simulink model "aurora_cpu_ch0_ver2_rtxsg"  (R2019b)
(part 2 of 4)

      link override Hardware Config: Controller=Xilinx VC707 Development Platform  Chassis=FlatIO  Slot1_Carrier=<empty>  Slot1_MezzA=<Empty>  Slot1_MezzB=<Empty>  Slot1_MezzC=<Empty>  Slot1_MezzD=<Empty>  Slot1_MezzE=<Empty>  Slot1_MezzF=<Empty>  Slot1_MezzG=<Empty>  Slot1_MezzH=<Empty>  Slot2_Carrier=<empty>  Slot2_MezzA=<unavailable>  Slot2_MezzB=<unavailable>  Slot3_Carrier=<empty>  Slot3_MezzA=<unavailable>  Slot3_MezzB=<unavailable>  Slot4_Carrier=<empty>  Slot4_MezzA=<unavailable>  Slot4_MezzB=<unavailable>  Slot5_Carrier=<empty>  Slot5_MezzA=<unavailable>  Slot5_MezzB=<unavailable>  Slot6_Carrier=<empty>  Slot6_MezzA=<unavailable>  Slot6_MezzB=<unavailable>  Slot7_Carrier=<empty>  Slot7_MezzA=<unavailable>  Slot7_MezzB=<unavailable>  Slot8_Carrier=<empty>  Slot8_MezzA=<unavailable>  Slot8_MezzB=<unavailable>  Slot9_Carrier=<empty>  Slot9_MezzA=<unavailable>  Slot9_MezzB=<unavailable>  Slot10_Carrier=<empty>  Slot10_MezzA=<unavailable>  Slot10_MezzB=<unavailable>  Slot11_Carrier=<empty>  Slot11_MezzA=<unavailable>  Slot11_MezzB=<unavailable>  Slot12_Carrier=<empty>  Slot12_MezzA=<unavailable>  Slot12_MezzB=<unavailable>  Slot13_Carrier=<empty>  Slot13_MezzA=<unavailable>  Slot13_MezzB=<unavailable>  Slot14_Carrier=<empty>  Slot14_MezzA=<unavailable>  Slot14_MezzB=<unavailable>  Slot15_Carrier=<empty>  Slot15_MezzA=<unavailable>  Slot15_MezzB=<unavailable>  Slot16_Carrier=<empty>  Slot16_MezzA=<unavailable>  Slot16_MezzB=<unavailable>  ExpansionSlot1A=<unavailable>  ExpansionSlot1B=<unavailable>  ExpansionSlot1C=<unavailable>  ExpansionSlot1D=<unavailable>  ExpansionSlot1E=<unavailable>  ExpansionSlot1F=<unavailable>  ExpansionSlot1G=<unavailable>  ExpansionSlot1H=<unavailable>  ExpansionSlot2A=<unavailable>  ExpansionSlot2B=<unavailable>  ExpansionSlot3A=<unavailable>  ExpansionSlot3B=<unavailable>  ExpansionSlot4A=<unavailable>  ExpansionSlot4B=<unavailable>  ExpansionSlot5A=<unavailable>  ExpansionSlot5B=<unavailable>  ExpansionSlot6A=<unavailable>  ExpansionSlot6B=<unavailable>  ExpansionSlot7A=<unavailable>  ExpansionSlot7B=<unavailable>  ExpansionSlot8A=<unavailable>  ExpansionSlot8B=<unavailable>  ExpansionSlot9A=<unavailable>  ExpansionSlot9B=<unavailable>  ExpansionSlot10A=<unavailable>  ExpansionSlot10B=<unavailable>  ExpansionSlot11A=<unavailable>  ExpansionSlot11B=<unavailable>  ExpansionSlot12A=<unavailable>  ExpansionSlot12B=<unavailable>  ExpansionSlot13A=<unavailable>  ExpansionSlot13B=<unavailable>  ExpansionSlot14A=<unavailable>  ExpansionSlot14B=<unavailable>  ExpansionSlot15A=<unavailable>  ExpansionSlot15B=<unavailable>  ExpansionSlot16A=<unavailable>  ExpansionSlot16B=<unavailable>  Slot_DV_16A="{\"dv_16A\":{\"ch0\":{\"PauseBehavior\":\"0\",\"IdleBehavior\":\"0\",\"DefaultValueReg\":\"0\"},\"ch1\":{\"PauseBehavior\":\"0\",\"IdleBehavior\":\"0\",\"DefaultValueReg\":\"0\"},\"ch2\":{\"PauseBehavior\":\"0\",\"IdleBehavior\":\"0\",\"DefaultValueReg\":\"0\"},\"ch3\":{\"PauseBehavior\":\"0\",\"IdleBehavior\":\"0\",\"DefaultValueReg\":\"0\"},\"ch4\":{\"PauseBehavior\":\"0\",\"IdleBehavior\":\"0\",\"DefaultValueReg\":\"0\"},\"ch5\":{\"PauseBehavior\":\"0\",\"IdleBehavior\":\"0\",\"DefaultValueReg\":\"0\"},\"ch6\":{\"PauseBehavior\":\"0\",\"IdleBehavior\":\"0\",\"DefaultValueReg\":\"0\"},\"ch7\":{\"PauseBehavior\":\"0\",\"IdleBehavior\":\"0\",\"DefaultValueReg\":\"0\"},\"ch8\":{\"PauseBehavior\":\"0\",\"IdleBehavior\":\"0\",\"DefaultValueReg\":\"0\"},\"ch9\":{\"PauseBehavior\":\"0\",\"IdleBehavior\":\"0\",\"DefaultValueReg\":\"0\"},\"ch10\":{\"PauseBehavior\":\"0\",\"IdleBehavior\":\"0\",\"DefaultValueReg\":\"0\"},\"ch11\":{\"PauseBehavior\":\"0\",\"IdleBehavior\":\"0\",\"DefaultValueReg\":\"0\"},\"ch12\":{\"PauseBehavior\":\"0\",\"IdleBehavior\":\"0\",\"DefaultValueReg\":\"0\"},\"ch13\":{\"PauseBehavior\":\"0\",\"IdleBehavior\":\"0\",\"DefaultValueReg\":\"0\"},\"ch14\":{\"PauseBehavior\":\"0\",\"IdleBehavior\":\"0\",\"DefaultValueReg\":\"0\"},\"ch15\":{\"PauseBehavior\":\"0\",\"IdleBehavior\":\"0\",\"DefaultValueReg\":\"0\"},\"ch16\":{\"PauseBehavior\":\"0\",\"IdleBehavior\":\"0\",\"DefaultValueReg\":\"0\"},\"ch17\":{\"PauseBehavior\":\"0\",\"IdleBehavior\":\"0\",\"DefaultValueReg\":\"0\"},\"ch18\":{\"PauseBehavior\":\"0\",\"IdleBehavior\":\"0\",\"DefaultValueReg\":\"0\"},\"ch19\":{\"PauseBehavior\":\"0\",\"IdleBehavior\":\"0\",\"DefaultValueReg\":\"0\"},\"ch20\":{\"PauseBehavior\":\"0\",\"IdleBehavior\":\"0\",\"DefaultValueReg\":\"0\"},\"ch21\":{\"PauseBehavior\":\"0\",\"IdleBehavior\":\"0\",\"DefaultValueReg\":\"0\"},\"ch22\":{\"PauseBehavior\":\"0\",\"IdleBehavior\":\"0\",\"DefaultValueReg\":\"0\"},\"ch23\":{\"PauseBehavior\":\"0\",\"IdleBehavior\":\"0\",\"DefaultValueReg\":\"0\"},\"ch24\":{\"PauseBehavior\":\"0\",\"IdleBehavior\":\"0\",\"DefaultValueReg\":\"0\"},\"ch25\":{\"PauseBehavior\":\"0\",\"IdleBehavior\":\"0\",\"DefaultValueReg\":\"0\"},\"ch26\":{\"PauseBehavior\":\"0\",\"IdleBehavior\":\"0\",\"DefaultValueReg\":\"0\"},\"ch27\":{\"PauseBehavior\":\"0\",\"IdleBehavior\":\"0\",\"DefaultValueReg\":\"0\"},\"ch28\":{\"PauseBehavior\":\"0\",\"IdleBehavior\":\"0\",\"DefaultValueReg\":\"0\"},\"ch29\":{\"PauseBehavior\":\"0\",\"IdleBehavior\":\"0\",\"DefaultValueReg\":\"0\"},\"ch30\":{\"PauseBehavior\":\"0\",\"IdleBehavior\":\"0\",\"DefaultValueReg\":\"0\"},\"ch31\":{\"PauseBehavior\":\"0\",\"IdleBehavior\":\"0\",\"DefaultValueReg\":\"0\"}}}"  Slot_DV_16B="{\"dv_16B\":{\"ch0\":{\"PauseBehavior\":\"0\",\"IdleBehavior\":\"0\",\"DefaultValueReg\":\"0\"},\"ch1\":{\"PauseBehavior\":\"0\",\"IdleBehavior\":\"0\",\"DefaultValueReg\":\"0\"},\"ch2\":{\"PauseBehavior\":\"0\",\"IdleBehavior\":\"0\",\"DefaultValueReg\":\"0\"},\"ch3\":{\"PauseBehavior\":\"0\",\"IdleBehavior\":\"0\",\"DefaultValueReg\":\"0\"},\"ch4\":{\"PauseBehavior\":\"0\",\"IdleBehavior\":\"0\",\"DefaultValueReg\":\"0\"},\"ch5\":{\"PauseBehavior\":\"0\",\"IdleBehavior\":\"0\",\"DefaultValueReg\":\"0\"},\"ch6\":{\"PauseBehavior\":\"0\",\"IdleBehavior\":\"0\",\"DefaultValueReg\":\"0\"},\"ch7\":{\"PauseBehavior\":\"0\",\"IdleBehavior\":\"0\",\"DefaultValueReg\":\"0\"},\"ch8\":{\"PauseBehavior\":\"0\",\"IdleBehavior\":\"0\",\"DefaultValueReg\":\"0\"},\"ch9\":{\"PauseBehavior\":\"0\",\"IdleBehavior\":\"0\",\"DefaultValueReg\":\"0\"},\"ch10\":{\"PauseBehavior\":\"0\",\"IdleBehavior\":\"0\",\"DefaultValueReg\":\"0\"},\"ch11\":{\"PauseBehavior\":\"0\",\"IdleBehavior\":\"0\",\"DefaultValueReg\":\"0\"},\"ch12\":{\"PauseBehavior\":\"0\",\"IdleBehavior\":\"0\",\"DefaultValueReg\":\"0\"},\"ch13\":{\"PauseBehavior\":\"0\",\"IdleBehavior\":\"0\",\"DefaultValueReg\":\"0\"},\"ch14\":{\"PauseBehavior\":\"0\",\"IdleBehavior\":\"0\",\"DefaultValueReg\":\"0\"},\"ch15\":{\"PauseBehavior\":\"0\",\"IdleBehavior\":\"0\",\"DefaultValueReg\":\"0\"},\"ch16\":{\"PauseBehavior\":\"0\",\"IdleBehavior\":\"0\",\"DefaultValueReg\":\"0\"},\"ch17\":{\"PauseBehavior\":\"0\",\"IdleBehavior\":\"0\",\"DefaultValueReg\":\"0\"},\"ch18\":{\"PauseBehavior\":\"0\",\"IdleBehavior\":\"0\",\"DefaultValueReg\":\"0\"},\"ch19\":{\"PauseBehavior\":\"0\",\"IdleBehavior\":\"0\",\"DefaultValueReg\":\"0\"},\"ch20\":{\"PauseBehavior\":\"0\",\"IdleBehavior\":\"0\",\"DefaultValueReg\":\"0\"},\"ch21\":{\"PauseBehavior\":\"0\",\"IdleBehavior\":\"0\",\"DefaultValueReg\":\"0\"},\"ch22\":{\"PauseBehavior\":\"0\",\"IdleBehavior\":\"0\",\"DefaultValueReg\":\"0\"},\"ch23\":{\"PauseBehavior\":\"0\",\"IdleBehavior\":\"0\",\"DefaultValueReg\":\"0\"},\"ch24\":{\"PauseBehavior\":\"0\",\"IdleBehavior\":\"0\",\"DefaultValueReg\":\"0\"},\"ch25\":{\"PauseBehavior\":\"0\",\"IdleBehavior\":\"0\",\"DefaultValueReg\":\"0\"},\"ch26\":{\"PauseBehavior\":\"0\",\"IdleBehavior\":\"0\",\"DefaultValueReg\":\"0\"},\"ch27\":{\"PauseBehavior\":\"0\",\"IdleBehavior\":\"0\",\"DefaultValueReg\":\"0\"},\"ch28\":{\"PauseBehavior\":\"0\",\"IdleBehavior\":\"0\",\"DefaultValueReg\":\"0\"},\"ch29\":{\"PauseBehavior\":\"0\",\"IdleBehavior\":\"0\",\"DefaultValueReg\":\"0\"},\"ch30\":{\"PauseBehavior\":\"0\",\"IdleBehavior\":\"0\",\"DefaultValueReg\":\"0\"},\"ch31\":{\"PauseBehavior\":\"0\",\"IdleBehavior\":\"0\",\"DefaultValueReg\":\"0\"}}}"  Expansion_DV_16A="{\"dv_Expansion_16A\":{\"ch0\":{\"PauseBehavior\":\"0\",\"IdleBehavior\":\"0\",\"DefaultValueReg\":\"0\"},\"ch1\":{\"PauseBehavior\":\"0\",\"IdleBehavior\":\"0\",\"DefaultValueReg\":\"0\"},\"ch2\":{\"PauseBehavior\":\"0\",\"IdleBehavior\":\"0\",\"DefaultValueReg\":\"0\"},\"ch3\":{\"PauseBehavior\":\"0\",\"IdleBehavior\":\"0\",\"DefaultValueReg\":\"0\"},\"ch4\":{\"PauseBehavior\":\"0\",\"IdleBehavior\":\"0\",\"DefaultValueReg\":\"0\"},\"ch5\":{\"PauseBehavior\":\"0\",\"IdleBehavior\":\"0\",\"DefaultValueReg\":\"0\"},\"ch6\":{\"PauseBehavior\":\"0\",\"IdleBehavior\":\"0\",\"DefaultValueReg\":\"0\"},\"ch7\":{\"PauseBehavior\":\"0\",\"IdleBehavior\":\"0\",\"DefaultValueReg\":\"0\"},\"ch8\":{\"PauseBehavior\":\"0\",\"IdleBehavior\":\"0\",\"DefaultValueReg\":\"0\"},\"ch9\":{\"PauseBehavior\":\"0\",\"IdleBehavior\":\"0\",\"DefaultValueReg\":\"0\"},\"ch10\":{\"PauseBehavior\":\"0\",\"IdleBehavior\":\"0\",\"DefaultValueReg\":\"0\"},\"ch11\":{\"PauseBehavior\":\"0\",\"IdleBehavior\":\"0\",\"DefaultValueReg\":\"0\"},\"ch12\":{\"PauseBehavior\":\"0\",\"IdleBehavior\":\"0\",\"DefaultValueReg\":\"0\"},\"ch13\":{\"PauseBehavior\":\"0\",\"IdleBehavior\":\"0\",\"DefaultValueReg\":\"0\"},\"ch14\":{\"PauseBehavior\":\"0\",\"IdleBehavior\":\"0\",\"DefaultValueReg\":\"0\"},\"ch15\":{\"PauseBehavior\":\"0\",\"IdleBehavior\":\"0\",\"DefaultValueReg\":\"0\"},\"ch16\":{\"PauseBehavior\":\"0\",\"IdleBehavior\":\"0\",\"DefaultValueReg\":\"0\"},\"ch17\":{\"PauseBehavior\":\"0\",\"IdleBehavior\":\"0\",\"DefaultValueReg\":\"0\"},\"ch18\":{\"PauseBehavior\":\"0\",\"IdleBehavior\":\"0\",\"DefaultValueReg\":\"0\"},\"ch19\":{\"PauseBehavior\":\"0\",\"IdleBehavior\":\"0\",\"DefaultValueReg\":\"0\"},\"ch20\":{\"PauseBehavior\":\"0\",\"IdleBehavior\":\"0\",\"DefaultValueReg\":\"0\"},\"ch21\":{\"PauseBehavior\":\"0\",\"IdleBehavior\":\"0\",\"DefaultValueReg\":\"0\"},\"ch22\":{\"PauseBehavior\":\"0\",\"IdleBehavior\":\"0\",\"DefaultValueReg\":\"0\"},\"ch23\":{\"PauseBehavior\":\"0\",\"IdleBehavior\":\"0\",\"DefaultValueReg\":\"0\"},\"ch24\":{\"PauseBehavior\":\"0\",\"IdleBehavior\":\"0\",\"DefaultValueReg\":\"0\"},\"ch25\":{\"PauseBehavior\":\"0\",\"IdleBehavior\":\"0\",\"DefaultValueReg\":\"0\"},\"ch26\":{\"PauseBehavior\":\"0\",\"IdleBehavior\":\"0\",\"DefaultValueReg\":\"0\"},\"ch27\":{\"PauseBehavior\":\"0\",\"IdleBehavior\":\"0\",\"DefaultValueReg\":\"0\"},\"ch28\":{\"PauseBehavior\":\"0\",\"IdleBehavior\":\"0\",\"DefaultValueReg\":\"0\"},\"ch29\":{\"PauseBehavior\":\"0\",\"IdleBehavior\":\"0\",\"DefaultValueReg\":\"0\"},\"ch30\":{\"PauseBehavior\":\"0\",\"IdleBehavior\":\"0\",\"DefaultValueReg\":\"0\"},\"ch31\":{\"PauseBehavior\":\"0\",\"IdleBehavior\":\"0\",\"DefaultValueReg\":\"0\"}}}"  Expansion_DV_16B="{\"dv_Expansion_16B\":{\"ch0\":{\"PauseBehavior\":\"0\",\"IdleBehavior\":\"0\",\"DefaultValueReg\":\"0\"},\"ch1\":{\"PauseBehavior\":\"0\",\"IdleBehavior\":\"0\",\"DefaultValueReg\":\"0\"},\"ch2\":{\"PauseBehavior\":\"0\",\"IdleBehavior\":\"0\",\"DefaultValueReg\":\"0\"},\"ch3\":{\"PauseBehavior\":\"0\",\"IdleBehavior\":\"0\",\"DefaultValueReg\":\"0\"},\"ch4\":{\"PauseBehavior\":\"0\",\"IdleBehavior\":\"0\",\"DefaultValueReg\":\"0\"},\"ch5\":{\"PauseBehavior\":\"0\",\"IdleBehavior\":\"0\",\"DefaultValueReg\":\"0\"},\"ch6\":{\"PauseBehavior\":\"0\",\"IdleBehavior\":\"0\",\"DefaultValueReg\":\"0\"},\"ch7\":{\"PauseBehavior\":\"0\",\"IdleBehavior\":\"0\",\"DefaultValueReg\":\"0\"},\"ch8\":{\"PauseBehavior\":\"0\",\"IdleBehavior\":\"0\",\"DefaultValueReg\":\"0\"},\"ch9\":{\"PauseBehavior\":\"0\",\"IdleBehavior\":\"0\",\"DefaultValueReg\":\"0\"},\"ch10\":{\"PauseBehavior\":\"0\",\"IdleBehavior\":\"0\",\"DefaultValueReg\":\"0\"},\"ch11\":{\"PauseBehavior\":\"0\",\"IdleBehavior\":\"0\",\"DefaultValueReg\":\"0\"},\"ch12\":{\"PauseBehavior\":\"0\",\"IdleBehavior\":\"0\",\"DefaultValueReg\":\"0\"},\"ch13\":{\"PauseBehavior\":\"0\",\"IdleBehavior\":\"0\",\"DefaultValueReg\":\"0\"},\"ch14\":{\"PauseBehavior\":\"0\",\"IdleBehavior\":\"0\",\"DefaultValueReg\":\"0\"},\"ch15\":{\"PauseBehavior\":\"0\",\"IdleBehavior\":\"0\",\"DefaultValueReg\":\"0\"},\"ch16\":{\"PauseBehavior\":\"0\",\"IdleBehavior\":\"0\",\"DefaultValueReg\":\"0\"},\"ch17\":{\"PauseBehavior\":\"0\",\"IdleBehavior\":\"0\",\"DefaultValueReg\":\"0\"},\"ch18\":{\"PauseBehavior\":\"0\",\"IdleBehavior\":\"0\",\"DefaultValueReg\":\"0\"},\"ch19\":{\"PauseBehavior\":\"0\",\"IdleBehavior\":\"0\",\"DefaultValueReg\":\"0\"},\"ch20\":{\"PauseBehavior\":\"0\",\"IdleBehavior\":\"0\",\"DefaultValueReg\":\"0\"},\"ch21\":{\"PauseBehavior\":\"0\",\"IdleBehavior\":\"0\",\"DefaultValueReg\":\"0\"},\"ch22\":{\"PauseBehavior\":\"0\",\"IdleBehavior\":\"0\",\"DefaultValueReg\":\"0\"},\"ch23\":{\"PauseBehavior\":\"0\",\"IdleBehavior\":\"0\",\"DefaultValueReg\":\"0\"},\"ch24\":{\"PauseBehavior\":\"0\",\"IdleBehavior\":\"0\",\"DefaultValueReg\":\"0\"},\"ch25\":{\"PauseBehavior\":\"0\",\"IdleBehavior\":\"0\",\"DefaultValueReg\":\"0\"},\"ch26\":{\"PauseBehavior\":\"0\",\"IdleBehavior\":\"0\",\"DefaultValueReg\":\"0\"},\"ch27\":{\"PauseBehavior\":\"0\",\"IdleBehavior\":\"0\",\"DefaultValueReg\":\"0\"},\"ch28\":{\"PauseBehavior\":\"0\",\"IdleBehavior\":\"0\",\"DefaultValueReg\":\"0\"},\"ch29\":{\"PauseBehavior\":\"0\",\"IdleBehavior\":\"0\",\"DefaultValueReg\":\"0\"},\"ch30\":{\"PauseBehavior\":\"0\",\"IdleBehavior\":\"0\",\"DefaultValueReg\":\"0\"},\"ch31\":{\"PauseBehavior\":\"0\",\"IdleBehavior\":\"0\",\"DefaultValueReg\":\"0\"}}}"  Slot_DV_15A="{\"dv_15A\":{\"ch0\":{\"PauseBehavior\":\"0\",\"IdleBehavior\":\"0\",\"DefaultValueReg\":\"0\"},\"ch1\":{\"PauseBehavior\":\"0\",\"IdleBehavior\":\"0\",\"DefaultValueReg\":\"0\"},\"ch2\":{\"PauseBehavior\":\"0\",\"IdleBehavior\":\"0\",\"DefaultValueReg\":\"0\"},\"ch3\":{\"PauseBehavior\":\"0\",\"IdleBehavior\":\"0\",\"DefaultValueReg\":\"0\"},\"ch4\":{\"PauseBehavior\":\"0\",\"IdleBehavior\":\"0\",\"DefaultValueReg\":\"0\"},\"ch5\":{\"PauseBehavior\":\"0\",\"IdleBehavior\":\"0\",\"DefaultValueReg\":\"0\"},\"ch6\":{\"PauseBehavior\":\"0\",\"IdleBehavior\":\"0\",\"DefaultValueReg\":\"0\"},\"ch7\":{\"PauseBehavior\":\"0\",\"IdleBehavior\":\"0\",\"DefaultValueReg\":\"0\"},\"ch8\":{\"PauseBehavior\":\"0\",\"IdleBehavior\":\"0\",\"DefaultValueReg\":\"0\"},\"ch9\":{\"PauseBehavior\":\"0\",\"IdleBehavior\":\"0\",\"DefaultValueReg\":\"0\"},\"ch10\":{\"PauseBehavior\":\"0\",\"IdleBehavior\":\"0\",\"DefaultValueReg\":\"0\"},\"ch11\":{\"PauseBehavior\":\"0\",\"IdleBehavior\":\"0\",\"DefaultValueReg\":\"0\"},\"ch12\":{\"PauseBehavior\":\"0\",\"IdleBehavior\":\"0\",\"DefaultValueReg\":\"0\"},\"ch13\":{\"PauseBehavior\":\"0\",\"IdleBehavior\":\"0\",\"DefaultValueReg\":\"0\"},\"ch14\":{\"PauseBehavior\":\"0\",\"IdleBehavior\":\"0\",\"DefaultValueReg\":\"0\"},\"ch15\":{\"PauseBehavior\":\"0\",\"IdleBehavior\":\"0\",\"DefaultValueReg\":\"0\"},\"ch16\":{\"PauseBehavior\":\"0\",\"IdleBehavior\":\"0\",\"DefaultValueReg\":\"0\"},\"ch17\":{\"PauseBehavior\":\"0\",\"IdleBehavior\":\"0\",\"DefaultValueReg\":\"0\"},\"ch18\":{\"PauseBehavior\":\"0\",\"IdleBehavior\":\"0\",\"DefaultValueReg\":\"0\"},\"ch19\":{\"PauseBehavior\":\"0\",\"IdleBehavior\":\"0\",\"DefaultValueReg\":\"0\"},\"ch20\":{\"PauseBehavior\":\"0\",\"IdleBehavior\":\"0\",\"DefaultValueReg\":\"0\"},\"ch21\":{\"PauseBehavior\":\"0\",\"IdleBehavior\":\"0\",\"DefaultValueReg\":\"0\"},\"ch22\":{\"PauseBehavior\":\"0\",\"IdleBehavior\":\"0\",\"DefaultValueReg\":\"0\"},\"ch23\":{\"PauseBehavior\":\"0\",\"IdleBehavior\":\"0\",\"DefaultValueReg\":\"0\"},\"ch24\":{\"PauseBehavior\":\"0\",\"IdleBehavior\":\"0\",\"DefaultValueReg\":\"0\"},\"ch25\":{\"PauseBehavior\":\"0\",\"IdleBehavior\":\"0\",\"DefaultValueReg\":\"0\"},\"ch26\":{\"PauseBehavior\":\"0\",\"IdleBehavior\":\"0\",\"DefaultValueReg\":\"0\"},\"ch27\":{\"PauseBehavior\":\"0\",\"IdleBehavior\":\"0\",\"DefaultValueReg\":\"0\"},\"ch28\":{\"PauseBehavior\":\"0\",\"IdleBehavior\":\"0\",\"DefaultValueReg\":\"0\"},\"ch29\":{\"PauseBehavior\":\"0\",\"IdleBehavior\":\"0\",\"DefaultValueReg\":\"0\"},\"ch30\":{\"PauseBehavior\":\"0\",\"IdleBehavior\":\"0\",\"DefaultValueReg\":\"0\"},\"ch31\":{\"PauseBehavior\":\"0\",\"IdleBehavior\":\"0\",\"DefaultValueReg\":\"0\"}}}"  Slot_DV_15B="{\"dv_15B\":{\"ch0\":{\"PauseBehavior\":\"0\",\"IdleBehavior\":\"0\",\"DefaultValueReg\":\"0\"},\"ch1\":{\"PauseBehavior\":\"0\",\"IdleBehavior\":\"0\",\"DefaultValueReg\":\"0\"},\"ch2\":{\"PauseBehavior\":\"0\",\"IdleBehavior\":\"0\",\"DefaultValueReg\":\"0\"},\"ch3\":{\"PauseBehavior\":\"0\",\"IdleBehavior\":\"0\",\"DefaultValueReg\":\"0\"},\"ch4\":{\"PauseBehavior\":\"0\",\"IdleBehavior\":\"0\",\"DefaultValueReg\":\"0\"},\"ch5\":{\"PauseBehavior\":\"0\",\"IdleBehavior\":\"0\",\"DefaultValueReg\":\"0\"},\"ch6\":{\"PauseBehavior\":\"0\",\"IdleBehavior\":\"0\",\"DefaultValueReg\":\"0\"},\"ch7\":{\"PauseBehavior\":\"0\",\"IdleBehavior\":\"0\",\"DefaultValueReg\":\"0\"},\"ch8\":{\"PauseBehavior\":\"0\",\"IdleBehavior\":\"0\",\"DefaultValueReg\":\"0\"},\"ch9\":{\"PauseBehavior\":\"0\",\"IdleBehavior\":\"0\",\"DefaultValueReg\":\"0\"},\"ch10\":{\"PauseBehavior\":\"0\",\"IdleBehavior\":\"0\",\"DefaultValueReg\":\"0\"},\"ch11\":{\"PauseBehavior\":\"0\",\"IdleBehavior\":\"0\",\"DefaultValueReg\":\"0\"},\"ch12\":{\"PauseBehavior\":\"0\",\"IdleBehavior\":\"0\",\"DefaultValueReg\":\"0\"},\"ch13\":{\"PauseBehavior\":\"0\",\"IdleBehavior\":\"0\",\"DefaultValueReg\":\"0\"},\"ch14\":{\"PauseBehavior\":\"0\",\"IdleBehavior\":\"0\",\"DefaultValueReg\":\"0\"},\"ch15\":{\"PauseBehavior\":\"0\",\"IdleBehavior\":\"0\",\"DefaultValueReg\":\"0\"},\"ch16\":{\"PauseBehavior\":\"0\",\"IdleBehavior\":\"0\",\"DefaultValueReg\":\"0\"},\"ch17\":{\"PauseBehavior\":\"0\",\"IdleBehavior\":\"0\",\"DefaultValueReg\":\"0\"},\"ch18\":{\"PauseBehavior\":\"0\",\"IdleBehavior\":\"0\",\"DefaultValueReg\":\"0\"},\"ch19\":{\"PauseBehavior\":\"0\",\"IdleBehavior\":\"0\",\"DefaultValueReg\":\"0\"},\"ch20\":{\"PauseBehavior\":\"0\",\"IdleBehavior\":\"0\",\"DefaultValueReg\":\"0\"},\"ch21\":{\"PauseBehavior\":\"0\",\"IdleBehavior\":\"0\",\"DefaultValueReg\":\"0\"},\"ch22\":{\"PauseBehavior\":\"0\",\"IdleBehavior\":\"0\",\"DefaultValueReg\":\"0\"},\"ch23\":{\"PauseBehavior\":\"0\",\"IdleBehavior\":\"0\",\"DefaultValueReg\":\"0\"},\"ch24\":{\"PauseBehavior\":\"0\",\"IdleBehavior\":\"0\",\"DefaultValueReg\":\"0\"},\"ch25\":{\"PauseBehavior\":\"0\",\"IdleBehavior\":\"0\",\"DefaultValueReg\":\"0\"},\"ch26\":{\"PauseBehavior\":\"0\",\"IdleBehavior\":\"0\",\"DefaultValueReg\":\"0\"},\"ch27\":{\"PauseBehavior\":\"0\",\"IdleBehavior\":\"0\",\"DefaultValueReg\":\"0\"},\"ch28\":{\"PauseBehavior\":\"0\",\"IdleBehavior\":\"0\",\"DefaultValueReg\":\"0\"},\"ch29\":{\"PauseBehavior\":\"0\",\"IdleBehavior\":\"0\",\"DefaultValueReg\":\"0\"},\"ch30\":{\"PauseBehavior\":\"0\",\"IdleBehavior\":\"0\",\"DefaultValueReg\":\"0\"},\"ch31\":{\"PauseBehavior\":\"0\",\"IdleBehavior\":\"0\",\"DefaultValueReg\":\"0\"}}}"  Expansion_DV_15A="{\"dv_Expansion_15A\":{\"ch0\":{\"PauseBehavior\":\"0\",\"IdleBehavior\":\"0\",\"DefaultValueReg\":\"0\"},\"ch1\":{\"PauseBehavior\":\"0\",\"IdleBehavior\":\"0\",\"DefaultValueReg\":\"0\"},\"ch2\":{\"PauseBehavior\":\"0\",\"IdleBehavior\":\"0\",\"DefaultValueReg\":\"0\"},\"ch3\":{\"PauseBehavior\":\"0\",\"IdleBehavior\":\"0\",\"DefaultValueReg\":\"0\"},\"ch4\":{\"PauseBehavior\":\"0\",\"IdleBehavior\":\"0\",\"DefaultValueReg\":\"0\"},\"ch5\":{\"PauseBehavior\":\"0\",\"IdleBehavior\":\"0\",\"DefaultValueReg\":\"0\"},\"ch6\":{\"PauseBehavior\":\"0\",\"IdleBehavior\":\"0\",\"DefaultValueReg\":\"0\"},\"ch7\":{\"PauseBehavior\":\"0\",\"IdleBehavior\":\"0\",\"DefaultValueReg\":\"0\"},\"ch8\":{\"PauseBehavior\":\"0\",\"IdleBehavior\":\"0\",\"DefaultValueReg\":\"0\"},\"ch9\":{\"PauseBehavior\":\"0\",\"IdleBehavior\":\"0\",\"DefaultValueReg\":\"0\"},\"ch10\":{\"PauseBehavior\":\"0\",\"IdleBehavior\":\"0\",\"DefaultValueReg\":\"0\"},\"ch11\":{\"PauseBehavior\":\"0\",\"IdleBehavior\":\"0\",\"DefaultValueReg\":\"0\"},\"ch12\":{\"PauseBehavior\":\"0\",\"IdleBehavior\":\"0\",\"DefaultValueReg\":\"0\"},\"ch13\":{\"PauseBehavior\":\"0\",\"IdleBehavior\":\"0\",\"DefaultValueReg\":\"0\"},\"ch14\":{\"PauseBehavior\":\"0\",\"IdleBehavior\":\"0\",\"DefaultValueReg\":\"0\"},\"ch15\":{\"PauseBehavior\":\"0\",\"IdleBehavior\":\"0\",\"DefaultValueReg\":\"0\"},\"ch16\":{\"PauseBehavior\":\"0\",\"IdleBehavior\":\"0\",\"DefaultValueReg\":\"0\"},\"ch17\":{\"PauseBehavior\":\"0\",\"IdleBehavior\":\"0\",\"DefaultValueReg\":\"0\"},\"ch18\":{\"PauseBehavior\":\"0\",\"IdleBehavior\":\"0\",\"DefaultValueReg\":\"0\"},\"ch19\":{\"PauseBehavior\":\"0\",\"IdleBehavior\":\"0\",\"DefaultValueReg\":\"0\"},\"ch20\":{\"PauseBehavior\":\"0\",\"IdleBehavior\":\"0\",\"DefaultValueReg\":\"0\"},\"ch21\":{\"PauseBehavior\":\"0\",\"IdleBehavior\":\"0\",\"DefaultValueReg\":\"0\"},\"ch22\":{\"PauseBehavior\":\"0\",\"IdleBehavior\":\"0\",\"DefaultValueReg\":\"0\"},\"ch23\":{\"PauseBehavior\":\"0\",\"IdleBehavior\":\"0\",\"DefaultValueReg\":\"0\"},\"ch24\":{\"PauseBehavior\":\"0\",\"IdleBehavior\":\"0\",\"DefaultValueReg\":\"0\"},\"ch25\":{\"PauseBehavior\":\"0\",\"IdleBehavior\":\"0\",\"DefaultValueReg\":\"0\"},\"ch26\":{\"PauseBehavior\":\"0\",\"IdleBehavior\":\"0\",\"DefaultValueReg\":\"0\"},\"ch27\":{\"PauseBehavior\":\"0\",\"IdleBehavior\":\"0\",\"DefaultValueReg\":\"0\"},\"ch28\":{\"PauseBehavior\":\"0\",\"IdleBehavior\":\"0\",\"DefaultValueReg\":\"0\"},\"ch29\":{\"PauseBehavior\":\"0\",\"IdleBehavior\":\"0\",\"DefaultValueReg\":\"0\"},\"ch30\":{\"PauseBehavior\":\"0\",\"IdleBehavior\":\"0\",\"DefaultValueReg\":\"0\"},\"ch31\":{\"PauseBehavior\":\"0\",\"IdleBehavior\":\"0\",\"DefaultValueReg\":\"0\"}}}"  Expansion_DV_15B="{\"dv_Expansion_15B\":{\"ch0\":{\"PauseBehavior\":\"0\",\"IdleBehavior\":\"0\",\"DefaultValueReg\":\"0\"},\"ch1\":{\"PauseBehavior\":\"0\",\"IdleBehavior\":\"0\",\"DefaultValueReg\":\"0\"},\"ch2\":{\"PauseBehavior\":\"0\",\"IdleBehavior\":\"0\",\"DefaultValueReg\":\"0\"},\"ch3\":{\"PauseBehavior\":\"0\",\"IdleBehavior\":\"0\",\"DefaultValueReg\":\"0\"},\"ch4\":{\"PauseBehavior\":\"0\",\"IdleBehavior\":\"0\",\"DefaultValueReg\":\"0\"},\"ch5\":{\"PauseBehavior\":\"0\",\"IdleBehavior\":\"0\",\"DefaultValueReg\":\"0\"},\"ch6\":{\"PauseBehavior\":\"0\",\"IdleBehavior\":\"0\",\"DefaultValueReg\":\"0\"},\"ch7\":{\"PauseBehavior\":\"0\",\"IdleBehavior\":\"0\",\"DefaultValueReg\":\"0\"},\"ch8\":{\"PauseBehavior\":\"0\",\"IdleBehavior\":\"0\",\"DefaultValueReg\":\"0\"},\"ch9\":{\"PauseBehavior\":\"0\",\"IdleBehavior\":\"0\",\"DefaultValueReg\":\"0\"},\"ch10\":{\"PauseBehavior\":\"0\",\"IdleBehavior\":\"0\",\"DefaultValueReg\":\"0\"},\"ch11\":{\"PauseBehavior\":\"0\",\"IdleBehavior\":\"0\",\"DefaultValueReg\":\"0\"},\"ch12\":{\"PauseBehavior\":\"0\",\"IdleBehavior\":\"0\",\"DefaultValueReg\":\"0\"},\"ch13\":{\"PauseBehavior\":\"0\",\"IdleBehavior\":\"0\",\"DefaultValueReg\":\"0\"},\"ch14\":{\"PauseBehavior\":\"0\",\"IdleBehavior\":\"0\",\"DefaultValueReg\":\"0\"},\"ch15\":{\"PauseBehavior\":\"0\",\"IdleBehavior\":\"0\",\"DefaultValueReg\":\"0\"},\"ch16\":{\"PauseBehavior\":\"0\",\"IdleBehavior\":\"0\",\"DefaultValueReg\":\"0\"},\"ch17\":{\"PauseBehavior\":\"0\",\"IdleBehavior\":\"0\",\"DefaultValueReg\":\"0\"},\"ch18\":{\"PauseBehavior\":\"0\",\"IdleBehavior\":\"0\",\"DefaultValueReg\":\"0\"},\"ch19\":{\"PauseBehavior\":\"0\",\"IdleBehavior\":\"0\",\"DefaultValueReg\":\"0\"},\"ch20\":{\"PauseBehavior\":\"0\",\"IdleBehavior\":\"0\",\"DefaultValueReg\":\"0\"},\"ch21\":{\"PauseBehavior\":\"0\",\"IdleBehavior\":\"0\",\"DefaultValueReg\":\"0\"},\"ch22\":{\"PauseBehavior\":\"0\",\"IdleBehavior\":\"0\",\"DefaultValueReg\":\"0\"},\"ch23\":{\"PauseBehavior\":\"0\",\"IdleBehavior\":\"0\",\"DefaultValueReg\":\"0\"},\"ch24\":{\"PauseBehavior\":\"0\",\"IdleBehavior\":\"0\",\"DefaultValueReg\":\"0\"},\"ch25\":{\"PauseBehavior\":\"0\",\"IdleBehavior\":\"0\",\"DefaultValueReg\":\"0\"},\"ch26\":{\"PauseBehavior\":\"0\",\"IdleBehavior\":\"0\",\"DefaultValueReg\":\"0\"},\"ch27\":{\"PauseBehavior\":\"0\",\"IdleBehavior\":\"0\",\"DefaultValueReg\":\"0\"},\"ch28\":{\"PauseBehavior\":\"0\",\"IdleBehavior\":\"0\",\"DefaultValueReg\":\"0\"},\"ch29\":{\"PauseBehavior\":\"0\",\"IdleBehavior\":\"0\",\"DefaultValueReg\":\"0\"},\"ch30\":{\"PauseBehavior\":\"0\",\"IdleBehavior\":\"0\",\"DefaultValueReg\":\"0\"},\"ch31\":{\"PauseBehavior\":\"0\",\"IdleBehavior\":\"0\",\"DefaultValueReg\":\"0\"}}}"  Slot_DV_14A="{\"dv_14A\":{\"ch0\":{\"PauseBehavior\":\"0\",\"IdleBehavior\":\"0\",\"DefaultValueReg\":\"0\"},\"ch1\":{\"PauseBehavior\":\"0\",\"IdleBehavior\":\"0\",\"DefaultValueReg\":\"0\"},\"ch2\":{\"PauseBehavior\":\"0\",\"IdleBehavior\":\"0\",\"DefaultValueReg\":\"0\"},\"ch3\":{\"PauseBehavior\":\"0\",\"IdleBehavior\":\"0\",\"DefaultValueReg\":\"0\"},\"ch4\":{\"PauseBehavior\":\"0\",\"IdleBehavior\":\"0\",\"DefaultValueReg\":\"0\"},\"ch5\":{\"PauseBehavior\":\"0\",\"IdleBehavior\":\"0\",\"DefaultValueReg\":\"0\"},\"ch6\":{\"PauseBehavior\":\"0\",\"IdleBehavior\":\"0\",\"DefaultValueReg\":\"0\"},\"ch7\":{\"PauseBehavior\":\"0\",\"IdleBehavior\":\"0\",\"DefaultValueReg\":\"0\"},\"ch8\":{\"PauseBehavior\":\"0\",\"IdleBehavior\":\"0\",\"DefaultValueReg\":\"0\"},\"ch9\":{\"PauseBehavior\":\"0\",\"IdleBehavior\":\"0\",\"DefaultValueReg\":\"0\"},\"ch10\":{\"PauseBehavior\":\"0\",\"IdleBehavior\":\"0\",\"DefaultValueReg\":\"0\"},\"ch11\":{\"PauseBehavior\":\"0\",\"IdleBehavior\":\"0\",\"DefaultValueReg\":\"0\"},\"ch12\":{\"PauseBehavior\":\"0\",\"IdleBehavior\":\"0\",\"DefaultValueReg\":\"0\"},\"ch13\":{\"PauseBehavior\":\"0\",\"IdleBehavior\":\"0\",\"DefaultValueReg\":\"0\"},\"ch14\":{\"PauseBehavior\":\"0\",\"IdleBehavior\":\"0\",\"DefaultValueReg\":\"0\"},\"ch15\":{\"PauseBehavior\":\"0\",\"IdleBehavior\":\"0\",\"DefaultValueReg\":\"0\"},\"ch16\":{\"PauseBehavior\":\"0\",\"IdleBehavior\":\"0\",\"DefaultValueReg\":\"0\"},\"ch17\":{\"PauseBehavior\":\"0\",\"IdleBehavior\":\"0\",\"DefaultValueReg\":\"0\"},\"ch18\":{\"PauseBehavior\":\"0\",\"IdleBehavior\":\"0\",\"DefaultValueReg\":\"0\"},\"ch19\":{\"PauseBehavior\":\"0\",\"IdleBehavior\":\"0\",\"DefaultValueReg\":\"0\"},\"ch20\":{\"PauseBehavior\":\"0\",\"IdleBehavior\":\"0\",\"DefaultValueReg\":\"0\"},\"ch21\":{\"PauseBehavior\":\"0\",\"IdleBehavior\":\"0\",\"DefaultValueReg\":\"0\"},\"ch22\":{\"PauseBehavior\":\"0\",\"IdleBehavior\":\"0\",\"DefaultValueReg\":\"0\"},\"ch23\":{\"PauseBehavior\":\"0\",\"IdleBehavior\":\"0\",\"DefaultValueReg\":\"0\"},\"ch24\":{\"PauseBehavior\":\"0\",\"IdleBehavior\":\"0\",\"DefaultValueReg\":\"0\"},\"ch25\":{\"PauseBehavior\":\"0\",\"IdleBehavior\":\"0\",\"DefaultValueReg\":\"0\"},\"ch26\":{\"PauseBehavior\":\"0\",\"IdleBehavior\":\"0\",\"DefaultValueReg\":\"0\"},\"ch27\":{\"PauseBehavior\":\"0\",\"IdleBehavior\":\"0\",\"DefaultValueReg\":\"0\"},\"ch28\":{\"PauseBehavior\":\"0\",\"IdleBehavior\":\"0\",\"DefaultValueReg\":\"0\"},\"ch29\":{\"PauseBehavior\":\"0\",\"IdleBehavior\":\"0\",\"DefaultValueReg\":\"0\"},\"ch30\":{\"PauseBehavior\":\"0\",\"IdleBehavior\":\"0\",\"DefaultValueReg\":\"0\"},\"ch31\":{\"PauseBehavior\":\"0\",\"IdleBehavior\":\"0\",\"DefaultValueReg\":\"0\"}}}"  Slot_DV_14B="{\"dv_14B\":{\"ch0\":{\"PauseBehavior\":\"0\",\"IdleBehavior\":\"0\",\"DefaultValueReg\":\"0\"},\"ch1\":{\"PauseBehavior\":\"0\",\"IdleBehavior\":\"0\",\"DefaultValueReg\":\"0\"},\"ch2\":{\"PauseBehavior\":\"0\",\"IdleBehavior\":\"0\",\"DefaultValueReg\":\"0\"},\"ch3\":{\"PauseBehavior\":\"0\",\"IdleBehavior\":\"0\",\"DefaultValueReg\":\"0\"},\"ch4\":{\"PauseBehavior\":\"0\",\"IdleBehavior\":\"0\",\"DefaultValueReg\":\"0\"},\"ch5\":{\"PauseBehavior\":\"0\",\"IdleBehavior\":\"0\",\"DefaultValueReg\":\"0\"},\"ch6\":{\"PauseBehavior\":\"0\",\"IdleBehavior\":\"0\",\"DefaultValueReg\":\"0\"},\"ch7\":{\"PauseBehavior\":\"0\",\"IdleBehavior\":\"0\",\"DefaultValueReg\":\"0\"},\"ch8\":{\"PauseBehavior\":\"0\",\"IdleBehavior\":\"0\",\"DefaultValueReg\":\"0\"},\"ch9\":{\"PauseBehavior\":\"0\",\"IdleBehavior\":\"0\",\"DefaultValueReg\":\"0\"},\"ch10\":{\"PauseBehavior\":\"0\",\"IdleBehavior\":\"0\",\"DefaultValueReg\":\"0\"},\"ch11\":{\"PauseBehavior\":\"0\",\"IdleBehavior\":\"0\",\"DefaultValueReg\":\"0\"},\"ch12\":{\"PauseBehavior\":\"0\",\"IdleBehavior\":\"0\",\"DefaultValueReg\":\"0\"},\"ch13\":{\"PauseBehavior\":\"0\",\"IdleBehavior\":\"0\",\"DefaultValueReg\":\"0\"},\"ch14\":{\"PauseBehavior\":\"0\",\"IdleBehavior\":\"0\",\"DefaultValueReg\":\"0\"},\"ch15\":{\"PauseBehavior\":\"0\",\"IdleBehavior\":\"0\",\"DefaultValueReg\":\"0\"},\"ch16\":{\"PauseBehavior\":\"0\",\"IdleBehavior\":\"0\",\"DefaultValueReg\":\"0\"},\"ch17\":{\"PauseBehavior\":\"0\",\"IdleBehavior\":\"0\",\"DefaultValueReg\":\"0\"},\"ch18\":{\"PauseBehavior\":\"0\",\"IdleBehavior\":\"0\",\"DefaultValueReg\":\"0\"},\"ch19\":{\"PauseBehavior\":\"0\",\"IdleBehavior\":\"0\",\"DefaultValueReg\":\"0\"},\"ch20\":{\"PauseBehavior\":\"0\",\"IdleBehavior\":\"0\",\"DefaultValueReg\":\"0\"},\"ch21\":{\"PauseBehavior\":\"0\",\"IdleBehavior\":\"0\",\"DefaultValueReg\":\"0\"},\"ch22\":{\"PauseBehavior\":\"0\",\"IdleBehavior\":\"0\",\"DefaultValueReg\":\"0\"},\"ch23\":{\"PauseBehavior\":\"0\",\"IdleBehavior\":\"0\",\"DefaultValueReg\":\"0\"},\"ch24\":{\"PauseBehavior\":\"0\",\"IdleBehavior\":\"0\",\"DefaultValueReg\":\"0\"},\"ch25\":{\"PauseBehavior\":\"0\",\"IdleBehavior\":\"0\",\"DefaultValueReg\":\"0\"},\"ch26\":{\"PauseBehavior\":\"0\",\"IdleBehavior\":\"0\",\"DefaultValueReg\":\"0\"},\"ch27\":{\"PauseBehavior\":\"0\",\"IdleBehavior\":\"0\",\"DefaultValueReg\":\"0\"},\"ch28\":{\"PauseBehavior\":\"0\",\"IdleBehavior\":\"0\",\"DefaultValueReg\":\"0\"},\"ch29\":{\"PauseBehavior\":\"0\",\"IdleBehavior\":\"0\",\"DefaultValueReg\":\"0\"},\"ch30\":{\"PauseBehavior\":\"0\",\"IdleBehavior\":\"0\",\"DefaultValueReg\":\"0\"},\"ch31\":{\"PauseBehavior\":\"0\",\"IdleBehavior\":\"0\",\"DefaultValueReg\":\"0\"}}}"  Expansion_DV_14A="{\"dv_Expansion_14A\":{\"ch0\":{\"PauseBehavior\":\"0\",\"IdleBehavior\":\"0\",\"DefaultValueReg\":\"0\"},\"ch1\":{\"PauseBehavior\":\"0\",\"IdleBehavior\":\"0\",\"DefaultValueReg\":\"0\"},\"ch2\":{\"PauseBehavior\":\"0\",\"IdleBehavior\":\"0\",\"DefaultValueReg\":\"0\"},\"ch3\":{\"PauseBehavior\":\"0\",\"IdleBehavior\":\"0\",\"DefaultValueReg\":\"0\"},\"ch4\":{\"PauseBehavior\":\"0\",\"IdleBehavior\":\"0\",\"DefaultValueReg\":\"0\"},\"ch5\":{\"PauseBehavior\":\"0\",\"IdleBehavior\":\"0\",\"DefaultValueReg\":\"0\"},\"ch6\":{\"PauseBehavior\":\"0\",\"IdleBehavior\":\"0\",\"DefaultValueReg\":\"0\"},\"ch7\":{\"PauseBehavior\":\"0\",\"IdleBehavior\":\"0\",\"DefaultValueReg\":\"0\"},\"ch8\":{\"PauseBehavior\":\"0\",\"IdleBehavior\":\"0\",\"DefaultValueReg\":\"0\"},\"ch9\":{\"PauseBehavior\":\"0\",\"IdleBehavior\":\"0\",\"DefaultValueReg\":\"0\"},\"ch10\":{\"PauseBehavior\":\"0\",\"IdleBehavior\":\"0\",\"DefaultValueReg\":\"0\"},\"ch11\":{\"PauseBehavior\":\"0\",\"IdleBehavior\":\"0\",\"DefaultValueReg\":\"0\"},\"ch12\":{\"PauseBehavior\":\"0\",\"IdleBehavior\":\"0\",\"DefaultValueReg\":\"0\"},\"ch13\":{\"PauseBehavior\":\"0\",\"IdleBehavior\":\"0\",\"DefaultValueReg\":\"0\"},\"ch14\":{\"PauseBehavior\":\"0\",\"IdleBehavior\":\"0\",\"DefaultValueReg\":\"0\"},\"ch15\":{\"PauseBehavior\":\"0\",\"IdleBehavior\":\"0\",\"DefaultValueReg\":\"0\"},\"ch16\":{\"PauseBehavior\":\"0\",\"IdleBehavior\":\"0\",\"DefaultValueReg\":\"0\"},\"ch17\":{\"PauseBehavior\":\"0\",\"IdleBehavior\":\"0\",\"DefaultValueReg\":\"0\"},\"ch18\":{\"PauseBehavior\":\"0\",\"IdleBehavior\":\"0\",\"DefaultValueReg\":\"0\"},\"ch19\":{\"PauseBehavior\":\"0\",\"IdleBehavior\":\"0\",\"DefaultValueReg\":\"0\"},\"ch20\":{\"PauseBehavior\":\"0\",\"IdleBehavior\":\"0\",\"DefaultValueReg\":\"0\"},\"ch21\":{\"PauseBehavior\":\"0\",\"IdleBehavior\":\"0\",\"DefaultValueReg\":\"0\"},\"ch22\":{\"PauseBehavior\":\"0\",\"IdleBehavior\":\"0\",\"DefaultValueReg\":\"0\"},\"ch23\":{\"PauseBehavior\":\"0\",\"IdleBehavior\":\"0\",\"DefaultValueReg\":\"0\"},\"ch24\":{\"PauseBehavior\":\"0\",\"IdleBehavior\":\"0\",\"DefaultValueReg\":\"0\"},\"ch25\":{\"PauseBehavior\":\"0\",\"IdleBehavior\":\"0\",\"DefaultValueReg\":\"0\"},\"ch26\":{\"PauseBehavior\":\"0\",\"IdleBehavior\":\"0\",\"DefaultValueReg\":\"0\"},\"ch27\":{\"PauseBehavior\":\"0\",\"IdleBehavior\":\"0\",\"DefaultValueReg\":\"0\"},\"ch28\":{\"PauseBehavior\":\"0\",\"IdleBehavior\":\"0\",\"DefaultValueReg\":\"0\"},\"ch29\":{\"PauseBehavior\":\"0\",\"IdleBehavior\":\"0\",\"DefaultValueReg\":\"0\"},\"ch30\":{\"PauseBehavior\":\"0\",\"IdleBehavior\":\"0\",\"DefaultValueReg\":\"0\"},\"ch31\":{\"PauseBehavior\":\"0\",\"IdleBehavior\":\"0\",\"DefaultValueReg\":\"0\"}}}"  Expansion_DV_14B="{\"dv_Expansion_14B\":{\"ch0\":{\"PauseBehavior\":\"0\",\"IdleBehavior\":\"0\",\"DefaultValueReg\":\"0\"},\"ch1\":{\"PauseBehavior\":\"0\",\"IdleBehavior\":\"0\",\"DefaultValueReg\":\"0\"},\"ch2\":{\"PauseBehavior\":\"0\",\"IdleBehavior\":\"0\",\"DefaultValueReg\":\"0\"},\"ch3\":{\"PauseBehavior\":\"0\",\"IdleBehavior\":\"0\",\"DefaultValueReg\":\"0\"},\"ch4\":{\"PauseBehavior\":\"0\",\"IdleBehavior\":\"0\",\"DefaultValueReg\":\"0\"},\"ch5\":{\"PauseBehavior\":\"0\",\"IdleBehavior\":\"0\",\"DefaultValueReg\":\"0\"},\"ch6\":{\"PauseBehavior\":\"0\",\"IdleBehavior\":\"0\",\"DefaultValueReg\":\"0\"},\"ch7\":{\"PauseBehavior\":\"0\",\"IdleBehavior\":\"0\",\"DefaultValueReg\":\"0\"},\"ch8\":{\"PauseBehavior\":\"0\",\"IdleBehavior\":\"0\",\"DefaultValueReg\":\"0\"},\"ch9\":{\"PauseBehavior\":\"0\",\"IdleBehavior\":\"0\",\"DefaultValueReg\":\"0\"},\"ch10\":{\"PauseBehavior\":\"0\",\"IdleBehavior\":\"0\",\"DefaultValueReg\":\"0\"},\"ch11\":{\"PauseBehavior\":\"0\",\"IdleBehavior\":\"0\",\"DefaultValueReg\":\"0\"},\"ch12\":{\"PauseBehavior\":\"0\",\"IdleBehavior\":\"0\",\"DefaultValueReg\":\"0\"},\"ch13\":{\"PauseBehavior\":\"0\",\"IdleBehavior\":\"0\",\"DefaultValueReg\":\"0\"},\"ch14\":{\"PauseBehavior\":\"0\",\"IdleBehavior\":\"0\",\"DefaultValueReg\":\"0\"},\"ch15\":{\"PauseBehavior\":\"0\",\"IdleBehavior\":\"0\",\"DefaultValueReg\":\"0\"},\"ch16\":{\"PauseBehavior\":\"0\",\"IdleBehavior\":\"0\",\"DefaultValueReg\":\"0\"},\"ch17\":{\"PauseBehavior\":\"0\",\"IdleBehavior\":\"0\",\"DefaultValueReg\":\"0\"},\"ch18\":{\"PauseBehavior\":\"0\",\"IdleBehavior\":\"0\",\"DefaultValueReg\":\"0\"},\"ch19\":{\"PauseBehavior\":\"0\",\"IdleBehavior\":\"0\",\"DefaultValueReg\":\"0\"},\"ch20\":{\"PauseBehavior\":\"0\",\"IdleBehavior\":\"0\",\"DefaultValueReg\":\"0\"},\"ch21\":{\"PauseBehavior\":\"0\",\"IdleBehavior\":\"0\",\"DefaultValueReg\":\"0\"},\"ch22\":{\"PauseBehavior\":\"0\",\"IdleBehavior\":\"0\",\"DefaultValueReg\":\"0\"},\"ch23\":{\"PauseBehavior\":\"0\",\"IdleBehavior\":\"0\",\"DefaultValueReg\":\"0\"},\"ch24\":{\"PauseBehavior\":\"0\",\"IdleBehavior\":\"0\",\"DefaultValueReg\":\"0\"},\"ch25\":{\"PauseBehavior\":\"0\",\"IdleBehavior\":\"0\",\"DefaultValueReg\":\"0\"},\"ch26\":{\"PauseBehavior\":\"0\",\"IdleBehavior\":\"0\",\"DefaultValueReg\":\"0\"},\"ch27\":{\"PauseBehavior\":\"0\",\"IdleBehavior\":\"0\",\"DefaultValueReg\":\"0\"},\"ch28\":{\"PauseBehavior\":\"0\",\"IdleBehavior\":\"0\",\"DefaultValueReg\":\"0\"},\"ch29\":{\"PauseBehavior\":\"0\",\"IdleBehavior\":\"0\",\"DefaultValueReg\":\"0\"},\"ch30\":{\"PauseBehavior\":\"0\",\"IdleBehavior\":\"0\",\"DefaultValueReg\":\"0\"},\"ch31\":{\"PauseBehavior\":\"0\",\"IdleBehavior\":\"0\",\"DefaultValueReg\":\"0\"}}}"  Slot_DV_13A="{\"dv_13A\":{\"ch0\":{\"PauseBehavior\":\"0\",\"IdleBehavior\":\"0\",\"DefaultValueReg\":\"0\"},\"ch1\":{\"PauseBehavior\":\"0\",\"IdleBehavior\":\"0\",\"DefaultValueReg\":\"0\"},\"ch2\":{\"PauseBehavior\":\"0\",\"IdleBehavior\":\"0\",\"DefaultValueReg\":\"0\"},\"ch3\":{\"PauseBehavior\":\"0\",\"IdleBehavior\":\"0\",\"DefaultValueReg\":\"0\"},\"ch4\":{\"PauseBehavior\":\"0\",\"IdleBehavior\":\"0\",\"DefaultValueReg\":\"0\"},\"ch5\":{\"PauseBehavior\":\"0\",\"IdleBehavior\":\"0\",\"DefaultValueReg\":\"0\"},\"ch6\":{\"PauseBehavior\":\"0\",\"IdleBehavior\":\"0\",\"DefaultValueReg\":\"0\"},\"ch7\":{\"PauseBehavior\":\"0\",\"IdleBehavior\":\"0\",\"DefaultValueReg\":\"0\"},\"ch8\":{\"PauseBehavior\":\"0\",\"IdleBehavior\":\"0\",\"DefaultValueReg\":\"0\"},\"ch9\":{\"PauseBehavior\":\"0\",\"IdleBehavior\":\"0\",\"DefaultValueReg\":\"0\"},\"ch10\":{\"PauseBehavior\":\"0\",\"IdleBehavior\":\"0\",\"DefaultValueReg\":\"0\"},\"ch11\":{\"PauseBehavior\":\"0\",\"IdleBehavior\":\"0\",\"DefaultValueReg\":\"0\"},\"ch12\":{\"PauseBehavior\":\"0\",\"IdleBehavior\":\"0\",\"DefaultValueReg\":\"0\"},\"ch13\":{\"PauseBehavior\":\"0\",\"IdleBehavior\":\"0\",\"DefaultValueReg\":\"0\"},\"ch14\":{\"PauseBehavior\":\"0\",\"IdleBehavior\":\"0\",\"DefaultValueReg\":\"0\"},\"ch15\":{\"PauseBehavior\":\"0\",\"IdleBehavior\":\"0\",\"DefaultValueReg\":\"0\"},\"ch16\":{\"PauseBehavior\":\"0\",\"IdleBehavior\":\"0\",\"DefaultValueReg\":\"0\"},\"ch17\":{\"PauseBehavior\":\"0\",\"IdleBehavior\":\"0\",\"DefaultValueReg\":\"0\"},\"ch18\":{\"PauseBehavior\":\"0\",\"IdleBehavior\":\"0\",\"DefaultValueReg\":\"0\"},\"ch19\":{\"PauseBehavior\":\"0\",\"IdleBehavior\":\"0\",\"DefaultValueReg\":\"0\"},\"ch20\":{\"PauseBehavior\":\"0\",\"IdleBehavior\":\"0\",\"DefaultValueReg\":\"0\"},\"ch21\":{\"PauseBehavior\":\"0\",\"IdleBehavior\":\"0\",\"DefaultValueReg\":\"0\"},\"ch22\":{\"PauseBehavior\":\"0\",\"IdleBehavior\":\"0\",\"DefaultValueReg\":\"0\"},\"ch23\":{\"PauseBehavior\":\"0\",\"IdleBehavior\":\"0\",\"DefaultValueReg\":\"0\"},\"ch24\":{\"PauseBehavior\":\"0\",\"IdleBehavior\":\"0\",\"DefaultValueReg\":\"0\"},\"ch25\":{\"PauseBehavior\":\"0\",\"IdleBehavior\":\"0\",\"DefaultValueReg\":\"0\"},\"ch26\":{\"PauseBehavior\":\"0\",\"IdleBehavior\":\"0\",\"DefaultValueReg\":\"0\"},\"ch27\":{\"PauseBehavior\":\"0\",\"IdleBehavior\":\"0\",\"DefaultValueReg\":\"0\"},\"ch28\":{\"PauseBehavior\":\"0\",\"IdleBehavior\":\"0\",\"DefaultValueReg\":\"0\"},\"ch29\":{\"PauseBehavior\":\"0\",\"IdleBehavior\":\"0\",\"DefaultValueReg\":\"0\"},\"ch30\":{\"PauseBehavior\":\"0\",\"IdleBehavior\":\"0\",\"DefaultValueReg\":\"0\"},\"ch31\":{\"PauseBehavior\":\"0\",\"IdleBehavior\":\"0\",\"DefaultValueReg\":\"0\"}}}"  Slot_DV_13B="{\"dv_13B\":{\"ch0\":{\"PauseBehavior\":\"0\",\"IdleBehavior\":\"0\",\"DefaultValueReg\":\"0\"},\"ch1\":{\"PauseBehavior\":\"0\",\"IdleBehavior\":\"0\",\"DefaultValueReg\":\"0\"},\"ch2\":{\"PauseBehavior\":\"0\",\"IdleBehavior\":\"0\",\"DefaultValueReg\":\"0\"},\"ch3\":{\"PauseBehavior\":\"0\",\"IdleBehavior\":\"0\",\"DefaultValueReg\":\"0\"},\"ch4\":{\"PauseBehavior\":\"0\",\"IdleBehavior\":\"0\",\"DefaultValueReg\":\"0\"},\"ch5\":{\"PauseBehavior\":\"0\",\"IdleBehavior\":\"0\",\"DefaultValueReg\":\"0\"},\"ch6\":{\"PauseBehavior\":\"0\",\"IdleBehavior\":\"0\",\"DefaultValueReg\":\"0\"},\"ch7\":{\"PauseBehavior\":\"0\",\"IdleBehavior\":\"0\",\"DefaultValueReg\":\"0\"},\"ch8\":{\"PauseBehavior\":\"0\",\"IdleBehavior\":\"0\",\"DefaultValueReg\":\"0\"},\"ch9\":{\"PauseBehavior\":\"0\",\"IdleBehavior\":\"0\",\"DefaultValueReg\":\"0\"},\"ch10\":{\"PauseBehavior\":\"0\",\"IdleBehavior\":\"0\",\"DefaultValueReg\":\"0\"},\"ch11\":{\"PauseBehavior\":\"0\",\"IdleBehavior\":\"0\",\"DefaultValueReg\":\"0\"},\"ch12\":{\"PauseBehavior\":\"0\",\"IdleBehavior\":\"0\",\"DefaultValueReg\":\"0\"},\"ch13\":{\"PauseBehavior\":\"0\",\"IdleBehavior\":\"0\",\"DefaultValueReg\":\"0\"},\"ch14\":{\"PauseBehavior\":\"0\",\"IdleBehavior\":\"0\",\"DefaultValueReg\":\"0\"},\"ch15\":{\"PauseBehavior\":\"0\",\"IdleBehavior\":\"0\",\"DefaultValueReg\":\"0\"},\"ch16\":{\"PauseBehavior\":\"0\",\"IdleBehavior\":\"0\",\"DefaultValueReg\":\"0\"},\"ch17\":{\"PauseBehavior\":\"0\",\"IdleBehavior\":\"0\",\"DefaultValueReg\":\"0\"},\"ch18\":{\"PauseBehavior\":\"0\",\"IdleBehavior\":\"0\",\"DefaultValueReg\":\"0\"},\"ch19\":{\"PauseBehavior\":\"0\",\"IdleBehavior\":\"0\",\"DefaultValueReg\":\"0\"},\"ch20\":{\"PauseBehavior\":\"0\",\"IdleBehavior\":\"0\",\"DefaultValueReg\":\"0\"},\"ch21\":{\"PauseBehavior\":\"0\",\"IdleBehavior\":\"0\",\"DefaultValueReg\":\"0\"},\"ch22\":{\"PauseBehavior\":\"0\",\"IdleBehavior\":\"0\",\"DefaultValueReg\":\"0\"},\"ch23\":{\"PauseBehavior\":\"0\",\"IdleBehavior\":\"0\",\"DefaultValueReg\":\"0\"},\"ch24\":{\"PauseBehavior\":\"0\",\"IdleBehavior\":\"0\",\"DefaultValueReg\":\"0\"},\"ch25\":{\"PauseBehavior\":\"0\",\"IdleBehavior\":\"0\",\"DefaultValueReg\":\"0\"},\"ch26\":{\"PauseBehavior\":\"0\",\"IdleBehavior\":\"0\",\"DefaultValueReg\":\"0\"},\"ch27\":{\"PauseBehavior\":\"0\",\"IdleBehavior\":\"0\",\"DefaultValueReg\":\"0\"},\"ch28\":{\"PauseBehavior\":\"0\",\"IdleBehavior\":\"0\",\"DefaultValueReg\":\"0\"},\"ch29\":{\"PauseBehavior\":\"0\",\"IdleBehavior\":\"0\",\"DefaultValueReg\":\"0\"},\"ch30\":{\"PauseBehavior\":\"0\",\"IdleBehavior\":\"0\",\"DefaultValueReg\":\"0\"},\"ch31\":{\"PauseBehavior\":\"0\",\"IdleBehavior\":\"0\",\"DefaultValueReg\":\"0\"}}}"  Expansion_DV_13A="{\"dv_Expansion_13A\":{\"ch0\":{\"PauseBehavior\":\"0\",\"IdleBehavior\":\"0\",\"DefaultValueReg\":\"0\"},\"ch1\":{\"PauseBehavior\":\"0\",\"IdleBehavior\":\"0\",\"DefaultValueReg\":\"0\"},\"ch2\":{\"PauseBehavior\":\"0\",\"IdleBehavior\":\"0\",\"DefaultValueReg\":\"0\"},\"ch3\":{\"PauseBehavior\":\"0\",\"IdleBehavior\":\"0\",\"DefaultValueReg\":\"0\"},\"ch4\":{\"PauseBehavior\":\"0\",\"IdleBehavior\":\"0\",\"DefaultValueReg\":\"0\"},\"ch5\":{\"PauseBehavior\":\"0\",\"IdleBehavior\":\"0\",\"DefaultValueReg\":\"0\"},\"ch6\":{\"PauseBehavior\":\"0\",\"IdleBehavior\":\"0\",\"DefaultValueReg\":\"0\"},\"ch7\":{\"PauseBehavior\":\"0\",\"IdleBehavior\":\"0\",\"DefaultValueReg\":\"0\"},\"ch8\":{\"PauseBehavior\":\"0\",\"IdleBehavior\":\"0\",\"DefaultValueReg\":\"0\"},\"ch9\":{\"PauseBehavior\":\"0\",\"IdleBehavior\":\"0\",\"DefaultValueReg\":\"0\"},\"ch10\":{\"PauseBehavior\":\"0\",\"IdleBehavior\":\"0\",\"DefaultValueReg\":\"0\"},\"ch11\":{\"PauseBehavior\":\"0\",\"IdleBehavior\":\"0\",\"DefaultValueReg\":\"0\"},\"ch12\":{\"PauseBehavior\":\"0\",\"IdleBehavior\":\"0\",\"DefaultValueReg\":\"0\"},\"ch13\":{\"PauseBehavior\":\"0\",\"IdleBehavior\":\"0\",\"DefaultValueReg\":\"0\"},\"ch14\":{\"PauseBehavior\":\"0\",\"IdleBehavior\":\"0\",\"DefaultValueReg\":\"0\"},\"ch15\":{\"PauseBehavior\":\"0\",\"IdleBehavior\":\"0\",\"DefaultValueReg\":\"0\"},\"ch16\":{\"PauseBehavior\":\"0\",\"IdleBehavior\":\"0\",\"DefaultValueReg\":\"0\"},\"ch17\":{\"PauseBehavior\":\"0\",\"IdleBehavior\":\"0\",\"DefaultValueReg\":\"0\"},\"ch18\":{\"PauseBehavior\":\"0\",\"IdleBehavior\":\"0\",\"DefaultValueReg\":\"0\"},\"ch19\":{\"PauseBehavior\":\"0\",\"IdleBehavior\":\"0\",\"DefaultValueReg\":\"0\"},\"ch20\":{\"PauseBehavior\":\"0\",\"IdleBehavior\":\"0\",\"DefaultValueReg\":\"0\"},\"ch21\":{\"PauseBehavior\":\"0\",\"IdleBehavior\":\"0\",\"DefaultValueReg\":\"0\"},\"ch22\":{\"PauseBehavior\":\"0\",\"IdleBehavior\":\"0\",\"DefaultValueReg\":\"0\"},\"ch23\":{\"PauseBehavior\":\"0\",\"IdleBehavior\":\"0\",\"DefaultValueReg\":\"0\"},\"ch24\":{\"PauseBehavior\":\"0\",\"IdleBehavior\":\"0\",\"DefaultValueReg\":\"0\"},\"ch25\":{\"PauseBehavior\":\"0\",\"IdleBehavior\":\"0\",\"DefaultValueReg\":\"0\"},\"ch26\":{\"PauseBehavior\":\"0\",\"IdleBehavior\":\"0\",\"DefaultValueReg\":\"0\"},\"ch27\":{\"PauseBehavior\":\"0\",\"IdleBehavior\":\"0\",\"DefaultValueReg\":\"0\"},\"ch28\":{\"PauseBehavior\":\"0\",\"IdleBehavior\":\"0\",\"DefaultValueReg\":\"0\"},\"ch29\":{\"PauseBehavior\":\"0\",\"IdleBehavior\":\"0\",\"DefaultValueReg\":\"0\"},\"ch30\":{\"PauseBehavior\":\"0\",\"IdleBehavior\":\"0\",\"DefaultValueReg\":\"0\"},\"ch31\":{\"PauseBehavior\":\"0\",\"IdleBehavior\":\"0\",\"DefaultValueReg\":\"0\"}}}"  Expansion_DV_13B="{\"dv_Expansion_13B\":{\"ch0\":{\"PauseBehavior\":\"0\",\"IdleBehavior\":\"0\",\"DefaultValueReg\":\"0\"},\"ch1\":{\"PauseBehavior\":\"0\",\"IdleBehavior\":\"0\",\"DefaultValueReg\":\"0\"},\"ch2\":{\"PauseBehavior\":\"0\",\"IdleBehavior\":\"0\",\"DefaultValueReg\":\"0\"},\"ch3\":{\"PauseBehavior\":\"0\",\"IdleBehavior\":\"0\",\"DefaultValueReg\":\"0\"},\"ch4\":{\"PauseBehavior\":\"0\",\"IdleBehavior\":\"0\",\"DefaultValueReg\":\"0\"},\"ch5\":{\"PauseBehavior\":\"0\",\"IdleBehavior\":\"0\",\"DefaultValueReg\":\"0\"},\"ch6\":{\"PauseBehavior\":\"0\",\"IdleBehavior\":\"0\",\"DefaultValueReg\":\"0\"},\"ch7\":{\"PauseBehavior\":\"0\",\"IdleBehavior\":\"0\",\"DefaultValueReg\":\"0\"},\"ch8\":{\"PauseBehavior\":\"0\",\"IdleBehavior\":\"0\",\"DefaultValueReg\":\"0\"},\"ch9\":{\"PauseBehavior\":\"0\",\"IdleBehavior\":\"0\",\"DefaultValueReg\":\"0\"},\"ch10\":{\"PauseBehavior\":\"0\",\"IdleBehavior\":\"0\",\"DefaultValueReg\":\"0\"},\"ch11\":{\"PauseBehavior\":\"0\",\"IdleBehavior\":\"0\",\"DefaultValueReg\":\"0\"},\"ch12\":{\"PauseBehavior\":\"0\",\"IdleBehavior\":\"0\",\"DefaultValueReg\":\"0\"},\"ch13\":{\"PauseBehavior\":\"0\",\"IdleBehavior\":\"0\",\"DefaultValueReg\":\"0\"},\"ch14\":{\"PauseBehavior\":\"0\",\"IdleBehavior\":\"0\",\"DefaultValueReg\":\"0\"},\"ch15\":{\"PauseBehavior\":\"0\",\"IdleBehavior\":\"0\",\"DefaultValueReg\":\"0\"},\"ch16\":{\"PauseBehavior\":\"0\",\"IdleBehavior\":\"0\",\"DefaultValueReg\":\"0\"},\"ch17\":{\"PauseBehavior\":\"0\",\"IdleBehavior\":\"0\",\"DefaultValueReg\":\"0\"},\"ch18\":{\"PauseBehavior\":\"0\",\"IdleBehavior\":\"0\",\"DefaultValueReg\":\"0\"},\"ch19\":{\"PauseBehavior\":\"0\",\"IdleBehavior\":\"0\",\"DefaultValueReg\":\"0\"},\"ch20\":{\"PauseBehavior\":\"0\",\"IdleBehavior\":\"0\",\"DefaultValueReg\":\"0\"},\"ch21\":{\"PauseBehavior\":\"0\",\"IdleBehavior\":\"0\",\"DefaultValueReg\":\"0\"},\"ch22\":{\"PauseBehavior\":\"0\",\"IdleBehavior\":\"0\",\"DefaultValueReg\":\"0\"},\"ch23\":{\"PauseBehavior\":\"0\",\"IdleBehavior\":\"0\",\"DefaultValueReg\":\"0\"},\"ch24\":{\"PauseBehavior\":\"0\",\"IdleBehavior\":\"0\",\"DefaultValueReg\":\"0\"},\"ch25\":{\"PauseBehavior\":\"0\",\"IdleBehavior\":\"0\",\"DefaultValueReg\":\"0\"},\"ch26\":{\"PauseBehavior\":\"0\",\"IdleBehavior\":\"0\",\"DefaultValueReg\":\"0\"},\"ch27\":{\"PauseBehavior\":\"0\",\"IdleBehavior\":\"0\",\"DefaultValueReg\":\"0\"},\"ch28\":{\"PauseBehavior\":\"0\",\"IdleBehavior\":\"0\",\"DefaultValueReg\":\"0\"},\"ch29\":{\"PauseBehavior\":\"0\",\"IdleBehavior\":\"0\",\"DefaultValueReg\":\"0\"},\"ch30\":{\"PauseBehavior\":\"0\",\"IdleBehavior\":\"0\",\"DefaultValueReg\":\"0\"},\"ch31\":{\"PauseBehavior\":\"0\",\"IdleBehavior\":\"0\",\"DefaultValueReg\":\"0\"}}}"  Slot_DV_12A="{\"dv_12A\":{\"ch0\":{\"PauseBehavior\":\"0\",\"IdleBehavior\":\"0\",\"DefaultValueReg\":\"0\"},\"ch1\":{\"PauseBehavior\":\"0\",\"IdleBehavior\":\"0\",\"DefaultValueReg\":\"0\"},\"ch2\":{\"PauseBehavior\":\"0\",\"IdleBehavior\":\"0\",\"DefaultValueReg\":\"0\"},\"ch3\":{\"PauseBehavior\":\"0\",\"IdleBehavior\":\"0\",\"DefaultValueReg\":\"0\"},\"ch4\":{\"PauseBehavior\":\"0\",\"IdleBehavior\":\"0\",\"DefaultValueReg\":\"0\"},\"ch5\":{\"PauseBehavior\":\"0\",\"IdleBehavior\":\"0\",\"DefaultValueReg\":\"0\"},\"ch6\":{\"PauseBehavior\":\"0\",\"IdleBehavior\":\"0\",\"DefaultValueReg\":\"0\"},\"ch7\":{\"PauseBehavior\":\"0\",\"IdleBehavior\":\"0\",\"DefaultValueReg\":\"0\"},\"ch8\":{\"PauseBehavior\":\"0\",\"IdleBehavior\":\"0\",\"DefaultValueReg\":\"0\"},\"ch9\":{\"PauseBehavior\":\"0\",\"IdleBehavior\":\"0\",\"DefaultValueReg\":\"0\"},\"ch10\":{\"PauseBehavior\":\"0\",\"IdleBehavior\":\"0\",\"DefaultValueReg\":\"0\"},\"ch11\":{\"PauseBehavior\":\"0\",\"IdleBehavior\":\"0\",\"DefaultValueReg\":\"0\"},\"ch12\":{\"PauseBehavior\":\"0\",\"IdleBehavior\":\"0\",\"DefaultValueReg\":\"0\"},\"ch13\":{\"PauseBehavior\":\"0\",\"IdleBehavior\":\"0\",\"DefaultValueReg\":\"0\"},\"ch14\":{\"PauseBehavior\":\"0\",\"IdleBehavior\":\"0\",\"DefaultValueReg\":\"0\"},\"ch15\":{\"PauseBehavior\":\"0\",\"IdleBehavior\":\"0\",\"DefaultValueReg\":\"0\"},\"ch16\":{\"PauseBehavior\":\"0\",\"IdleBehavior\":\"0\",\"DefaultValueReg\":\"0\"},\"ch17\":{\"PauseBehavior\":\"0\",\"IdleBehavior\":\"0\",\"DefaultValueReg\":\"0\"},\"ch18\":{\"PauseBehavior\":\"0\",\"IdleBehavior\":\"0\",\"DefaultValueReg\":\"0\"},\"ch19\":{\"PauseBehavior\":\"0\",\"IdleBehavior\":\"0\",\"DefaultValueReg\":\"0\"},\"ch20\":{\"PauseBehavior\":\"0\",\"IdleBehavior\":\"0\",\"DefaultValueReg\":\"0\"},\"ch21\":{\"PauseBehavior\":\"0\",\"IdleBehavior\":\"0\",\"DefaultValueReg\":\"0\"},\"ch22\":{\"PauseBehavior\":\"0\",\"IdleBehavior\":\"0\",\"DefaultValueReg\":\"0\"},\"ch23\":{\"PauseBehavior\":\"0\",\"IdleBehavior\":\"0\",\"DefaultValueReg\":\"0\"},\"ch24\":{\"PauseBehavior\":\"0\",\"IdleBehavior\":\"0\",\"DefaultValueReg\":\"0\"},\"ch25\":{\"PauseBehavior\":\"0\",\"IdleBehavior\":\"0\",\"DefaultValueReg\":\"0\"},\"ch26\":{\"PauseBehavior\":\"0\",\"IdleBehavior\":\"0\",\"DefaultValueReg\":\"0\"},\"ch27\":{\"PauseBehavior\":\"0\",\"IdleBehavior\":\"0\",\"DefaultValueReg\":\"0\"},\"ch28\":{\"PauseBehavior\":\"0\",\"IdleBehavior\":\"0\",\"DefaultValueReg\":\"0\"},\"ch29\":{\"PauseBehavior\":\"0\",\"IdleBehavior\":\"0\",\"DefaultValueReg\":\"0\"},\"ch30\":{\"PauseBehavior\":\"0\",\"IdleBehavior\":\"0\",\"DefaultValueReg\":\"0\"},\"ch31\":{\"PauseBehavior\":\"0\",\"IdleBehavior\":\"0\",\"DefaultValueReg\":\"0\"}}}"  Slot_DV_12B="{\"dv_12B\":{\"ch0\":{\"PauseBehavior\":\"0\",\"IdleBehavior\":\"0\",\"DefaultValueReg\":\"0\"},\"ch1\":{\"PauseBehavior\":\"0\",\"IdleBehavior\":\"0\",\"DefaultValueReg\":\"0\"},\"ch2\":{\"PauseBehavior\":\"0\",\"IdleBehavior\":\"0\",\"DefaultValueReg\":\"0\"},\"ch3\":{\"PauseBehavior\":\"0\",\"IdleBehavior\":\"0\",\"DefaultValueReg\":\"0\"},\"ch4\":{\"PauseBehavior\":\"0\",\"IdleBehavior\":\"0\",\"DefaultValueReg\":\"0\"},\"ch5\":{\"PauseBehavior\":\"0\",\"IdleBehavior\":\"0\",\"DefaultValueReg\":\"0\"},\"ch6\":{\"PauseBehavior\":\"0\",\"IdleBehavior\":\"0\",\"DefaultValueReg\":\"0\"},\"ch7\":{\"PauseBehavior\":\"0\",\"IdleBehavior\":\"0\",\"DefaultValueReg\":\"0\"},\"ch8\":{\"PauseBehavior\":\"0\",\"IdleBehavior\":\"0\",\"DefaultValueReg\":\"0\"},\"ch9\":{\"PauseBehavior\":\"0\",\"IdleBehavior\":\"0\",\"DefaultValueReg\":\"0\"},\"ch10\":{\"PauseBehavior\":\"0\",\"IdleBehavior\":\"0\",\"DefaultValueReg\":\"0\"},\"ch11\":{\"PauseBehavior\":\"0\",\"IdleBehavior\":\"0\",\"DefaultValueReg\":\"0\"},\"ch12\":{\"PauseBehavior\":\"0\",\"IdleBehavior\":\"0\",\"DefaultValueReg\":\"0\"},\"ch13\":{\"PauseBehavior\":\"0\",\"IdleBehavior\":\"0\",\"DefaultValueReg\":\"0\"},\"ch14\":{\"PauseBehavior\":\"0\",\"IdleBehavior\":\"0\",\"DefaultValueReg\":\"0\"},\"ch15\":{\"PauseBehavior\":\"0\",\"IdleBehavior\":\"0\",\"DefaultValueReg\":\"0\"},\"ch16\":{\"PauseBehavior\":\"0\",\"IdleBehavior\":\"0\",\"DefaultValueReg\":\"0\"},\"ch17\":{\"PauseBehavior\":\"0\",\"IdleBehavior\":\"0\",\"DefaultValueReg\":\"0\"},\"ch18\":{\"PauseBehavior\":\"0\",\"IdleBehavior\":\"0\",\"DefaultValueReg\":\"0\"},\"ch19\":{\"PauseBehavior\":\"0\",\"IdleBehavior\":\"0\",\"DefaultValueReg\":\"0\"},\"ch20\":{\"PauseBehavior\":\"0\",\"IdleBehavior\":\"0\",\"DefaultValueReg\":\"0\"},\"ch21\":{\"PauseBehavior\":\"0\",\"IdleBehavior\":\"0\",\"DefaultValueReg\":\"0\"},\"ch22\":{\"PauseBehavior\":\"0\",\"IdleBehavior\":\"0\",\"DefaultValueReg\":\"0\"},\"ch23\":{\"PauseBehavior\":\"0\",\"IdleBehavior\":\"0\",\"DefaultValueReg\":\"0\"},\"ch24\":{\"PauseBehavior\":\"0\",\"IdleBehavior\":\"0\",\"DefaultValueReg\":\"0\"},\"ch25\":{\"PauseBehavior\":\"0\",\"IdleBehavior\":\"0\",\"DefaultValueReg\":\"0\"},\"ch26\":{\"PauseBehavior\":\"0\",\"IdleBehavior\":\"0\",\"DefaultValueReg\":\"0\"},\"ch27\":{\"PauseBehavior\":\"0\",\"IdleBehavior\":\"0\",\"DefaultValueReg\":\"0\"},\"ch28\":{\"PauseBehavior\":\"0\",\"IdleBehavior\":\"0\",\"DefaultValueReg\":\"0\"},\"ch29\":{\"PauseBehavior\":\"0\",\"IdleBehavior\":\"0\",\"DefaultValueReg\":\"0\"},\"ch30\":{\"PauseBehavior\":\"0\",\"IdleBehavior\":\"0\",\"DefaultValueReg\":\"0\"},\"ch31\":{\"PauseBehavior\":\"0\",\"IdleBehavior\":\"0\",\"DefaultValueReg\":\"0\"}}}"  Expansion_DV_12A="{\"dv_Expansion_12A\":{\"ch0\":{\"PauseBehavior\":\"0\",\"IdleBehavior\":\"0\",\"DefaultValueReg\":\"0\"},\"ch1\":{\"PauseBehavior\":\"0\",\"IdleBehavior\":\"0\",\"DefaultValueReg\":\"0\"},\"ch2\":{\"PauseBehavior\":\"0\",\"IdleBehavior\":\"0\",\"DefaultValueReg\":\"0\"},\"ch3\":{\"PauseBehavior\":\"0\",\"IdleBehavior\":\"0\",\"DefaultValueReg\":\"0\"},\"ch4\":{\"PauseBehavior\":\"0\",\"IdleBehavior\":\"0\",\"DefaultValueReg\":\"0\"},\"ch5\":{\"PauseBehavior\":\"0\",\"IdleBehavior\":\"0\",\"DefaultValueReg\":\"0\"},\"ch6\":{\"PauseBehavior\":\"0\",\"IdleBehavior\":\"0\",\"DefaultValueReg\":\"0\"},\"ch7\":{\"PauseBehavior\":\"0\",\"IdleBehavior\":\"0\",\"DefaultValueReg\":\"0\"},\"ch8\":{\"PauseBehavior\":\"0\",\"IdleBehavior\":\"0\",\"DefaultValueReg\":\"0\"},\"ch9\":{\"PauseBehavior\":\"0\",\"IdleBehavior\":\"0\",\"DefaultValueReg\":\"0\"},\"ch10\":{\"PauseBehavior\":\"0\",\"IdleBehavior\":\"0\",\"DefaultValueReg\":\"0\"},\"ch11\":{\"PauseBehavior\":\"0\",\"IdleBehavior\":\"0\",\"DefaultValueReg\":\"0\"},\"ch12\":{\"PauseBehavior\":\"0\",\"IdleBehavior\":\"0\",\"DefaultValueReg\":\"0\"},\"ch13\":{\"PauseBehavior\":\"0\",\"IdleBehavior\":\"0\",\"DefaultValueReg\":\"0\"},\"ch14\":{\"PauseBehavior\":\"0\",\"IdleBehavior\":\"0\",\"DefaultValueReg\":\"0\"},\"ch15\":{\"PauseBehavior\":\"0\",\"IdleBehavior\":\"0\",\"DefaultValueReg\":\"0\"},\"ch16\":{\"PauseBehavior\":\"0\",\"IdleBehavior\":\"0\",\"DefaultValueReg\":\"0\"},\"ch17\":{\"PauseBehavior\":\"0\",\"IdleBehavior\":\"0\",\"DefaultValueReg\":\"0\"},\"ch18\":{\"PauseBehavior\":\"0\",\"IdleBehavior\":\"0\",\"DefaultValueReg\":\"0\"},\"ch19\":{\"PauseBehavior\":\"0\",\"IdleBehavior\":\"0\",\"DefaultValueReg\":\"0\"},\"ch20\":{\"PauseBehavior\":\"0\",\"IdleBehavior\":\"0\",\"DefaultValueReg\":\"0\"},\"ch21\":{\"PauseBehavior\":\"0\",\"IdleBehavior\":\"0\",\"DefaultValueReg\":\"0\"},\"ch22\":{\"PauseBehavior\":\"0\",\"IdleBehavior\":\"0\",\"DefaultValueReg\":\"0\"},\"ch23\":{\"PauseBehavior\":\"0\",\"IdleBehavior\":\"0\",\"DefaultValueReg\":\"0\"},\"ch24\":{\"PauseBehavior\":\"0\",\"IdleBehavior\":\"0\",\"DefaultValueReg\":\"0\"},\"ch25\":{\"PauseBehavior\":\"0\",\"IdleBehavior\":\"0\",\"DefaultValueReg\":\"0\"},\"ch26\":{\"PauseBehavior\":\"0\",\"IdleBehavior\":\"0\",\"DefaultValueReg\":\"0\"},\"ch27\":{\"PauseBehavior\":\"0\",\"IdleBehavior\":\"0\",\"DefaultValueReg\":\"0\"},\"ch28\":{\"PauseBehavior\":\"0\",\"IdleBehavior\":\"0\",\"DefaultValueReg\":\"0\"},\"ch29\":{\"PauseBehavior\":\"0\",\"IdleBehavior\":\"0\",\"DefaultValueReg\":\"0\"},\"ch30\":{\"PauseBehavior\":\"0\",\"IdleBehavior\":\"0\",\"DefaultValueReg\":\"0\"},\"ch31\":{\"PauseBehavior\":\"0\",\"IdleBehavior\":\"0\",\"DefaultValueReg\":\"0\"}}}"  Expansion_DV_12B="{\"dv_Expansion_12B\":{\"ch0\":{\"PauseBehavior\":\"0\",\"IdleBehavior\":\"0\",\"DefaultValueReg\":\"0\"},\"ch1\":{\"PauseBehavior\":\"0\",\"IdleBehavior\":\"0\",\"DefaultValueReg\":\"0\"},\"ch2\":{\"PauseBehavior\":\"0\",\"IdleBehavior\":\"0\",\"DefaultValueReg\":\"0\"},\"ch3\":{\"PauseBehavior\":\"0\",\"IdleBehavior\":\"0\",\"DefaultValueReg\":\"0\"},\"ch4\":{\"PauseBehavior\":\"0\",\"IdleBehavior\":\"0\",\"DefaultValueReg\":\"0\"},\"ch5\":{\"PauseBehavior\":\"0\",\"IdleBehavior\":\"0\",\"DefaultValueReg\":\"0\"},\"ch6\":{\"PauseBehavior\":\"0\",\"IdleBehavior\":\"0\",\"DefaultValueReg\":\"0\"},\"ch7\":{\"PauseBehavior\":\"0\",\"IdleBehavior\":\"0\",\"DefaultValueReg\":\"0\"},\"ch8\":{\"PauseBehavior\":\"0\",\"IdleBehavior\":\"0\",\"DefaultValueReg\":\"0\"},\"ch9\":{\"PauseBehavior\":\"0\",\"IdleBehavior\":\"0\",\"DefaultValueReg\":\"0\"},\"ch10\":{\"PauseBehavior\":\"0\",\"IdleBehavior\":\"0\",\"DefaultValueReg\":\"0\"},\"ch11\":{\"PauseBehavior\":\"0\",\"IdleBehavior\":\"0\",\"DefaultValueReg\":\"0\"},\"ch12\":{\"PauseBehavior\":\"0\",\"IdleBehavior\":\"0\",\"DefaultValueReg\":\"0\"},\"ch13\":{\"PauseBehavior\":\"0\",\"IdleBehavior\":\"0\",\"DefaultValueReg\":\"0\"},\"ch14\":{\"PauseBehavior\":\"0\",\"IdleBehavior\":\"0\",\"DefaultValueReg\":\"0\"},\"ch15\":{\"PauseBehavior\":\"0\",\"IdleBehavior\":\"0\",\"DefaultValueReg\":\"0\"},\"ch16\":{\"PauseBehavior\":\"0\",\"IdleBehavior\":\"0\",\"DefaultValueReg\":\"0\"},\"ch17\":{\"PauseBehavior\":\"0\",\"IdleBehavior\":\"0\",\"DefaultValueReg\":\"0\"},\"ch18\":{\"PauseBehavior\":\"0\",\"IdleBehavior\":\"0\",\"DefaultValueReg\":\"0\"},\"ch19\":{\"PauseBehavior\":\"0\",\"IdleBehavior\":\"0\",\"DefaultValueReg\":\"0\"},\"ch20\":{\"PauseBehavior\":\"0\",\"IdleBehavior\":\"0\",\"DefaultValueReg\":\"0\"},\"ch21\":{\"PauseBehavior\":\"0\",\"IdleBehavior\":\"0\",\"DefaultValueReg\":\"0\"},\"ch22\":{\"PauseBehavior\":\"0\",\"IdleBehavior\":\"0\",\"DefaultValueReg\":\"0\"},\"ch23\":{\"PauseBehavior\":\"0\",\"IdleBehavior\":\"0\",\"DefaultValueReg\":\"0\"},\"ch24\":{\"PauseBehavior\":\"0\",\"IdleBehavior\":\"0\",\"DefaultValueReg\":\"0\"},\"ch25\":{\"PauseBehavior\":\"0\",\"IdleBehavior\":\"0\",\"DefaultValueReg\":\"0\"},\"ch26\":{\"PauseBehavior\":\"0\",\"IdleBehavior\":\"0\",\"DefaultValueReg\":\"0\"},\"ch27\":{\"PauseBehavior\":\"0\",\"IdleBehavior\":\"0\",\"DefaultValueReg\":\"0\"},\"ch28\":{\"PauseBehavior\":\"0\",\"IdleBehavior\":\"0\",\"DefaultValueReg\":\"0\"},\"ch29\":{\"PauseBehavior\":\"0\",\"IdleBehavior\":\"0\",\"DefaultValueReg\":\"0\"},\"ch30\":{\"PauseBehavior\":\"0\",\"IdleBehavior\":\"0\",\"DefaultValueReg\":\"0\"},\"ch31\":{\"PauseBehavior\":\"0\",\"IdleBehavior\":\"0\",\"DefaultValueReg\":\"0\"}}}"  Slot_DV_11A="{\"dv_11A\":{\"ch0\":{\"PauseBehavior\":\"0\",\"IdleBehavior\":\"0\",\"DefaultValueReg\":\"0\"},\"ch1\":{\"PauseBehavior\":\"0\",\"IdleBehavior\":\"0\",\"DefaultValueReg\":\"0\"},\"ch2\":{\"PauseBehavior\":\"0\",\"IdleBehavior\":\"0\",\"DefaultValueReg\":\"0\"},\"ch3\":{\"PauseBehavior\":\"0\",\"IdleBehavior\":\"0\",\"DefaultValueReg\":\"0\"},\"ch4\":{\"PauseBehavior\":\"0\",\"IdleBehavior\":\"0\",\"DefaultValueReg\":\"0\"},\"ch5\":{\"PauseBehavior\":\"0\",\"IdleBehavior\":\"0\",\"DefaultValueReg\":\"0\"},\"ch6\":{\"PauseBehavior\":\"0\",\"IdleBehavior\":\"0\",\"DefaultValueReg\":\"0\"},\"ch7\":{\"PauseBehavior\":\"0\",\"IdleBehavior\":\"0\",\"DefaultValueReg\":\"0\"},\"ch8\":{\"PauseBehavior\":\"0\",\"IdleBehavior\":\"0\",\"DefaultValueReg\":\"0\"},\"ch9\":{\"PauseBehavior\":\"0\",\"IdleBehavior\":\"0\",\"DefaultValueReg\":\"0\"},\"ch10\":{\"PauseBehavior\":\"0\",\"IdleBehavior\":\"0\",\"DefaultValueReg\":\"0\"},\"ch11\":{\"PauseBehavior\":\"0\",\"IdleBehavior\":\"0\",\"DefaultValueReg\":\"0\"},\"ch12\":{\"PauseBehavior\":\"0\",\"IdleBehavior\":\"0\",\"DefaultValueReg\":\"0\"},\"ch13\":{\"PauseBehavior\":\"0\",\"IdleBehavior\":\"0\",\"DefaultValueReg\":\"0\"},\"ch14\":{\"PauseBehavior\":\"0\",\"IdleBehavior\":\"0\",\"DefaultValueReg\":\"0\"},\"ch15\":{\"PauseBehavior\":\"0\",\"IdleBehavior\":\"0\",\"DefaultValueReg\":\"0\"},\"ch16\":{\"PauseBehavior\":\"0\",\"IdleBehavior\":\"0\",\"DefaultValueReg\":\"0\"},\"ch17\":{\"PauseBehavior\":\"0\",\"IdleBehavior\":\"0\",\"DefaultValueReg\":\"0\"},\"ch18\":{\"PauseBehavior\":\"0\",\"IdleBehavior\":\"0\",\"DefaultValueReg\":\"0\"},\"ch19\":{\"PauseBehavior\":\"0\",\"IdleBehavior\":\"0\",\"DefaultValueReg\":\"0\"},\"ch20\":{\"PauseBehavior\":\"0\",\"IdleBehavior\":\"0\",\"DefaultValueReg\":\"0\"},\"ch21\":{\"PauseBehavior\":\"0\",\"IdleBehavior\":\"0\",\"DefaultValueReg\":\"0\"},\"ch22\":{\"PauseBehavior\":\"0\",\"IdleBehavior\":\"0\",\"DefaultValueReg\":\"0\"},\"ch23\":{\"PauseBehavior\":\"0\",\"IdleBehavior\":\"0\",\"DefaultValueReg\":\"0\"},\"ch24\":{\"PauseBehavior\":\"0\",\"IdleBehavior\":\"0\",\"DefaultValueReg\":\"0\"},\"ch25\":{\"PauseBehavior\":\"0\",\"IdleBehavior\":\"0\",\"DefaultValueReg\":\"0\"},\"ch26\":{\"PauseBehavior\":\"0\",\"IdleBehavior\":\"0\",\"DefaultValueReg\":\"0\"},\"ch27\":{\"PauseBehavior\":\"0\",\"IdleBehavior\":\"0\",\"DefaultValueReg\":\"0\"},\"ch28\":{\"PauseBehavior\":\"0\",\"IdleBehavior\":\"0\",\"DefaultValueReg\":\"0\"},\"ch29\":{\"PauseBehavior\":\"0\",\"IdleBehavior\":\"0\",\"DefaultValueReg\":\"0\"},\"ch30\":{\"PauseBehavior\":\"0\",\"IdleBehavior\":\"0\",\"DefaultValueReg\":\"0\"},\"ch31\":{\"PauseBehavior\":\"0\",\"IdleBehavior\":\"0\",\"DefaultValueReg\":\"0\"}}}"  Slot_DV_11B="{\"dv_11B\":{\"ch0\":{\"PauseBehavior\":\"0\",\"IdleBehavior\":\"0\",\"DefaultValueReg\":\"0\"},\"ch1\":{\"PauseBehavior\":\"0\",\"IdleBehavior\":\"0\",\"DefaultValueReg\":\"0\"},\"ch2\":{\"PauseBehavior\":\"0\",\"IdleBehavior\":\"0\",\"DefaultValueReg\":\"0\"},\"ch3\":{\"PauseBehavior\":\"0\",\"IdleBehavior\":\"0\",\"DefaultValueReg\":\"0\"},\"ch4\":{\"PauseBehavior\":\"0\",\"IdleBehavior\":\"0\",\"DefaultValueReg\":\"0\"},\"ch5\":{\"PauseBehavior\":\"0\",\"IdleBehavior\":\"0\",\"DefaultValueReg\":\"0\"},\"ch6\":{\"PauseBehavior\":\"0\",\"IdleBehavior\":\"0\",\"DefaultValueReg\":\"0\"},\"ch7\":{\"PauseBehavior\":\"0\",\"IdleBehavior\":\"0\",\"DefaultValueReg\":\"0\"},\"ch8\":{\"PauseBehavior\":\"0\",\"IdleBehavior\":\"0\",\"DefaultValueReg\":\"0\"},\"ch9\":{\"PauseBehavior\":\"0\",\"IdleBehavior\":\"0\",\"DefaultValueReg\":\"0\"},\"ch10\":{\"PauseBehavior\":\"0\",\"IdleBehavior\":\"0\",\"DefaultValueReg\":\"0\"},\"ch11\":{\"PauseBehavior\":\"0\",\"IdleBehavior\":\"0\",\"DefaultValueReg\":\"0\"},\"ch12\":{\"PauseBehavior\":\"0\",\"IdleBehavior\":\"0\",\"DefaultValueReg\":\"0\"},\"ch13\":{\"PauseBehavior\":\"0\",\"IdleBehavior\":\"0\",\"DefaultValueReg\":\"0\"},\"ch14\":{\"PauseBehavior\":\"0\",\"IdleBehavior\":\"0\",\"DefaultValueReg\":\"0\"},\"ch15\":{\"PauseBehavior\":\"0\",\"IdleBehavior\":\"0\",\"DefaultValueReg\":\"0\"},\"ch16\":{\"PauseBehavior\":\"0\",\"IdleBehavior\":\"0\",\"DefaultValueReg\":\"0\"},\"ch17\":{\"PauseBehavior\":\"0\",\"IdleBehavior\":\"0\",\"DefaultValueReg\":\"0\"},\"ch18\":{\"PauseBehavior\":\"0\",\"IdleBehavior\":\"0\",\"DefaultValueReg\":\"0\"},\"ch19\":{\"PauseBehavior\":\"0\",\"IdleBehavior\":\"0\",\"DefaultValueReg\":\"0\"},\"ch20\":{\"PauseBehavior\":\"0\",\"IdleBehavior\":\"0\",\"DefaultValueReg\":\"0\"},\"ch21\":{\"PauseBehavior\":\"0\",\"IdleBehavior\":\"0\",\"DefaultValueReg\":\"0\"},\"ch22\":{\"PauseBehavior\":\"0\",\"IdleBehavior\":\"0\",\"DefaultValueReg\":\"0\"},\"ch23\":{\"PauseBehavior\":\"0\",\"IdleBehavior\":\"0\",\"DefaultValueReg\":\"0\"},\"ch24\":{\"PauseBehavior\":\"0\",\"IdleBehavior\":\"0\",\"DefaultValueReg\":\"0\"},\"ch25\":{\"PauseBehavior\":\"0\",\"IdleBehavior\":\"0\",\"DefaultValueReg\":\"0\"},\"ch26\":{\"PauseBehavior\":\"0\",\"IdleBehavior\":\"0\",\"DefaultValueReg\":\"0\"},\"ch27\":{\"PauseBehavior\":\"0\",\"IdleBehavior\":\"0\",\"DefaultValueReg\":\"0\"},\"ch28\":{\"PauseBehavior\":\"0\",\"IdleBehavior\":\"0\",\"DefaultValueReg\":\"0\"},\"ch29\":{\"PauseBehavior\":\"0\",\"IdleBehavior\":\"0\",\"DefaultValueReg\":\"0\"},\"ch30\":{\"PauseBehavior\":\"0\",\"IdleBehavior\":\"0\",\"DefaultValueReg\":\"0\"},\"ch31\":{\"PauseBehavior\":\"0\",\"IdleBehavior\":\"0\",\"DefaultValueReg\":\"0\"}}}"  Expansion_DV_11A="{\"dv_Expansion_11A\":{\"ch0\":{\"PauseBehavior\":\"0\",\"IdleBehavior\":\"0\",\"DefaultValueReg\":\"0\"},\"ch1\":{\"PauseBehavior\":\"0\",\"IdleBehavior\":\"0\",\"DefaultValueReg\":\"0\"},\"ch2\":{\"PauseBehavior\":\"0\",\"IdleBehavior\":\"0\",\"DefaultValueReg\":\"0\"},\"ch3\":{\"PauseBehavior\":\"0\",\"IdleBehavior\":\"0\",\"DefaultValueReg\":\"0\"},\"ch4\":{\"PauseBehavior\":\"0\",\"IdleBehavior\":\"0\",\"DefaultValueReg\":\"0\"},\"ch5\":{\"PauseBehavior\":\"0\",\"IdleBehavior\":\"0\",\"DefaultValueReg\":\"0\"},\"ch6\":{\"PauseBehavior\":\"0\",\"IdleBehavior\":\"0\",\"DefaultValueReg\":\"0\"},\"ch7\":{\"PauseBehavior\":\"0\",\"IdleBehavior\":\"0\",\"DefaultValueReg\":\"0\"},\"ch8\":{\"PauseBehavior\":\"0\",\"IdleBehavior\":\"0\",\"DefaultValueReg\":\"0\"},\"ch9\":{\"PauseBehavior\":\"0\",\"IdleBehavior\":\"0\",\"DefaultValueReg\":\"0\"},\"ch10\":{\"PauseBehavior\":\"0\",\"IdleBehavior\":\"0\",\"DefaultValueReg\":\"0\"},\"ch11\":{\"PauseBehavior\":\"0\",\"IdleBehavior\":\"0\",\"DefaultValueReg\":\"0\"},\"ch12\":{\"PauseBehavior\":\"0\",\"IdleBehavior\":\"0\",\"DefaultValueReg\":\"0\"},\"ch13\":{\"PauseBehavior\":\"0\",\"IdleBehavior\":\"0\",\"DefaultValueReg\":\"0\"},\"ch14\":{\"PauseBehavior\":\"0\",\"IdleBehavior\":\"0\",\"DefaultValueReg\":\"0\"},\"ch15\":{\"PauseBehavior\":\"0\",\"IdleBehavior\":\"0\",\"DefaultValueReg\":\"0\"},\"ch16\":{\"PauseBehavior\":\"0\",\"IdleBehavior\":\"0\",\"DefaultValueReg\":\"0\"},\"ch17\":{\"PauseBehavior\":\"0\",\"IdleBehavior\":\"0\",\"DefaultValueReg\":\"0\"},\"ch18\":{\"PauseBehavior\":\"0\",\"IdleBehavior\":\"0\",\"DefaultValueReg\":\"0\"},\"ch19\":{\"PauseBehavior\":\"0\",\"IdleBehavior\":\"0\",\"DefaultValueReg\":\"0\"},\"ch20\":{\"PauseBehavior\":\"0\",\"IdleBehavior\":\"0\",\"DefaultValueReg\":\"0\"},\"ch21\":{\"PauseBehavior\":\"0\",\"IdleBehavior\":\"0\",\"DefaultValueReg\":\"0\"},\"ch22\":{\"PauseBehavior\":\"0\",\"IdleBehavior\":\"0\",\"DefaultValueReg\":\"0\"},\"ch23\":{\"PauseBehavior\":\"0\",\"IdleBehavior\":\"0\",\"DefaultValueReg\":\"0\"},\"ch24\":{\"PauseBehavior\":\"0\",\"IdleBehavior\":\"0\",\"DefaultValueReg\":\"0\"},\"ch25\":{\"PauseBehavior\":\"0\",\"IdleBehavior\":\"0\",\"DefaultValueReg\":\"0\"},\"ch26\":{\"PauseBehavior\":\"0\",\"IdleBehavior\":\"0\",\"DefaultValueReg\":\"0\"},\"ch27\":{\"PauseBehavior\":\"0\",\"IdleBehavior\":\"0\",\"DefaultValueReg\":\"0\"},\"ch28\":{\"PauseBehavior\":\"0\",\"IdleBehavior\":\"0\",\"DefaultValueReg\":\"0\"},\"ch29\":{\"PauseBehavior\":\"0\",\"IdleBehavior\":\"0\",\"DefaultValueReg\":\"0\"},\"ch30\":{\"PauseBehavior\":\"0\",\"IdleBehavior\":\"0\",\"DefaultValueReg\":\"0\"},\"ch31\":{\"PauseBehavior\":\"0\",\"IdleBehavior\":\"0\",\"DefaultValueReg\":\"0\"}}}"  Expansion_DV_11B="{\"dv_Expansion_11B\":{\"ch0\":{\"PauseBehavior\":\"0\",\"IdleBehavior\":\"0\",\"DefaultValueReg\":\"0\"},\"ch1\":{\"PauseBehavior\":\"0\",\"IdleBehavior\":\"0\",\"DefaultValueReg\":\"0\"},\"ch2\":{\"PauseBehavior\":\"0\",\"IdleBehavior\":\"0\",\"DefaultValueReg\":\"0\"},\"ch3\":{\"PauseBehavior\":\"0\",\"IdleBehavior\":\"0\",\"DefaultValueReg\":\"0\"},\"ch4\":{\"PauseBehavior\":\"0\",\"IdleBehavior\":\"0\",\"DefaultValueReg\":\"0\"},\"ch5\":{\"PauseBehavior\":\"0\",\"IdleBehavior\":\"0\",\"DefaultValueReg\":\"0\"},\"ch6\":{\"PauseBehavior\":\"0\",\"IdleBehavior\":\"0\",\"DefaultValueReg\":\"0\"},\"ch7\":{\"PauseBehavior\":\"0\",\"IdleBehavior\":\"0\",\"DefaultValueReg\":\"0\"},\"ch8\":{\"PauseBehavior\":\"0\",\"IdleBehavior\":\"0\",\"DefaultValueReg\":\"0\"},\"ch9\":{\"PauseBehavior\":\"0\",\"IdleBehavior\":\"0\",\"DefaultValueReg\":\"0\"},\"ch10\":{\"PauseBehavior\":\"0\",\"IdleBehavior\":\"0\",\"DefaultValueReg\":\"0\"},\"ch11\":{\"PauseBehavior\":\"0\",\"IdleBehavior\":\"0\",\"DefaultValueReg\":\"0\"},\"ch12\":{\"PauseBehavior\":\"0\",\"IdleBehavior\":\"0\",\"DefaultValueReg\":\"0\"},\"ch13\":{\"PauseBehavior\":\"0\",\"IdleBehavior\":\"0\",\"DefaultValueReg\":\"0\"},\"ch14\":{\"PauseBehavior\":\"0\",\"IdleBehavior\":\"0\",\"DefaultValueReg\":\"0\"},\"ch15\":{\"PauseBehavior\":\"0\",\"IdleBehavior\":\"0\",\"DefaultValueReg\":\"0\"},\"ch16\":{\"PauseBehavior\":\"0\",\"IdleBehavior\":\"0\",\"DefaultValueReg\":\"0\"},\"ch17\":{\"PauseBehavior\":\"0\",\"IdleBehavior\":\"0\",\"DefaultValueReg\":\"0\"},\"ch18\":{\"PauseBehavior\":\"0\",\"IdleBehavior\":\"0\",\"DefaultValueReg\":\"0\"},\"ch19\":{\"PauseBehavior\":\"0\",\"IdleBehavior\":\"0\",\"DefaultValueReg\":\"0\"},\"ch20\":{\"PauseBehavior\":\"0\",\"IdleBehavior\":\"0\",\"DefaultValueReg\":\"0\"},\"ch21\":{\"PauseBehavior\":\"0\",\"IdleBehavior\":\"0\",\"DefaultValueReg\":\"0\"},\"ch22\":{\"PauseBehavior\":\"0\",\"IdleBehavior\":\"0\",\"DefaultValueReg\":\"0\"},\"ch23\":{\"PauseBehavior\":\"0\",\"IdleBehavior\":\"0\",\"DefaultValueReg\":\"0\"},\"ch24\":{\"PauseBehavior\":\"0\",\"IdleBehavior\":\"0\",\"DefaultValueReg\":\"0\"},\"ch25\":{\"PauseBehavior\":\"0\",\"IdleBehavior\":\"0\",\"DefaultValueReg\":\"0\"},\"ch26\":{\"PauseBehavior\":\"0\",\"IdleBehavior\":\"0\",\"DefaultValueReg\":\"0\"},\"ch27\":{\"PauseBehavior\":\"0\",\"IdleBehavior\":\"0\",\"DefaultValueReg\":\"0\"},\"ch28\":{\"PauseBehavior\":\"0\",\"IdleBehavior\":\"0\",\"DefaultValueReg\":\"0\"},\"ch29\":{\"PauseBehavior\":\"0\",\"IdleBehavior\":\"0\",\"DefaultValueReg\":\"0\"},\"ch30\":{\"PauseBehavior\":\"0\",\"IdleBehavior\":\"0\",\"DefaultValueReg\":\"0\"},\"ch31\":{\"PauseBehavior\":\"0\",\"IdleBehavior\":\"0\",\"DefaultValueReg\":\"0\"}}}"  Slot_DV_10A="{\"dv_10A\":{\"ch0\":{\"PauseBehavior\":\"0\",\"IdleBehavior\":\"0\",\"DefaultValueReg\":\"0\"},\"ch1\":{\"PauseBehavior\":\"0\",\"IdleBehavior\":\"0\",\"DefaultValueReg\":\"0\"},\"ch2\":{\"PauseBehavior\":\"0\",\"IdleBehavior\":\"0\",\"DefaultValueReg\":\"0\"},\"ch3\":{\"PauseBehavior\":\"0\",\"IdleBehavior\":\"0\",\"DefaultValueReg\":\"0\"},\"ch4\":{\"PauseBehavior\":\"0\",\"IdleBehavior\":\"0\",\"DefaultValueReg\":\"0\"},\"ch5\":{\"PauseBehavior\":\"0\",\"IdleBehavior\":\"0\",\"DefaultValueReg\":\"0\"},\"ch6\":{\"PauseBehavior\":\"0\",\"IdleBehavior\":\"0\",\"DefaultValueReg\":\"0\"},\"ch7\":{\"PauseBehavior\":\"0\",\"IdleBehavior\":\"0\",\"DefaultValueReg\":\"0\"},\"ch8\":{\"PauseBehavior\":\"0\",\"IdleBehavior\":\"0\",\"DefaultValueReg\":\"0\"},\"ch9\":{\"PauseBehavior\":\"0\",\"IdleBehavior\":\"0\",\"DefaultValueReg\":\"0\"},\"ch10\":{\"PauseBehavior\":\"0\",\"IdleBehavior\":\"0\",\"DefaultValueReg\":\"0\"},\"ch11\":{\"PauseBehavior\":\"0\",\"IdleBehavior\":\"0\",\"DefaultValueReg\":\"0\"},\"ch12\":{\"PauseBehavior\":\"0\",\"IdleBehavior\":\"0\",\"DefaultValueReg\":\"0\"},\"ch13\":{\"PauseBehavior\":\"0\",\"IdleBehavior\":\"0\",\"DefaultValueReg\":\"0\"},\"ch14\":{\"PauseBehavior\":\"0\",\"IdleBehavior\":\"0\",\"DefaultValueReg\":\"0\"},\"ch15\":{\"PauseBehavior\":\"0\",\"IdleBehavior\":\"0\",\"DefaultValueReg\":\"0\"},\"ch16\":{\"PauseBehavior\":\"0\",\"IdleBehavior\":\"0\",\"DefaultValueReg\":\"0\"},\"ch17\":{\"PauseBehavior\":\"0\",\"IdleBehavior\":\"0\",\"DefaultValueReg\":\"0\"},\"ch18\":{\"PauseBehavior\":\"0\",\"IdleBehavior\":\"0\",\"DefaultValueReg\":\"0\"},\"ch19\":{\"PauseBehavior\":\"0\",\"IdleBehavior\":\"0\",\"DefaultValueReg\":\"0\"},\"ch20\":{\"PauseBehavior\":\"0\",\"IdleBehavior\":\"0\",\"DefaultValueReg\":\"0\"},\"ch21\":{\"PauseBehavior\":\"0\",\"IdleBehavior\":\"0\",\"DefaultValueReg\":\"0\"},\"ch22\":{\"PauseBehavior\":\"0\",\"IdleBehavior\":\"0\",\"DefaultValueReg\":\"0\"},\"ch23\":{\"PauseBehavior\":\"0\",\"IdleBehavior\":\"0\",\"DefaultValueReg\":\"0\"},\"ch24\":{\"PauseBehavior\":\"0\",\"IdleBehavior\":\"0\",\"DefaultValueReg\":\"0\"},\"ch25\":{\"PauseBehavior\":\"0\",\"IdleBehavior\":\"0\",\"DefaultValueReg\":\"0\"},\"ch26\":{\"PauseBehavior\":\"0\",\"IdleBehavior\":\"0\",\"DefaultValueReg\":\"0\"},\"ch27\":{\"PauseBehavior\":\"0\",\"IdleBehavior\":\"0\",\"DefaultValueReg\":\"0\"},\"ch28\":{\"PauseBehavior\":\"0\",\"IdleBehavior\":\"0\",\"DefaultValueReg\":\"0\"},\"ch29\":{\"PauseBehavior\":\"0\",\"IdleBehavior\":\"0\",\"DefaultValueReg\":\"0\"},\"ch30\":{\"PauseBehavior\":\"0\",\"IdleBehavior\":\"0\",\"DefaultValueReg\":\"0\"},\"ch31\":{\"PauseBehavior\":\"0\",\"IdleBehavior\":\"0\",\"DefaultValueReg\":\"0\"}}}"  Slot_DV_10B="{\"dv_10B\":{\"ch0\":{\"PauseBehavior\":\"0\",\"IdleBehavior\":\"0\",\"DefaultValueReg\":\"0\"},\"ch1\":{\"PauseBehavior\":\"0\",\"IdleBehavior\":\"0\",\"DefaultValueReg\":\"0\"},\"ch2\":{\"PauseBehavior\":\"0\",\"IdleBehavior\":\"0\",\"DefaultValueReg\":\"0\"},\"ch3\":{\"PauseBehavior\":\"0\",\"IdleBehavior\":\"0\",\"DefaultValueReg\":\"0\"},\"ch4\":{\"PauseBehavior\":\"0\",\"IdleBehavior\":\"0\",\"DefaultValueReg\":\"0\"},\"ch5\":{\"PauseBehavior\":\"0\",\"IdleBehavior\":\"0\",\"DefaultValueReg\":\"0\"},\"ch6\":{\"PauseBehavior\":\"0\",\"IdleBehavior\":\"0\",\"DefaultValueReg\":\"0\"},\"ch7\":{\"PauseBehavior\":\"0\",\"IdleBehavior\":\"0\",\"DefaultValueReg\":\"0\"},\"ch8\":{\"PauseBehavior\":\"0\",\"IdleBehavior\":\"0\",\"DefaultValueReg\":\"0\"},\"ch9\":{\"PauseBehavior\":\"0\",\"IdleBehavior\":\"0\",\"DefaultValueReg\":\"0\"},\"ch10\":{\"PauseBehavior\":\"0\",\"IdleBehavior\":\"0\",\"DefaultValueReg\":\"0\"},\"ch11\":{\"PauseBehavior\":\"0\",\"IdleBehavior\":\"0\",\"DefaultValueReg\":\"0\"},\"ch12\":{\"PauseBehavior\":\"0\",\"IdleBehavior\":\"0\",\"DefaultValueReg\":\"0\"},\"ch13\":{\"PauseBehavior\":\"0\",\"IdleBehavior\":\"0\",\"DefaultValueReg\":\"0\"},\"ch14\":{\"PauseBehavior\":\"0\",\"IdleBehavior\":\"0\",\"DefaultValueReg\":\"0\"},\"ch15\":{\"PauseBehavior\":\"0\",\"IdleBehavior\":\"0\",\"DefaultValueReg\":\"0\"},\"ch16\":{\"PauseBehavior\":\"0\",\"IdleBehavior\":\"0\",\"DefaultValueReg\":\"0\"},\"ch17\":{\"PauseBehavior\":\"0\",\"IdleBehavior\":\"0\",\"DefaultValueReg\":\"0\"},\"ch18\":{\"PauseBehavior\":\"0\",\"IdleBehavior\":\"0\",\"DefaultValueReg\":\"0\"},\"ch19\":{\"PauseBehavior\":\"0\",\"IdleBehavior\":\"0\",\"DefaultValueReg\":\"0\"},\"ch20\":{\"PauseBehavior\":\"0\",\"IdleBehavior\":\"0\",\"DefaultValueReg\":\"0\"},\"ch21\":{\"PauseBehavior\":\"0\",\"IdleBehavior\":\"0\",\"DefaultValueReg\":\"0\"},\"ch22\":{\"PauseBehavior\":\"0\",\"IdleBehavior\":\"0\",\"DefaultValueReg\":\"0\"},\"ch23\":{\"PauseBehavior\":\"0\",\"IdleBehavior\":\"0\",\"DefaultValueReg\":\"0\"},\"ch24\":{\"PauseBehavior\":\"0\",\"IdleBehavior\":\"0\",\"DefaultValueReg\":\"0\"},\"ch25\":{\"PauseBehavior\":\"0\",\"IdleBehavior\":\"0\",\"DefaultValueReg\":\"0\"},\"ch26\":{\"PauseBehavior\":\"0\",\"IdleBehavior\":\"0\",\"DefaultValueReg\":\"0\"},\"ch27\":{\"PauseBehavior\":\"0\",\"IdleBehavior\":\"0\",\"DefaultValueReg\":\"0\"},\"ch28\":{\"PauseBehavior\":\"0\",\"IdleBehavior\":\"0\",\"DefaultValueReg\":\"0\"},\"ch29\":{\"PauseBehavior\":\"0\",\"IdleBehavior\":\"0\",\"DefaultValueReg\":\"0\"},\"ch30\":{\"PauseBehavior\":\"0\",\"IdleBehavior\":\"0\",\"DefaultValueReg\":\"0\"},\"ch31\":{\"PauseBehavior\":\"0\",\"IdleBehavior\":\"0\",\"DefaultValueReg\":\"0\"}}}"  Expansion_DV_10A="{\"dv_Expansion_10A\":{\"ch0\":{\"PauseBehavior\":\"0\",\"IdleBehavior\":\"0\",\"DefaultValueReg\":\"0\"},\"ch1\":{\"PauseBehavior\":\"0\",\"IdleBehavior\":\"0\",\"DefaultValueReg\":\"0\"},\"ch2\":{\"PauseBehavior\":\"0\",\"IdleBehavior\":\"0\",\"DefaultValueReg\":\"0\"},\"ch3\":{\"PauseBehavior\":\"0\",\"IdleBehavior\":\"0\",\"DefaultValueReg\":\"0\"},\"ch4\":{\"PauseBehavior\":\"0\",\"IdleBehavior\":\"0\",\"DefaultValueReg\":\"0\"},\"ch5\":{\"PauseBehavior\":\"0\",\"IdleBehavior\":\"0\",\"DefaultValueReg\":\"0\"},\"ch6\":{\"PauseBehavior\":\"0\",\"IdleBehavior\":\"0\",\"DefaultValueReg\":\"0\"},\"ch7\":{\"PauseBehavior\":\"0\",\"IdleBehavior\":\"0\",\"DefaultValueReg\":\"0\"},\"ch8\":{\"PauseBehavior\":\"0\",\"IdleBehavior\":\"0\",\"DefaultValueReg\":\"0\"},\"ch9\":{\"PauseBehavior\":\"0\",\"IdleBehavior\":\"0\",\"DefaultValueReg\":\"0\"},\"ch10\":{\"PauseBehavior\":\"0\",\"IdleBehavior\":\"0\",\"DefaultValueReg\":\"0\"},\"ch11\":{\"PauseBehavior\":\"0\",\"IdleBehavior\":\"0\",\"DefaultValueReg\":\"0\"},\"ch12\":{\"PauseBehavior\":\"0\",\"IdleBehavior\":\"0\",\"DefaultValueReg\":\"0\"},\"ch13\":{\"PauseBehavior\":\"0\",\"IdleBehavior\":\"0\",\"DefaultValueReg\":\"0\"},\"ch14\":{\"PauseBehavior\":\"0\",\"IdleBehavior\":\"0\",\"DefaultValueReg\":\"0\"},\"ch15\":{\"PauseBehavior\":\"0\",\"IdleBehavior\":\"0\",\"DefaultValueReg\":\"0\"},\"ch16\":{\"PauseBehavior\":\"0\",\"IdleBehavior\":\"0\",\"DefaultValueReg\":\"0\"},\"ch17\":{\"PauseBehavior\":\"0\",\"IdleBehavior\":\"0\",\"DefaultValueReg\":\"0\"},\"ch18\":{\"PauseBehavior\":\"0\",\"IdleBehavior\":\"0\",\"DefaultValueReg\":\"0\"},\"ch19\":{\"PauseBehavior\":\"0\",\"IdleBehavior\":\"0\",\"DefaultValueReg\":\"0\"},\"ch20\":{\"PauseBehavior\":\"0\",\"IdleBehavior\":\"0\",\"DefaultValueReg\":\"0\"},\"ch21\":{\"PauseBehavior\":\"0\",\"IdleBehavior\":\"0\",\"DefaultValueReg\":\"0\"},\"ch22\":{\"PauseBehavior\":\"0\",\"IdleBehavior\":\"0\",\"DefaultValueReg\":\"0\"},\"ch23\":{\"PauseBehavior\":\"0\",\"IdleBehavior\":\"0\",\"DefaultValueReg\":\"0\"},\"ch24\":{\"PauseBehavior\":\"0\",\"IdleBehavior\":\"0\",\"DefaultValueReg\":\"0\"},\"ch25\":{\"PauseBehavior\":\"0\",\"IdleBehavior\":\"0\",\"DefaultValueReg\":\"0\"},\"ch26\":{\"PauseBehavior\":\"0\",\"IdleBehavior\":\"0\",\"DefaultValueReg\":\"0\"},\"ch27\":{\"PauseBehavior\":\"0\",\"IdleBehavior\":\"0\",\"DefaultValueReg\":\"0\"},\"ch28\":{\"PauseBehavior\":\"0\",\"IdleBehavior\":\"0\",\"DefaultValueReg\":\"0\"},\"ch29\":{\"PauseBehavior\":\"0\",\"IdleBehavior\":\"0\",\"DefaultValueReg\":\"0\"},\"ch30\":{\"PauseBehavior\":\"0\",\"IdleBehavior\":\"0\",\"DefaultValueReg\":\"0\"},\"ch31\":{\"PauseBehavior\":\"0\",\"IdleBehavior\":\"0\",\"DefaultValueReg\":\"0\"}}}"  Expansion_DV_10B="{\"dv_Expansion_10B\":{\"ch0\":{\"PauseBehavior\":\"0\",\"IdleBehavior\":\"0\",\"DefaultValueReg\":\"0\"},\"ch1\":{\"PauseBehavior\":\"0\",\"IdleBehavior\":\"0\",\"DefaultValueReg\":\"0\"},\"ch2\":{\"PauseBehavior\":\"0\",\"IdleBehavior\":\"0\",\"DefaultValueReg\":\"0\"},\"ch3\":{\"PauseBehavior\":\"0\",\"IdleBehavior\":\"0\",\"DefaultValueReg\":\"0\"},\"ch4\":{\"PauseBehavior\":\"0\",\"IdleBehavior\":\"0\",\"DefaultValueReg\":\"0\"},\"ch5\":{\"PauseBehavior\":\"0\",\"IdleBehavior\":\"0\",\"DefaultValueReg\":\"0\"},\"ch6\":{\"PauseBehavior\":\"0\",\"IdleBehavior\":\"0\",\"DefaultValueReg\":\"0\"},\"ch7\":{\"PauseBehavior\":\"0\",\"IdleBehavior\":\"0\",\"DefaultValueReg\":\"0\"},\"ch8\":{\"PauseBehavior\":\"0\",\"IdleBehavior\":\"0\",\"DefaultValueReg\":\"0\"},\"ch9\":{\"PauseBehavior\":\"0\",\"IdleBehavior\":\"0\",\"DefaultValueReg\":\"0\"},\"ch10\":{\"PauseBehavior\":\"0\",\"IdleBehavior\":\"0\",\"DefaultValueReg\":\"0\"},\"ch11\":{\"PauseBehavior\":\"0\",\"IdleBehavior\":\"0\",\"DefaultValueReg\":\"0\"},\"ch12\":{\"PauseBehavior\":\"0\",\"IdleBehavior\":\"0\",\"DefaultValueReg\":\"0\"},\"ch13\":{\"PauseBehavior\":\"0\",\"IdleBehavior\":\"0\",\"DefaultValueReg\":\"0\"},\"ch14\":{\"PauseBehavior\":\"0\",\"IdleBehavior\":\"0\",\"DefaultValueReg\":\"0\"},\"ch15\":{\"PauseBehavior\":\"0\",\"IdleBehavior\":\"0\",\"DefaultValueReg\":\"0\"},\"ch16\":{\"PauseBehavior\":\"0\",\"IdleBehavior\":\"0\",\"DefaultValueReg\":\"0\"},\"ch17\":{\"PauseBehavior\":\"0\",\"IdleBehavior\":\"0\",\"DefaultValueReg\":\"0\"},\"ch18\":{\"PauseBehavior\":\"0\",\"IdleBehavior\":\"0\",\"DefaultValueReg\":\"0\"},\"ch19\":{\"PauseBehavior\":\"0\",\"IdleBehavior\":\"0\",\"DefaultValueReg\":\"0\"},\"ch20\":{\"PauseBehavior\":\"0\",\"IdleBehavior\":\"0\",\"DefaultValueReg\":\"0\"},\"ch21\":{\"PauseBehavior\":\"0\",\"IdleBehavior\":\"0\",\"DefaultValueReg\":\"0\"},\"ch22\":{\"PauseBehavior\":\"0\",\"IdleBehavior\":\"0\",\"DefaultValueReg\":\"0\"},\"ch23\":{\"PauseBehavior\":\"0\",\"IdleBehavior\":\"0\",\"DefaultValueReg\":\"0\"},\"ch24\":{\"PauseBehavior\":\"0\",\"IdleBehavior\":\"0\",\"DefaultValueReg\":\"0\"},\"ch25\":{\"PauseBehavior\":\"0\",\"IdleBehavior\":\"0\",\"DefaultValueReg\":\"0\"},\"ch26\":{\"PauseBehavior\":\"0\",\"IdleBehavior\":\"0\",\"DefaultValueReg\":\"0\"},\"ch27\":{\"PauseBehavior\":\"0\",\"IdleBehavior\":\"0\",\"DefaultValueReg\":\"0\"},\"ch28\":{\"PauseBehavior\":\"0\",\"IdleBehavior\":\"0\",\"DefaultValueReg\":\"0\"},\"ch29\":{\"PauseBehavior\":\"0\",\"IdleBehavior\":\"0\",\"DefaultValueReg\":\"0\"},\"ch30\":{\"PauseBehavior\":\"0\",\"IdleBehavior\":\"0\",\"DefaultValueReg\":\"0\"},\"ch31\":{\"PauseBehavior\":\"0\",\"IdleBehavior\":\"0\",\"DefaultValueReg\":\"0\"}}}"  Slot_DV_9A="{\"dv_9A\":{\"ch0\":{\"PauseBehavior\":\"0\",\"IdleBehavior\":\"0\",\"DefaultValueReg\":\"0\"},\"ch1\":{\"PauseBehavior\":\"0\",\"IdleBehavior\":\"0\",\"DefaultValueReg\":\"0\"},\"ch2\":{\"PauseBehavior\":\"0\",\"IdleBehavior\":\"0\",\"DefaultValueReg\":\"0\"},\"ch3\":{\"PauseBehavior\":\"0\",\"IdleBehavior\":\"0\",\"DefaultValueReg\":\"0\"},\"ch4\":{\"PauseBehavior\":\"0\",\"IdleBehavior\":\"0\",\"DefaultValueReg\":\"0\"},\"ch5\":{\"PauseBehavior\":\"0\",\"IdleBehavior\":\"0\",\"DefaultValueReg\":\"0\"},\"ch6\":{\"PauseBehavior\":\"0\",\"IdleBehavior\":\"0\",\"DefaultValueReg\":\"0\"},\"ch7\":{\"PauseBehavior\":\"0\",\"IdleBehavior\":\"0\",\"DefaultValueReg\":\"0\"},\"ch8\":{\"PauseBehavior\":\"0\",\"IdleBehavior\":\"0\",\"DefaultValueReg\":\"0\"},\"ch9\":{\"PauseBehavior\":\"0\",\"IdleBehavior\":\"0\",\"DefaultValueReg\":\"0\"},\"ch10\":{\"PauseBehavior\":\"0\",\"IdleBehavior\":\"0\",\"DefaultValueReg\":\"0\"},\"ch11\":{\"PauseBehavior\":\"0\",\"IdleBehavior\":\"0\",\"DefaultValueReg\":\"0\"},\"ch12\":{\"PauseBehavior\":\"0\",\"IdleBehavior\":\"0\",\"DefaultValueReg\":\"0\"},\"ch13\":{\"PauseBehavior\":\"0\",\"IdleBehavior\":\"0\",\"DefaultValueReg\":\"0\"},\"ch14\":{\"PauseBehavior\":\"0\",\"IdleBehavior\":\"0\",\"DefaultValueReg\":\"0\"},\"ch15\":{\"PauseBehavior\":\"0\",\"IdleBehavior\":\"0\",\"DefaultValueReg\":\"0\"},\"ch16\":{\"PauseBehavior\":\"0\",\"IdleBehavior\":\"0\",\"DefaultValueReg\":\"0\"},\"ch17\":{\"PauseBehavior\":\"0\",\"IdleBehavior\":\"0\",\"DefaultValueReg\":\"0\"},\"ch18\":{\"PauseBehavior\":\"0\",\"IdleBehavior\":\"0\",\"DefaultValueReg\":\"0\"},\"ch19\":{\"PauseBehavior\":\"0\",\"IdleBehavior\":\"0\",\"DefaultValueReg\":\"0\"},\"ch20\":{\"PauseBehavior\":\"0\",\"IdleBehavior\":\"0\",\"DefaultValueReg\":\"0\"},\"ch21\":{\"PauseBehavior\":\"0\",\"IdleBehavior\":\"0\",\"DefaultValueReg\":\"0\"},\"ch22\":{\"PauseBehavior\":\"0\",\"IdleBehavior\":\"0\",\"DefaultValueReg\":\"0\"},\"ch23\":{\"PauseBehavior\":\"0\",\"IdleBehavior\":\"0\",\"DefaultValueReg\":\"0\"},\"ch24\":{\"PauseBehavior\":\"0\",\"IdleBehavior\":\"0\",\"DefaultValueReg\":\"0\"},\"ch25\":{\"PauseBehavior\":\"0\",\"IdleBehavior\":\"0\",\"DefaultValueReg\":\"0\"},\"ch26\":{\"PauseBehavior\":\"0\",\"IdleBehavior\":\"0\",\"DefaultValueReg\":\"0\"},\"ch27\":{\"PauseBehavior\":\"0\",\"IdleBehavior\":\"0\",\"DefaultValueReg\":\"0\"},\"ch28\":{\"PauseBehavior\":\"0\",\"IdleBehavior\":\"0\",\"DefaultValueReg\":\"0\"},\"ch29\":{\"PauseBehavior\":\"0\",\"IdleBehavior\":\"0\",\"DefaultValueReg\":\"0\"},\"ch30\":{\"PauseBehavior\":\"0\",\"IdleBehavior\":\"0\",\"DefaultValueReg\":\"0\"},\"ch31\":{\"PauseBehavior\":\"0\",\"IdleBehavior\":\"0\",\"DefaultValueReg\":\"0\"}}}"  Slot_DV_9B="{\"dv_9B\":{\"ch0\":{\"PauseBehavior\":\"0\",\"IdleBehavior\":\"0\",\"DefaultValueReg\":\"0\"},\"ch1\":{\"PauseBehavior\":\"0\",\"IdleBehavior\":\"0\",\"DefaultValueReg\":\"0\"},\"ch2\":{\"PauseBehavior\":\"0\",\"IdleBehavior\":\"0\",\"DefaultValueReg\":\"0\"},\"ch3\":{\"PauseBehavior\":\"0\",\"IdleBehavior\":\"0\",\"DefaultValueReg\":\"0\"},\"ch4\":{\"PauseBehavior\":\"0\",\"IdleBehavior\":\"0\",\"DefaultValueReg\":\"0\"},\"ch5\":{\"PauseBehavior\":\"0\",\"IdleBehavior\":\"0\",\"DefaultValueReg\":\"0\"},\"ch6\":{\"PauseBehavior\":\"0\",\"IdleBehavior\":\"0\",\"DefaultValueReg\":\"0\"},\"ch7\":{\"PauseBehavior\":\"0\",\"IdleBehavior\":\"0\",\"DefaultValueReg\":\"0\"},\"ch8\":{\"PauseBehavior\":\"0\",\"IdleBehavior\":\"0\",\"DefaultValueReg\":\"0\"},\"ch9\":{\"PauseBehavior\":\"0\",\"IdleBehavior\":\"0\",\"DefaultValueReg\":\"0\"},\"ch10\":{\"PauseBehavior\":\"0\",\"IdleBehavior\":\"0\",\"DefaultValueReg\":\"0\"},\"ch11\":{\"PauseBehavior\":\"0\",\"IdleBehavior\":\"0\",\"DefaultValueReg\":\"0\"},\"ch12\":{\"PauseBehavior\":\"0\",\"IdleBehavior\":\"0\",\"DefaultValueReg\":\"0\"},\"ch13\":{\"PauseBehavior\":\"0\",\"IdleBehavior\":\"0\",\"DefaultValueReg\":\"0\"},\"ch14\":{\"PauseBehavior\":\"0\",\"IdleBehavior\":\"0\",\"DefaultValueReg\":\"0\"},\"ch15\":{\"PauseBehavior\":\"0\",\"IdleBehavior\":\"0\",\"DefaultValueReg\":\"0\"},\"ch16\":{\"PauseBehavior\":\"0\",\"IdleBehavior\":\"0\",\"DefaultValueReg\":\"0\"},\"ch17\":{\"PauseBehavior\":\"0\",\"IdleBehavior\":\"0\",\"DefaultValueReg\":\"0\"},\"ch18\":{\"PauseBehavior\":\"0\",\"IdleBehavior\":\"0\",\"DefaultValueReg\":\"0\"},\"ch19\":{\"PauseBehavior\":\"0\",\"IdleBehavior\":\"0\",\"DefaultValueReg\":\"0\"},\"ch20\":{\"PauseBehavior\":\"0\",\"IdleBehavior\":\"0\",\"DefaultValueReg\":\"0\"},\"ch21\":{\"PauseBehavior\":\"0\",\"IdleBehavior\":\"0\",\"DefaultValueReg\":\"0\"},\"ch22\":{\"PauseBehavior\":\"0\",\"IdleBehavior\":\"0\",\"DefaultValueReg\":\"0\"},\"ch23\":{\"PauseBehavior\":\"0\",\"IdleBehavior\":\"0\",\"DefaultValueReg\":\"0\"},\"ch24\":{\"PauseBehavior\":\"0\",\"IdleBehavior\":\"0\",\"DefaultValueReg\":\"0\"},\"ch25\":{\"PauseBehavior\":\"0\",\"IdleBehavior\":\"0\",\"DefaultValueReg\":\"0\"},\"ch26\":{\"PauseBehavior\":\"0\",\"IdleBehavior\":\"0\",\"DefaultValueReg\":\"0\"},\"ch27\":{\"PauseBehavior\":\"0\",\"IdleBehavior\":\"0\",\"DefaultValueReg\":\"0\"},\"ch28\":{\"PauseBehavior\":\"0\",\"IdleBehavior\":\"0\",\"DefaultValueReg\":\"0\"},\"ch29\":{\"PauseBehavior\":\"0\",\"IdleBehavior\":\"0\",\"DefaultValueReg\":\"0\"},\"ch30\":{\"PauseBehavior\":\"0\",\"IdleBehavior\":\"0\",\"DefaultValueReg\":\"0\"},\"ch31\":{\"PauseBehavior\":\"0\",\"IdleBehavior\":\"0\",\"DefaultValueReg\":\"0\"}}}"  Expansion_DV_9A="{\"dv_Expansion_9A\":{\"ch0\":{\"PauseBehavior\":\"0\",\"IdleBehavior\":\"0\",\"DefaultValueReg\":\"0\"},\"ch1\":{\"PauseBehavior\":\"0\",\"IdleBehavior\":\"0\",\"DefaultValueReg\":\"0\"},\"ch2\":{\"PauseBehavior\":\"0\",\"IdleBehavior\":\"0\",\"DefaultValueReg\":\"0\"},\"ch3\":{\"PauseBehavior\":\"0\",\"IdleBehavior\":\"0\",\"DefaultValueReg\":\"0\"},\"ch4\":{\"PauseBehavior\":\"0\",\"IdleBehavior\":\"0\",\"DefaultValueReg\":\"0\"},\"ch5\":{\"PauseBehavior\":\"0\",\"IdleBehavior\":\"0\",\"DefaultValueReg\":\"0\"},\"ch6\":{\"PauseBehavior\":\"0\",\"IdleBehavior\":\"0\",\"DefaultValueReg\":\"0\"},\"ch7\":{\"PauseBehavior\":\"0\",\"IdleBehavior\":\"0\",\"DefaultValueReg\":\"0\"},\"ch8\":{\"PauseBehavior\":\"0\",\"IdleBehavior\":\"0\",\"DefaultValueReg\":\"0\"},\"ch9\":{\"PauseBehavior\":\"0\",\"IdleBehavior\":\"0\",\"DefaultValueReg\":\"0\"},\"ch10\":{\"PauseBehavior\":\"0\",\"IdleBehavior\":\"0\",\"DefaultValueReg\":\"0\"},\"ch11\":{\"PauseBehavior\":\"0\",\"IdleBehavior\":\"0\",\"DefaultValueReg\":\"0\"},\"ch12\":{\"PauseBehavior\":\"0\",\"IdleBehavior\":\"0\",\"DefaultValueReg\":\"0\"},\"ch13\":{\"PauseBehavior\":\"0\",\"IdleBehavior\":\"0\",\"DefaultValueReg\":\"0\"},\"ch14\":{\"PauseBehavior\":\"0\",\"IdleBehavior\":\"0\",\"DefaultValueReg\":\"0\"},\"ch15\":{\"PauseBehavior\":\"0\",\"IdleBehavior\":\"0\",\"DefaultValueReg\":\"0\"},\"ch16\":{\"PauseBehavior\":\"0\",\"IdleBehavior\":\"0\",\"DefaultValueReg\":\"0\"},\"ch17\":{\"PauseBehavior\":\"0\",\"IdleBehavior\":\"0\",\"DefaultValueReg\":\"0\"},\"ch18\":{\"PauseBehavior\":\"0\",\"IdleBehavior\":\"0\",\"DefaultValueReg\":\"0\"},\"ch19\":{\"PauseBehavior\":\"0\",\"IdleBehavior\":\"0\",\"DefaultValueReg\":\"0\"},\"ch20\":{\"PauseBehavior\":\"0\",\"IdleBehavior\":\"0\",\"DefaultValueReg\":\"0\"},\"ch21\":{\"PauseBehavior\":\"0\",\"IdleBehavior\":\"0\",\"DefaultValueReg\":\"0\"},\"ch22\":{\"PauseBehavior\":\"0\",\"IdleBehavior\":\"0\",\"DefaultValueReg\":\"0\"},\"ch23\":{\"PauseBehavior\":\"0\",\"IdleBehavior\":\"0\",\"DefaultValueReg\":\"0\"},\"ch24\":{\"PauseBehavior\":\"0\",\"IdleBehavior\":\"0\",\"DefaultValueReg\":\"0\"},\"ch25\":{\"PauseBehavior\":\"0\",\"IdleBehavior\":\"0\",\"DefaultValueReg\":\"0\"},\"ch26\":{\"PauseBehavior\":\"0\",\"IdleBehavior\":\"0\",\"DefaultValueReg\":\"0\"},\"ch27\":{\"PauseBehavior\":\"0\",\"IdleBehavior\":\"0\",\"DefaultValueReg\":\"0\"},\"ch28\":{\"PauseBehavior\":\"0\",\"IdleBehavior\":\"0\",\"DefaultValueReg\":\"0\"},\"ch29\":{\"PauseBehavior\":\"0\",\"IdleBehavior\":\"0\",\"DefaultValueReg\":\"0\"},\"ch30\":{\"PauseBehavior\":\"0\",\"IdleBehavior\":\"0\",\"DefaultValueReg\":\"0\"},\"ch31\":{\"PauseBehavior\":\"0\",\"IdleBehavior\":\"0\",\"DefaultValueReg\":\"0\"}}}"  Expansion_DV_9B="{\"dv_Expansion_9B\":{\"ch0\":{\"PauseBehavior\":\"0\",\"IdleBehavior\":\"0\",\"DefaultValueReg\":\"0\"},\"ch1\":{\"PauseBehavior\":\"0\",\"IdleBehavior\":\"0\",\"DefaultValueReg\":\"0\"},\"ch2\":{\"PauseBehavior\":\"0\",\"IdleBehavior\":\"0\",\"DefaultValueReg\":\"0\"},\"ch3\":{\"PauseBehavior\":\"0\",\"IdleBehavior\":\"0\",\"DefaultValueReg\":\"0\"},\"ch4\":{\"PauseBehavior\":\"0\",\"IdleBehavior\":\"0\",\"DefaultValueReg\":\"0\"},\"ch5\":{\"PauseBehavior\":\"0\",\"IdleBehavior\":\"0\",\"DefaultValueReg\":\"0\"},\"ch6\":{\"PauseBehavior\":\"0\",\"IdleBehavior\":\"0\",\"DefaultValueReg\":\"0\"},\"ch7\":{\"PauseBehavior\":\"0\",\"IdleBehavior\":\"0\",\"DefaultValueReg\":\"0\"},\"ch8\":{\"PauseBehavior\":\"0\",\"IdleBehavior\":\"0\",\"DefaultValueReg\":\"0\"},\"ch9\":{\"PauseBehavior\":\"0\",\"IdleBehavior\":\"0\",\"DefaultValueReg\":\"0\"},\"ch10\":{\"PauseBehavior\":\"0\",\"IdleBehavior\":\"0\",\"DefaultValueReg\":\"0\"},\"ch11\":{\"PauseBehavior\":\"0\",\"IdleBehavior\":\"0\",\"DefaultValueReg\":\"0\"},\"ch12\":{\"PauseBehavior\":\"0\",\"IdleBehavior\":\"0\",\"DefaultValueReg\":\"0\"},\"ch13\":{\"PauseBehavior\":\"0\",\"IdleBehavior\":\"0\",\"DefaultValueReg\":\"0\"},\"ch14\":{\"PauseBehavior\":\"0\",\"IdleBehavior\":\"0\",\"DefaultValueReg\":\"0\"},\"ch15\":{\"PauseBehavior\":\"0\",\"IdleBehavior\":\"0\",\"DefaultValueReg\":\"0\"},\"ch16\":{\"PauseBehavior\":\"0\",\"IdleBehavior\":\"0\",\"DefaultValueReg\":\"0\"},\"ch17\":{\"PauseBehavior\":\"0\",\"IdleBehavior\":\"0\",\"DefaultValueReg\":\"0\"},\"ch18\":{\"PauseBehavior\":\"0\",\"IdleBehavior\":\"0\",\"DefaultValueReg\":\"0\"},\"ch19\":{\"PauseBehavior\":\"0\",\"IdleBehavior\":\"0\",\"DefaultValueReg\":\"0\"},\"ch20\":{\"PauseBehavior\":\"0\",\"IdleBehavior\":\"0\",\"DefaultValueReg\":\"0\"},\"ch21\":{\"PauseBehavior\":\"0\",\"IdleBehavior\":\"0\",\"DefaultValueReg\":\"0\"},\"ch22\":{\"PauseBehavior\":\"0\",\"IdleBehavior\":\"0\",\"DefaultValueReg\":\"0\"},\"ch23\":{\"PauseBehavior\":\"0\",\"IdleBehavior\":\"0\",\"DefaultValueReg\":\"0\"},\"ch24\":{\"PauseBehavior\":\"0\",\"IdleBehavior\":\"0\",\"DefaultValueReg\":\"0\"},\"ch25\":{\"PauseBehavior\":\"0\",\"IdleBehavior\":\"0\",\"DefaultValueReg\":\"0\"},\"ch26\":{\"PauseBehavior\":\"0\",\"IdleBehavior\":\"0\",\"DefaultValueReg\":\"0\"},\"ch27\":{\"PauseBehavior\":\"0\",\"IdleBehavior\":\"0\",\"DefaultValueReg\":\"0\"},\"ch28\":{\"PauseBehavior\":\"0\",\"IdleBehavior\":\"0\",\"DefaultValueReg\":\"0\"},\"ch29\":{\"PauseBehavior\":\"0\",\"IdleBehavior\":\"0\",\"DefaultValueReg\":\"0\"},\"ch30\":{\"PauseBehavior\":\"0\",\"IdleBehavior\":\"0\",\"DefaultValueReg\":\"0\"},\"ch31\":{\"PauseBehavior\":\"0\",\"IdleBehavior\":\"0\",\"DefaultValueReg\":\"0\"}}}"  Slot_DV_8A="{\"dv_8A\":{\"ch0\":{\"PauseBehavior\":\"0\",\"IdleBehavior\":\"0\",\"DefaultValueReg\":\"0\"},\"ch1\":{\"PauseBehavior\":\"0\",\"IdleBehavior\":\"0\",\"DefaultValueReg\":\"0\"},\"ch2\":{\"PauseBehavior\":\"0\",\"IdleBehavior\":\"0\",\"DefaultValueReg\":\"0\"},\"ch3\":{\"PauseBehavior\":\"0\",\"IdleBehavior\":\"0\",\"DefaultValueReg\":\"0\"},\"ch4\":{\"PauseBehavior\":\"0\",\"IdleBehavior\":\"0\",\"DefaultValueReg\":\"0\"},\"ch5\":{\"PauseBehavior\":\"0\",\"IdleBehavior\":\"0\",\"DefaultValueReg\":\"0\"},\"ch6\":{\"PauseBehavior\":\"0\",\"IdleBehavior\":\"0\",\"DefaultValueReg\":\"0\"},\"ch7\":{\"PauseBehavior\":\"0\",\"IdleBehavior\":\"0\",\"DefaultValueReg\":\"0\"},\"ch8\":{\"PauseBehavior\":\"0\",\"IdleBehavior\":\"0\",\"DefaultValueReg\":\"0\"},\"ch9\":{\"PauseBehavior\":\"0\",\"IdleBehavior\":\"0\",\"DefaultValueReg\":\"0\"},\"ch10\":{\"PauseBehavior\":\"0\",\"IdleBehavior\":\"0\",\"DefaultValueReg\":\"0\"},\"ch11\":{\"PauseBehavior\":\"0\",\"IdleBehavior\":\"0\",\"DefaultValueReg\":\"0\"},\"ch12\":{\"PauseBehavior\":\"0\",\"IdleBehavior\":\"0\",\"DefaultValueReg\":\"0\"},\"ch13\":{\"PauseBehavior\":\"0\",\"IdleBehavior\":\"0\",\"DefaultValueReg\":\"0\"},\"ch14\":{\"PauseBehavior\":\"0\",\"IdleBehavior\":\"0\",\"DefaultValueReg\":\"0\"},\"ch15\":{\"PauseBehavior\":\"0\",\"IdleBehavior\":\"0\",\"DefaultValueReg\":\"0\"},\"ch16\":{\"PauseBehavior\":\"0\",\"IdleBehavior\":\"0\",\"DefaultValueReg\":\"0\"},\"ch17\":{\"PauseBehavior\":\"0\",\"IdleBehavior\":\"0\",\"DefaultValueReg\":\"0\"},\"ch18\":{\"PauseBehavior\":\"0\",\"IdleBehavior\":\"0\",\"DefaultValueReg\":\"0\"},\"ch19\":{\"PauseBehavior\":\"0\",\"IdleBehavior\":\"0\",\"DefaultValueReg\":\"0\"},\"ch20\":{\"PauseBehavior\":\"0\",\"IdleBehavior\":\"0\",\"DefaultValueReg\":\"0\"},\"ch21\":{\"PauseBehavior\":\"0\",\"IdleBehavior\":\"0\",\"DefaultValueReg\":\"0\"},\"ch22\":{\"PauseBehavior\":\"0\",\"IdleBehavior\":\"0\",\"DefaultValueReg\":\"0\"},\"ch23\":{\"PauseBehavior\":\"0\",\"IdleBehavior\":\"0\",\"DefaultValueReg\":\"0\"},\"ch24\":{\"PauseBehavior\":\"0\",\"IdleBehavior\":\"0\",\"DefaultValueReg\":\"0\"},\"ch25\":{\"PauseBehavior\":\"0\",\"IdleBehavior\":\"0\",\"DefaultValueReg\":\"0\"},\"ch26\":{\"PauseBehavior\":\"0\",\"IdleBehavior\":\"0\",\"DefaultValueReg\":\"0\"},\"ch27\":{\"PauseBehavior\":\"0\",\"IdleBehavior\":\"0\",\"DefaultValueReg\":\"0\"},\"ch28\":{\"PauseBehavior\":\"0\",\"IdleBehavior\":\"0\",\"DefaultValueReg\":\"0\"},\"ch29\":{\"PauseBehavior\":\"0\",\"IdleBehavior\":\"0\",\"DefaultValueReg\":\"0\"},\"ch30\":{\"PauseBehavior\":\"0\",\"IdleBehavior\":\"0\",\"DefaultValueReg\":\"0\"},\"ch31\":{\"PauseBehavior\":\"0\",\"IdleBehavior\":\"0\",\"DefaultValueReg\":\"0\"}}}"  Slot_DV_8B="{\"dv_8B\":{\"ch0\":{\"PauseBehavior\":\"0\",\"IdleBehavior\":\"0\",\"DefaultValueReg\":\"0\"},\"ch1\":{\"PauseBehavior\":\"0\",\"IdleBehavior\":\"0\",\"DefaultValueReg\":\"0\"},\"ch2\":{\"PauseBehavior\":\"0\",\"IdleBehavior\":\"0\",\"DefaultValueReg\":\"0\"},\"ch3\":{\"PauseBehavior\":\"0\",\"IdleBehavior\":\"0\",\"DefaultValueReg\":\"0\"},\"ch4\":{\"PauseBehavior\":\"0\",\"IdleBehavior\":\"0\",\"DefaultValueReg\":\"0\"},\"ch5\":{\"PauseBehavior\":\"0\",\"IdleBehavior\":\"0\",\"DefaultValueReg\":\"0\"},\"ch6\":{\"PauseBehavior\":\"0\",\"IdleBehavior\":\"0\",\"DefaultValueReg\":\"0\"},\"ch7\":{\"PauseBehavior\":\"0\",\"IdleBehavior\":\"0\",\"DefaultValueReg\":\"0\"},\"ch8\":{\"PauseBehavior\":\"0\",\"IdleBehavior\":\"0\",\"DefaultValueReg\":\"0\"},\"ch9\":{\"PauseBehavior\":\"0\",\"IdleBehavior\":\"0\",\"DefaultValueReg\":\"0\"},\"ch10\":{\"PauseBehavior\":\"0\",\"IdleBehavior\":\"0\",\"DefaultValueReg\":\"0\"},\"ch11\":{\"PauseBehavior\":\"0\",\"IdleBehavior\":\"0\",\"DefaultValueReg\":\"0\"},\"ch12\":{\"PauseBehavior\":\"0\",\"IdleBehavior\":\"0\",\"DefaultValueReg\":\"0\"},\"ch13\":{\"PauseBehavior\":\"0\",\"IdleBehavior\":\"0\",\"DefaultValueReg\":\"0\"},\"ch14\":{\"PauseBehavior\":\"0\",\"IdleBehavior\":\"0\",\"DefaultValueReg\":\"0\"},\"ch15\":{\"PauseBehavior\":\"0\",\"IdleBehavior\":\"0\",\"DefaultValueReg\":\"0\"},\"ch16\":{\"PauseBehavior\":\"0\",\"IdleBehavior\":\"0\",\"DefaultValueReg\":\"0\"},\"ch17\":{\"PauseBehavior\":\"0\",\"IdleBehavior\":\"0\",\"DefaultValueReg\":\"0\"},\"ch18\":{\"PauseBehavior\":\"0\",\"IdleBehavior\":\"0\",\"DefaultValueReg\":\"0\"},\"ch19\":{\"PauseBehavior\":\"0\",\"IdleBehavior\":\"0\",\"DefaultValueReg\":\"0\"},\"ch20\":{\"PauseBehavior\":\"0\",\"IdleBehavior\":\"0\",\"DefaultValueReg\":\"0\"},\"ch21\":{\"PauseBehavior\":\"0\",\"IdleBehavior\":\"0\",\"DefaultValueReg\":\"0\"},\"ch22\":{\"PauseBehavior\":\"0\",\"IdleBehavior\":\"0\",\"DefaultValueReg\":\"0\"},\"ch23\":{\"PauseBehavior\":\"0\",\"IdleBehavior\":\"0\",\"DefaultValueReg\":\"0\"},\"ch24\":{\"PauseBehavior\":\"0\",\"IdleBehavior\":\"0\",\"DefaultValueReg\":\"0\"},\"ch25\":{\"PauseBehavior\":\"0\",\"IdleBehavior\":\"0\",\"DefaultValueReg\":\"0\"},\"ch26\":{\"PauseBehavior\":\"0\",\"IdleBehavior\":\"0\",\"DefaultValueReg\":\"0\"},\"ch27\":{\"PauseBehavior\":\"0\",\"IdleBehavior\":\"0\",\"DefaultValueReg\":\"0\"},\"ch28\":{\"PauseBehavior\":\"0\",\"IdleBehavior\":\"0\",\"DefaultValueReg\":\"0\"},\"ch29\":{\"PauseBehavior\":\"0\",\"IdleBehavior\":\"0\",\"DefaultValueReg\":\"0\"},\"ch30\":{\"PauseBehavior\":\"0\",\"IdleBehavior\":\"0\",\"DefaultValueReg\":\"0\"},\"ch31\":{\"PauseBehavior\":\"0\",\"IdleBehavior\":\"0\",\"DefaultValueReg\":\"0\"}}}"  Expansion_DV_8A="{\"dv_Expansion_8A\":{\"ch0\":{\"PauseBehavior\":\"0\",\"IdleBehavior\":\"0\",\"DefaultValueReg\":\"0\"},\"ch1\":{\"PauseBehavior\":\"0\",\"IdleBehavior\":\"0\",\"DefaultValueReg\":\"0\"},\"ch2\":{\"PauseBehavior\":\"0\",\"IdleBehavior\":\"0\",\"DefaultValueReg\":\"0\"},\"ch3\":{\"PauseBehavior\":\"0\",\"IdleBehavior\":\"0\",\"DefaultValueReg\":\"0\"},\"ch4\":{\"PauseBehavior\":\"0\",\"IdleBehavior\":\"0\",\"DefaultValueReg\":\"0\"},\"ch5\":{\"PauseBehavior\":\"0\",\"IdleBehavior\":\"0\",\"DefaultValueReg\":\"0\"},\"ch6\":{\"PauseBehavior\":\"0\",\"IdleBehavior\":\"0\",\"DefaultValueReg\":\"0\"},\"ch7\":{\"PauseBehavior\":\"0\",\"IdleBehavior\":\"0\",\"DefaultValueReg\":\"0\"},\"ch8\":{\"PauseBehavior\":\"0\",\"IdleBehavior\":\"0\",\"DefaultValueReg\":\"0\"},\"ch9\":{\"PauseBehavior\":\"0\",\"IdleBehavior\":\"0\",\"DefaultValueReg\":\"0\"},\"ch10\":{\"PauseBehavior\":\"0\",\"IdleBehavior\":\"0\",\"DefaultValueReg\":\"0\"},\"ch11\":{\"PauseBehavior\":\"0\",\"IdleBehavior\":\"0\",\"DefaultValueReg\":\"0\"},\"ch12\":{\"PauseBehavior\":\"0\",\"IdleBehavior\":\"0\",\"DefaultValueReg\":\"0\"},\"ch13\":{\"PauseBehavior\":\"0\",\"IdleBehavior\":\"0\",\"DefaultValueReg\":\"0\"},\"ch14\":{\"PauseBehavior\":\"0\",\"IdleBehavior\":\"0\",\"DefaultValueReg\":\"0\"},\"ch15\":{\"PauseBehavior\":\"0\",\"IdleBehavior\":\"0\",\"DefaultValueReg\":\"0\"},\"ch16\":{\"PauseBehavior\":\"0\",\"IdleBehavior\":\"0\",\"DefaultValueReg\":\"0\"},\"ch17\":{\"PauseBehavior\":\"0\",\"IdleBehavior\":\"0\",\"DefaultValueReg\":\"0\"},\"ch18\":{\"PauseBehavior\":\"0\",\"IdleBehavior\":\"0\",\"DefaultValueReg\":\"0\"},\"ch19\":{\"PauseBehavior\":\"0\",\"IdleBehavior\":\"0\",\"DefaultValueReg\":\"0\"},\"ch20\":{\"PauseBehavior\":\"0\",\"IdleBehavior\":\"0\",\"DefaultValueReg\":\"0\"},\"ch21\":{\"PauseBehavior\":\"0\",\"IdleBehavior\":\"0\",\"DefaultValueReg\":\"0\"},\"ch22\":{\"PauseBehavior\":\"0\",\"IdleBehavior\":\"0\",\"DefaultValueReg\":\"0\"},\"ch23\":{\"PauseBehavior\":\"0\",\"IdleBehavior\":\"0\",\"DefaultValueReg\":\"0\"},\"ch24\":{\"PauseBehavior\":\"0\",\"IdleBehavior\":\"0\",\"DefaultValueReg\":\"0\"},\"ch25\":{\"PauseBehavior\":\"0\",\"IdleBehavior\":\"0\",\"DefaultValueReg\":\"0\"},\"ch26\":{\"PauseBehavior\":\"0\",\"IdleBehavior\":\"0\",\"DefaultValueReg\":\"0\"},\"ch27\":{\"PauseBehavior\":\"0\",\"IdleBehavior\":\"0\",\"DefaultValueReg\":\"0\"},\"ch28\":{\"PauseBehavior\":\"0\",\"IdleBehavior\":\"0\",\"DefaultValueReg\":\"0\"},\"ch29\":{\"PauseBehavior\":\"0\",\"IdleBehavior\":\"0\",\"DefaultValueReg\":\"0\"},\"ch30\":{\"PauseBehavior\":\"0\",\"IdleBehavior\":\"0\",\"DefaultValueReg\":\"0\"},\"ch31\":{\"PauseBehavior\":\"0\",\"IdleBehavior\":\"0\",\"DefaultValueReg\":\"0\"}}}"  Expansion_DV_8B="{\"dv_Expansion_8B\":{\"ch0\":{\"PauseBehavior\":\"0\",\"IdleBehavior\":\"0\",\"DefaultValueReg\":\"0\"},\"ch1\":{\"PauseBehavior\":\"0\",\"IdleBehavior\":\"0\",\"DefaultValueReg\":\"0\"},\"ch2\":{\"PauseBehavior\":\"0\",\"IdleBehavior\":\"0\",\"DefaultValueReg\":\"0\"},\"ch3\":{\"PauseBehavior\":\"0\",\"IdleBehavior\":\"0\",\"DefaultValueReg\":\"0\"},\"ch4\":{\"PauseBehavior\":\"0\",\"IdleBehavior\":\"0\",\"DefaultValueReg\":\"0\"},\"ch5\":{\"PauseBehavior\":\"0\",\"IdleBehavior\":\"0\",\"DefaultValueReg\":\"0\"},\"ch6\":{\"PauseBehavior\":\"0\",\"IdleBehavior\":\"0\",\"DefaultValueReg\":\"0\"},\"ch7\":{\"PauseBehavior\":\"0\",\"IdleBehavior\":\"0\",\"DefaultValueReg\":\"0\"},\"ch8\":{\"PauseBehavior\":\"0\",\"IdleBehavior\":\"0\",\"DefaultValueReg\":\"0\"},\"ch9\":{\"PauseBehavior\":\"0\",\"IdleBehavior\":\"0\",\"DefaultValueReg\":\"0\"},\"ch10\":{\"PauseBehavior\":\"0\",\"IdleBehavior\":\"0\",\"DefaultValueReg\":\"0\"},\"ch11\":{\"PauseBehavior\":\"0\",\"IdleBehavior\":\"0\",\"DefaultValueReg\":\"0\"},\"ch12\":{\"PauseBehavior\":\"0\",\"IdleBehavior\":\"0\",\"DefaultValueReg\":\"0\"},\"ch13\":{\"PauseBehavior\":\"0\",\"IdleBehavior\":\"0\",\"DefaultValueReg\":\"0\"},\"ch14\":{\"PauseBehavior\":\"0\",\"IdleBehavior\":\"0\",\"DefaultValueReg\":\"0\"},\"ch15\":{\"PauseBehavior\":\"0\",\"IdleBehavior\":\"0\",\"DefaultValueReg\":\"0\"},\"ch16\":{\"PauseBehavior\":\"0\",\"IdleBehavior\":\"0\",\"DefaultValueReg\":\"0\"},\"ch17\":{\"PauseBehavior\":\"0\",\"IdleBehavior\":\"0\",\"DefaultValueReg\":\"0\"},\"ch18\":{\"PauseBehavior\":\"0\",\"IdleBehavior\":\"0\",\"DefaultValueReg\":\"0\"},\"ch19\":{\"PauseBehavior\":\"0\",\"IdleBehavior\":\"0\",\"DefaultValueReg\":\"0\"},\"ch20\":{\"PauseBehavior\":\"0\",\"IdleBehavior\":\"0\",\"DefaultValueReg\":\"0\"},\"ch21\":{\"PauseBehavior\":\"0\",\"IdleBehavior\":\"0\",\"DefaultValueReg\":\"0\"},\"ch22\":{\"PauseBehavior\":\"0\",\"IdleBehavior\":\"0\",\"DefaultValueReg\":\"0\"},\"ch23\":{\"PauseBehavior\":\"0\",\"IdleBehavior\":\"0\",\"DefaultValueReg\":\"0\"},\"ch24\":{\"PauseBehavior\":\"0\",\"IdleBehavior\":\"0\",\"DefaultValueReg\":\"0\"},\"ch25\":{\"PauseBehavior\":\"0\",\"IdleBehavior\":\"0\",\"DefaultValueReg\":\"0\"},\"ch26\":{\"PauseBehavior\":\"0\",\"IdleBehavior\":\"0\",\"DefaultValueReg\":\"0\"},\"ch27\":{\"PauseBehavior\":\"0\",\"IdleBehavior\":\"0\",\"DefaultValueReg\":\"0\"},\"ch28\":{\"PauseBehavior\":\"0\",\"IdleBehavior\":\"0\",\"DefaultValueReg\":\"0\"},\"ch29\":{\"PauseBehavior\":\"0\",\"IdleBehavior\":\"0\",\"DefaultValueReg\":\"0\"},\"ch30\":{\"PauseBehavior\":\"0\",\"IdleBehavior\":\"0\",\"DefaultValueReg\":\"0\"},\"ch31\":{\"PauseBehavior\":\"0\",\"IdleBehavior\":\"0\",\"DefaultValueReg\":\"0\"}}}"  Slot_DV_7A="{\"dv_7A\":{\"ch0\":{\"PauseBehavior\":\"0\",\"IdleBehavior\":\"0\",\"DefaultValueReg\":\"0\"},\"ch1\":{\"PauseBehavior\":\"0\",\"IdleBehavior\":\"0\",\"DefaultValueReg\":\"0\"},\"ch2\":{\"PauseBehavior\":\"0\",\"IdleBehavior\":\"0\",\"DefaultValueReg\":\"0\"},\"ch3\":{\"PauseBehavior\":\"0\",\"IdleBehavior\":\"0\",\"DefaultValueReg\":\"0\"},\"ch4\":{\"PauseBehavior\":\"0\",\"IdleBehavior\":\"0\",\"DefaultValueReg\":\"0\"},\"ch5\":{\"PauseBehavior\":\"0\",\"IdleBehavior\":\"0\",\"DefaultValueReg\":\"0\"},\"ch6\":{\"PauseBehavior\":\"0\",\"IdleBehavior\":\"0\",\"DefaultValueReg\":\"0\"},\"ch7\":{\"PauseBehavior\":\"0\",\"IdleBehavior\":\"0\",\"DefaultValueReg\":\"0\"},\"ch8\":{\"PauseBehavior\":\"0\",\"IdleBehavior\":\"0\",\"DefaultValueReg\":\"0\"},\"ch9\":{\"PauseBehavior\":\"0\",\"IdleBehavior\":\"0\",\"DefaultValueReg\":\"0\"},\"ch10\":{\"PauseBehavior\":\"0\",\"IdleBehavior\":\"0\",\"DefaultValueReg\":\"0\"},\"ch11\":{\"PauseBehavior\":\"0\",\"IdleBehavior\":\"0\",\"DefaultValueReg\":\"0\"},\"ch12\":{\"PauseBehavior\":\"0\",\"IdleBehavior\":\"0\",\"DefaultValueReg\":\"0\"},\"ch13\":{\"PauseBehavior\":\"0\",\"IdleBehavior\":\"0\",\"DefaultValueReg\":\"0\"},\"ch14\":{\"PauseBehavior\":\"0\",\"IdleBehavior\":\"0\",\"DefaultValueReg\":\"0\"},\"ch15\":{\"PauseBehavior\":\"0\",\"IdleBehavior\":\"0\",\"DefaultValueReg\":\"0\"},\"ch16\":{\"PauseBehavior\":\"0\",\"IdleBehavior\":\"0\",\"DefaultValueReg\":\"0\"},\"ch17\":{\"PauseBehavior\":\"0\",\"IdleBehavior\":\"0\",\"DefaultValueReg\":\"0\"},\"ch18\":{\"PauseBehavior\":\"0\",\"IdleBehavior\":\"0\",\"DefaultValueReg\":\"0\"},\"ch19\":{\"PauseBehavior\":\"0\",\"IdleBehavior\":\"0\",\"DefaultValueReg\":\"0\"},\"ch20\":{\"PauseBehavior\":\"0\",\"IdleBehavior\":\"0\",\"DefaultValueReg\":\"0\"},\"ch21\":{\"PauseBehavior\":\"0\",\"IdleBehavior\":\"0\",\"DefaultValueReg\":\"0\"},\"ch22\":{\"PauseBehavior\":\"0\",\"IdleBehavior\":\"0\",\"DefaultValueReg\":\"0\"},\"ch23\":{\"PauseBehavior\":\"0\",\"IdleBehavior\":\"0\",\"DefaultValueReg\":\"0\"},\"ch24\":{\"PauseBehavior\":\"0\",\"IdleBehavior\":\"0\",\"DefaultValueReg\":\"0\"},\"ch25\":{\"PauseBehavior\":\"0\",\"IdleBehavior\":\"0\",\"DefaultValueReg\":\"0\"},\"ch26\":{\"PauseBehavior\":\"0\",\"IdleBehavior\":\"0\",\"DefaultValueReg\":\"0\"},\"ch27\":{\"PauseBehavior\":\"0\",\"IdleBehavior\":\"0\",\"DefaultValueReg\":\"0\"},\"ch28\":{\"PauseBehavior\":\"0\",\"IdleBehavior\":\"0\",\"DefaultValueReg\":\"0\"},\"ch29\":{\"PauseBehavior\":\"0\",\"IdleBehavior\":\"0\",\"DefaultValueReg\":\"0\"},\"ch30\":{\"PauseBehavior\":\"0\",\"IdleBehavior\":\"0\",\"DefaultValueReg\":\"0\"},\"ch31\":{\"PauseBehavior\":\"0\",\"IdleBehavior\":\"0\",\"DefaultValueReg\":\"0\"}}}"  Slot_DV_7B="{\"dv_7B\":{\"ch0\":{\"PauseBehavior\":\"0\",\"IdleBehavior\":\"0\",\"DefaultValueReg\":\"0\"},\"ch1\":{\"PauseBehavior\":\"0\",\"IdleBehavior\":\"0\",\"DefaultValueReg\":\"0\"},\"ch2\":{\"PauseBehavior\":\"0\",\"IdleBehavior\":\"0\",\"DefaultValueReg\":\"0\"},\"ch3\":{\"PauseBehavior\":\"0\",\"IdleBehavior\":\"0\",\"DefaultValueReg\":\"0\"},\"ch4\":{\"PauseBehavior\":\"0\",\"IdleBehavior\":\"0\",\"DefaultValueReg\":\"0\"},\"ch5\":{\"PauseBehavior\":\"0\",\"IdleBehavior\":\"0\",\"DefaultValueReg\":\"0\"},\"ch6\":{\"PauseBehavior\":\"0\",\"IdleBehavior\":\"0\",\"DefaultValueReg\":\"0\"},\"ch7\":{\"PauseBehavior\":\"0\",\"IdleBehavior\":\"0\",\"DefaultValueReg\":\"0\"},\"ch8\":{\"PauseBehavior\":\"0\",\"IdleBehavior\":\"0\",\"DefaultValueReg\":\"0\"},\"ch9\":{\"PauseBehavior\":\"0\",\"IdleBehavior\":\"0\",\"DefaultValueReg\":\"0\"},\"ch10\":{\"PauseBehavior\":\"0\",\"IdleBehavior\":\"0\",\"DefaultValueReg\":\"0\"},\"ch11\":{\"PauseBehavior\":\"0\",\"IdleBehavior\":\"0\",\"DefaultValueReg\":\"0\"},\"ch12\":{\"PauseBehavior\":\"0\",\"IdleBehavior\":\"0\",\"DefaultValueReg\":\"0\"},\"ch13\":{\"PauseBehavior\":\"0\",\"IdleBehavior\":\"0\",\"DefaultValueReg\":\"0\"},\"ch14\":{\"PauseBehavior\":\"0\",\"IdleBehavior\":\"0\",\"DefaultValueReg\":\"0\"},\"ch15\":{\"PauseBehavior\":\"0\",\"IdleBehavior\":\"0\",\"DefaultValueReg\":\"0\"},\"ch16\":{\"PauseBehavior\":\"0\",\"IdleBehavior\":\"0\",\"DefaultValueReg\":\"0\"},\"ch17\":{\"PauseBehavior\":\"0\",\"IdleBehavior\":\"0\",\"DefaultValueReg\":\"0\"},\"ch18\":{\"PauseBehavior\":\"0\",\"IdleBehavior\":\"0\",\"DefaultValueReg\":\"0\"},\"ch19\":{\"PauseBehavior\":\"0\",\"IdleBehavior\":\"0\",\"DefaultValueReg\":\"0\"},\"ch20\":{\"PauseBehavior\":\"0\",\"IdleBehavior\":\"0\",\"DefaultValueReg\":\"0\"},\"ch21\":{\"PauseBehavior\":\"0\",\"IdleBehavior\":\"0\",\"DefaultValueReg\":\"0\"},\"ch22\":{\"PauseBehavior\":\"0\",\"IdleBehavior\":\"0\",\"DefaultValueReg\":\"0\"},\"ch23\":{\"PauseBehavior\":\"0\",\"IdleBehavior\":\"0\",\"DefaultValueReg\":\"0\"},\"ch24\":{\"PauseBehavior\":\"0\",\"IdleBehavior\":\"0\",\"DefaultValueReg\":\"0\"},\"ch25\":{\"PauseBehavior\":\"0\",\"IdleBehavior\":\"0\",\"DefaultValueReg\":\"0\"},\"ch26\":{\"PauseBehavior\":\"0\",\"IdleBehavior\":\"0\",\"DefaultValueReg\":\"0\"},\"ch27\":{\"PauseBehavior\":\"0\",\"IdleBehavior\":\"0\",\"DefaultValueReg\":\"0\"},\"ch28\":{\"PauseBehavior\":\"0\",\"IdleBehavior\":\"0\",\"DefaultValueReg\":\"0\"},\"ch29\":{\"PauseBehavior\":\"0\",\"IdleBehavior\":\"0\",\"DefaultValueReg\":\"0\"},\"ch30\":{\"PauseBehavior\":\"0\",\"IdleBehavior\":\"0\",\"DefaultValueReg\":\"0\"},\"ch31\":{\"PauseBehavior\":\"0\",\"IdleBehavior\":\"0\",\"DefaultValueReg\":\"0\"}}}"  Expansion_DV_7A="{\"dv_Expansion_7A\":{\"ch0\":{\"PauseBehavior\":\"0\",\"IdleBehavior\":\"0\",\"DefaultValueReg\":\"0\"},\"ch1\":{\"PauseBehavior\":\"0\",\"IdleBehavior\":\"0\",\"DefaultValueReg\":\"0\"},\"ch2\":{\"PauseBehavior\":\"0\",\"IdleBehavior\":\"0\",\"DefaultValueReg\":\"0\"},\"ch3\":{\"PauseBehavior\":\"0\",\"IdleBehavior\":\"0\",\"DefaultValueReg\":\"0\"},\"ch4\":{\"PauseBehavior\":\"0\",\"IdleBehavior\":\"0\",\"DefaultValueReg\":\"0\"},\"ch5\":{\"PauseBehavior\":\"0\",\"IdleBehavior\":\"0\",\"DefaultValueReg\":\"0\"},\"ch6\":{\"PauseBehavior\":\"0\",\"IdleBehavior\":\"0\",\"DefaultValueReg\":\"0\"},\"ch7\":{\"PauseBehavior\":\"0\",\"IdleBehavior\":\"0\",\"DefaultValueReg\":\"0\"},\"ch8\":{\"PauseBehavior\":\"0\",\"IdleBehavior\":\"0\",\"DefaultValueReg\":\"0\"},\"ch9\":{\"PauseBehavior\":\"0\",\"IdleBehavior\":\"0\",\"DefaultValueReg\":\"0\"},\"ch10\":{\"PauseBehavior\":\"0\",\"IdleBehavior\":\"0\",\"DefaultValueReg\":\"0\"},\"ch11\":{\"PauseBehavior\":\"0\",\"IdleBehavior\":\"0\",\"DefaultValueReg\":\"0\"},\"ch12\":{\"PauseBehavior\":\"0\",\"IdleBehavior\":\"0\",\"DefaultValueReg\":\"0\"},\"ch13\":{\"PauseBehavior\":\"0\",\"IdleBehavior\":\"0\",\"DefaultValueReg\":\"0\"},\"ch14\":{\"PauseBehavior\":\"0\",\"IdleBehavior\":\"0\",\"DefaultValueReg\":\"0\"},\"ch15\":{\"PauseBehavior\":\"0\",\"IdleBehavior\":\"0\",\"DefaultValueReg\":\"0\"},\"ch16\":{\"PauseBehavior\":\"0\",\"IdleBehavior\":\"0\",\"DefaultValueReg\":\"0\"},\"ch17\":{\"PauseBehavior\":\"0\",\"IdleBehavior\":\"0\",\"DefaultValueReg\":\"0\"},\"ch18\":{\"PauseBehavior\":\"0\",\"IdleBehavior\":\"0\",\"DefaultValueReg\":\"0\"},\"ch19\":{\"PauseBehavior\":\"0\",\"IdleBehavior\":\"0\",\"DefaultValueReg\":\"0\"},\"ch20\":{\"PauseBehavior\":\"0\",\"IdleBehavior\":\"0\",\"DefaultValueReg\":\"0\"},\"ch21\":{\"PauseBehavior\":\"0\",\"IdleBehavior\":\"0\",\"DefaultValueReg\":\"0\"},\"ch22\":{\"PauseBehavior\":\"0\",\"IdleBehavior\":\"0\",\"DefaultValueReg\":\"0\"},\"ch23\":{\"PauseBehavior\":\"0\",\"IdleBehavior\":\"0\",\"DefaultValueReg\":\"0\"},\"ch24\":{\"PauseBehavior\":\"0\",\"IdleBehavior\":\"0\",\"DefaultValueReg\":\"0\"},\"ch25\":{\"PauseBehavior\":\"0\",\"IdleBehavior\":\"0\",\"DefaultValueReg\":\"0\"},\"ch26\":{\"PauseBehavior\":\"0\",\"IdleBehavior\":\"0\",\"DefaultValueReg\":\"0\"},\"ch27\":{\"PauseBehavior\":\"0\",\"IdleBehavior\":\"0\",\"DefaultValueReg\":\"0\"},\"ch28\":{\"PauseBehavior\":\"0\",\"IdleBehavior\":\"0\",\"DefaultValueReg\":\"0\"},\"ch29\":{\"PauseBehavior\":\"0\",\"IdleBehavior\":\"0\",\"DefaultValueReg\":\"0\"},\"ch30\":{\"PauseBehavior\":\"0\",\"IdleBehavior\":\"0\",\"DefaultValueReg\":\"0\"},\"ch31\":{\"PauseBehavior\":\"0\",\"IdleBehavior\":\"0\",\"DefaultValueReg\":\"0\"}}}"  Expansion_DV_7B="{\"dv_Expansion_7B\":{\"ch0\":{\"PauseBehavior\":\"0\",\"IdleBehavior\":\"0\",\"DefaultValueReg\":\"0\"},\"ch1\":{\"PauseBehavior\":\"0\",\"IdleBehavior\":\"0\",\"DefaultValueReg\":\"0\"},\"ch2\":{\"PauseBehavior\":\"0\",\"IdleBehavior\":\"0\",\"DefaultValueReg\":\"0\"},\"ch3\":{\"PauseBehavior\":\"0\",\"IdleBehavior\":\"0\",\"DefaultValueReg\":\"0\"},\"ch4\":{\"PauseBehavior\":\"0\",\"IdleBehavior\":\"0\",\"DefaultValueReg\":\"0\"},\"ch5\":{\"PauseBehavior\":\"0\",\"IdleBehavior\":\"0\",\"DefaultValueReg\":\"0\"},\"ch6\":{\"PauseBehavior\":\"0\",\"IdleBehavior\":\"0\",\"DefaultValueReg\":\"0\"},\"ch7\":{\"PauseBehavior\":\"0\",\"IdleBehavior\":\"0\",\"DefaultValueReg\":\"0\"},\"ch8\":{\"PauseBehavior\":\"0\",\"IdleBehavior\":\"0\",\"DefaultValueReg\":\"0\"},\"ch9\":{\"PauseBehavior\":\"0\",\"IdleBehavior\":\"0\",\"DefaultValueReg\":\"0\"},\"ch10\":{\"PauseBehavior\":\"0\",\"IdleBehavior\":\"0\",\"DefaultValueReg\":\"0\"},\"ch11\":{\"PauseBehavior\":\"0\",\"IdleBehavior\":\"0\",\"DefaultValueReg\":\"0\"},\"ch12\":{\"PauseBehavior\":\"0\",\"IdleBehavior\":\"0\",\"DefaultValueReg\":\"0\"},\"ch13\":{\"PauseBehavior\":\"0\",\"IdleBehavior\":\"0\",\"DefaultValueReg\":\"0\"},\"ch14\":{\"PauseBehavior\":\"0\",\"IdleBehavior\":\"0\",\"DefaultValueReg\":\"0\"},\"ch15\":{\"PauseBehavior\":\"0\",\"IdleBehavior\":\"0\",\"DefaultValueReg\":\"0\"},\"ch16\":{\"PauseBehavior\":\"0\",\"IdleBehavior\":\"0\",\"DefaultValueReg\":\"0\"},\"ch17\":{\"PauseBehavior\":\"0\",\"IdleBehavior\":\"0\",\"DefaultValueReg\":\"0\"},\"ch18\":{\"PauseBehavior\":\"0\",\"IdleBehavior\":\"0\",\"DefaultValueReg\":\"0\"},\"ch19\":{\"PauseBehavior\":\"0\",\"IdleBehavior\":\"0\",\"DefaultValueReg\":\"0\"},\"ch20\":{\"PauseBehavior\":\"0\",\"IdleBehavior\":\"0\",\"DefaultValueReg\":\"0\"},\"ch21\":{\"PauseBehavior\":\"0\",\"IdleBehavior\":\"0\",\"DefaultValueReg\":\"0\"},\"ch22\":{\"PauseBehavior\":\"0\",\"IdleBehavior\":\"0\",\"DefaultValueReg\":\"0\"},\"ch23\":{\"PauseBehavior\":\"0\",\"IdleBehavior\":\"0\",\"DefaultValueReg\":\"0\"},\"ch24\":{\"PauseBehavior\":\"0\",\"IdleBehavior\":\"0\",\"DefaultValueReg\":\"0\"},\"ch25\":{\"PauseBehavior\":\"0\",\"IdleBehavior\":\"0\",\"DefaultValueReg\":\"0\"},\"ch26\":{\"PauseBehavior\":\"0\",\"IdleBehavior\":\"0\",\"DefaultValueReg\":\"0\"},\"ch27\":{\"PauseBehavior\":\"0\",\"IdleBehavior\":\"0\",\"DefaultValueReg\":\"0\"},\"ch28\":{\"PauseBehavior\":\"0\",\"IdleBehavior\":\"0\",\"DefaultValueReg\":\"0\"},\"ch29\":{\"PauseBehavior\":\"0\",\"IdleBehavior\":\"0\",\"DefaultValueReg\":\"0\"},\"ch30\":{\"PauseBehavior\":\"0\",\"IdleBehavior\":\"0\",\"DefaultValueReg\":\"0\"},\"ch31\":{\"PauseBehavior\":\"0\",\"IdleBehavior\":\"0\",\"DefaultValueReg\":\"0\"}}}"  Slot_DV_6A="{\"dv_6A\":{\"ch0\":{\"PauseBehavior\":\"0\",\"IdleBehavior\":\"0\",\"DefaultValueReg\":\"0\"},\"ch1\":{\"PauseBehavior\":\"0\",\"IdleBehavior\":\"0\",\"DefaultValueReg\":\"0\"},\"ch2\":{\"PauseBehavior\":\"0\",\"IdleBehavior\":\"0\",\"DefaultValueReg\":\"0\"},\"ch3\":{\"PauseBehavior\":\"0\",\"IdleBehavior\":\"0\",\"DefaultValueReg\":\"0\"},\"ch4\":{\"PauseBehavior\":\"0\",\"IdleBehavior\":\"0\",\"DefaultValueReg\":\"0\"},\"ch5\":{\"PauseBehavior\":\"0\",\"IdleBehavior\":\"0\",\"DefaultValueReg\":\"0\"},\"ch6\":{\"PauseBehavior\":\"0\",\"IdleBehavior\":\"0\",\"DefaultValueReg\":\"0\"},\"ch7\":{\"PauseBehavior\":\"0\",\"IdleBehavior\":\"0\",\"DefaultValueReg\":\"0\"},\"ch8\":{\"PauseBehavior\":\"0\",\"IdleBehavior\":\"0\",\"DefaultValueReg\":\"0\"},\"ch9\":{\"PauseBehavior\":\"0\",\"IdleBehavior\":\"0\",\"DefaultValueReg\":\"0\"},\"ch10\":{\"PauseBehavior\":\"0\",\"IdleBehavior\":\"0\",\"DefaultValueReg\":\"0\"},\"ch11\":{\"PauseBehavior\":\"0\",\"IdleBehavior\":\"0\",\"DefaultValueReg\":\"0\"},\"ch12\":{\"PauseBehavior\":\"0\",\"IdleBehavior\":\"0\",\"DefaultValueReg\":\"0\"},\"ch13\":{\"PauseBehavior\":\"0\",\"IdleBehavior\":\"0\",\"DefaultValueReg\":\"0\"},\"ch14\":{\"PauseBehavior\":\"0\",\"IdleBehavior\":\"0\",\"DefaultValueReg\":\"0\"},\"ch15\":{\"PauseBehavior\":\"0\",\"IdleBehavior\":\"0\",\"DefaultValueReg\":\"0\"},\"ch16\":{\"PauseBehavior\":\"0\",\"IdleBehavior\":\"0\",\"DefaultValueReg\":\"0\"},\"ch17\":{\"PauseBehavior\":\"0\",\"IdleBehavior\":\"0\",\"DefaultValueReg\":\"0\"},\"ch18\":{\"PauseBehavior\":\"0\",\"IdleBehavior\":\"0\",\"DefaultValueReg\":\"0\"},\"ch19\":{\"PauseBehavior\":\"0\",\"IdleBehavior\":\"0\",\"DefaultValueReg\":\"0\"},\"ch20\":{\"PauseBehavior\":\"0\",\"IdleBehavior\":\"0\",\"DefaultValueReg\":\"0\"},\"ch21\":{\"PauseBehavior\":\"0\",\"IdleBehavior\":\"0\",\"DefaultValueReg\":\"0\"},\"ch22\":{\"PauseBehavior\":\"0\",\"IdleBehavior\":\"0\",\"DefaultValueReg\":\"0\"},\"ch23\":{\"PauseBehavior\":\"0\",\"IdleBehavior\":\"0\",\"DefaultValueReg\":\"0\"},\"ch24\":{\"PauseBehavior\":\"0\",\"IdleBehavior\":\"0\",\"DefaultValueReg\":\"0\"},\"ch25\":{\"PauseBehavior\":\"0\",\"IdleBehavior\":\"0\",\"DefaultValueReg\":\"0\"},\"ch26\":{\"PauseBehavior\":\"0\",\"IdleBehavior\":\"0\",\"DefaultValueReg\":\"0\"},\"ch27\":{\"PauseBehavior\":\"0\",\"IdleBehavior\":\"0\",\"DefaultValueReg\":\"0\"},\"ch28\":{\"PauseBehavior\":\"0\",\"IdleBehavior\":\"0\",\"DefaultValueReg\":\"0\"},\"ch29\":{\"PauseBehavior\":\"0\",\"IdleBehavior\":\"0\",\"DefaultValueReg\":\"0\"},\"ch30\":{\"PauseBehavior\":\"0\",\"IdleBehavior\":\"0\",\"DefaultValueReg\":\"0\"},\"ch31\":{\"PauseBehavior\":\"0\",\"IdleBehavior\":\"0\",\"DefaultValueReg\":\"0\"}}}"  Slot_DV_6B="{\"dv_6B\":{\"ch0\":{\"PauseBehavior\":\"0\",\"IdleBehavior\":\"0\",\"DefaultValueReg\":\"0\"},\"ch1\":{\"PauseBehavior\":\"0\",\"IdleBehavior\":\"0\",\"DefaultValueReg\":\"0\"},\"ch2\":{\"PauseBehavior\":\"0\",\"IdleBehavior\":\"0\",\"DefaultValueReg\":\"0\"},\"ch3\":{\"PauseBehavior\":\"0\",\"IdleBehavior\":\"0\",\"DefaultValueReg\":\"0\"},\"ch4\":{\"PauseBehavior\":\"0\",\"IdleBehavior\":\"0\",\"DefaultValueReg\":\"0\"},\"ch5\":{\"PauseBehavior\":\"0\",\"IdleBehavior\":\"0\",\"DefaultValueReg\":\"0\"},\"ch6\":{\"PauseBehavior\":\"0\",\"IdleBehavior\":\"0\",\"DefaultValueReg\":\"0\"},\"ch7\":{\"PauseBehavior\":\"0\",\"IdleBehavior\":\"0\",\"DefaultValueReg\":\"0\"},\"ch8\":{\"PauseBehavior\":\"0\",\"IdleBehavior\":\"0\",\"DefaultValueReg\":\"0\"},\"ch9\":{\"PauseBehavior\":\"0\",\"IdleBehavior\":\"0\",\"DefaultValueReg\":\"0\"},\"ch10\":{\"PauseBehavior\":\"0\",\"IdleBehavior\":\"0\",\"DefaultValueReg\":\"0\"},\"ch11\":{\"PauseBehavior\":\"0\",\"IdleBehavior\":\"0\",\"DefaultValueReg\":\"0\"},\"ch12\":{\"PauseBehavior\":\"0\",\"IdleBehavior\":\"0\",\"DefaultValueReg\":\"0\"},\"ch13\":{\"PauseBehavior\":\"0\",\"IdleBehavior\":\"0\",\"DefaultValueReg\":\"0\"},\"ch14\":{\"PauseBehavior\":\"0\",\"IdleBehavior\":\"0\",\"DefaultValueReg\":\"0\"},\"ch15\":{\"PauseBehavior\":\"0\",\"IdleBehavior\":\"0\",\"DefaultValueReg\":\"0\"},\"ch16\":{\"PauseBehavior\":\"0\",\"IdleBehavior\":\"0\",\"DefaultValueReg\":\"0\"},\"ch17\":{\"PauseBehavior\":\"0\",\"IdleBehavior\":\"0\",\"DefaultValueReg\":\"0\"},\"ch18\":{\"PauseBehavior\":\"0\",\"IdleBehavior\":\"0\",\"DefaultValueReg\":\"0\"},\"ch19\":{\"PauseBehavior\":\"0\",\"IdleBehavior\":\"0\",\"DefaultValueReg\":\"0\"},\"ch20\":{\"PauseBehavior\":\"0\",\"IdleBehavior\":\"0\",\"DefaultValueReg\":\"0\"},\"ch21\":{\"PauseBehavior\":\"0\",\"IdleBehavior\":\"0\",\"DefaultValueReg\":\"0\"},\"ch22\":{\"PauseBehavior\":\"0\",\"IdleBehavior\":\"0\",\"DefaultValueReg\":\"0\"},\"ch23\":{\"PauseBehavior\":\"0\",\"IdleBehavior\":\"0\",\"DefaultValueReg\":\"0\"},\"ch24\":{\"PauseBehavior\":\"0\",\"IdleBehavior\":\"0\",\"DefaultValueReg\":\"0\"},\"ch25\":{\"PauseBehavior\":\"0\",\"IdleBehavior\":\"0\",\"DefaultValueReg\":\"0\"},\"ch26\":{\"PauseBehavior\":\"0\",\"IdleBehavior\":\"0\",\"DefaultValueReg\":\"0\"},\"ch27\":{\"PauseBehavior\":\"0\",\"IdleBehavior\":\"0\",\"DefaultValueReg\":\"0\"},\"ch28\":{\"PauseBehavior\":\"0\",\"IdleBehavior\":\"0\",\"DefaultValueReg\":\"0\"},\"ch29\":{\"PauseBehavior\":\"0\",\"IdleBehavior\":\"0\",\"DefaultValueReg\":\"0\"},\"ch30\":{\"PauseBehavior\":\"0\",\"IdleBehavior\":\"0\",\"DefaultValueReg\":\"0\"},\"ch31\":{\"PauseBehavior\":\"0\",\"IdleBehavior\":\"0\",\"DefaultValueReg\":\"0\"}}}"  Expansion_DV_6A="{\"dv_Expansion_6A\":{\"ch0\":{\"PauseBehavior\":\"0\",\"IdleBehavior\":\"0\",\"DefaultValueReg\":\"0\"},\"ch1\":{\"PauseBehavior\":\"0\",\"IdleBehavior\":\"0\",\"DefaultValueReg\":\"0\"},\"ch2\":{\"PauseBehavior\":\"0\",\"IdleBehavior\":\"0\",\"DefaultValueReg\":\"0\"},\"ch3\":{\"PauseBehavior\":\"0\",\"IdleBehavior\":\"0\",\"DefaultValueReg\":\"0\"},\"ch4\":{\"PauseBehavior\":\"0\",\"IdleBehavior\":\"0\",\"DefaultValueReg\":\"0\"},\"ch5\":{\"PauseBehavior\":\"0\",\"IdleBehavior\":\"0\",\"DefaultValueReg\":\"0\"},\"ch6\":{\"PauseBehavior\":\"0\",\"IdleBehavior\":\"0\",\"DefaultValueReg\":\"0\"},\"ch7\":{\"PauseBehavior\":\"0\",\"IdleBehavior\":\"0\",\"DefaultValueReg\":\"0\"},\"ch8\":{\"PauseBehavior\":\"0\",\"IdleBehavior\":\"0\",\"DefaultValueReg\":\"0\"},\"ch9\":{\"PauseBehavior\":\"0\",\"IdleBehavior\":\"0\",\"DefaultValueReg\":\"0\"},\"ch10\":{\"PauseBehavior\":\"0\",\"IdleBehavior\":\"0\",\"DefaultValueReg\":\"0\"},\"ch11\":{\"PauseBehavior\":\"0\",\"IdleBehavior\":\"0\",\"DefaultValueReg\":\"0\"},\"ch12\":{\"PauseBehavior\":\"0\",\"IdleBehavior\":\"0\",\"DefaultValueReg\":\"0\"},\"ch13\":{\"PauseBehavior\":\"0\",\"IdleBehavior\":\"0\",\"DefaultValueReg\":\"0\"},\"ch14\":{\"PauseBehavior\":\"0\",\"IdleBehavior\":\"0\",\"DefaultValueReg\":\"0\"},\"ch15\":{\"PauseBehavior\":\"0\",\"IdleBehavior\":\"0\",\"DefaultValueReg\":\"0\"},\"ch16\":{\"PauseBehavior\":\"0\",\"IdleBehavior\":\"0\",\"DefaultValueReg\":\"0\"},\"ch17\":{\"PauseBehavior\":\"0\",\"IdleBehavior\":\"0\",\"DefaultValueReg\":\"0\"},\"ch18\":{\"PauseBehavior\":\"0\",\"IdleBehavior\":\"0\",\"DefaultValueReg\":\"0\"},\"ch19\":{\"PauseBehavior\":\"0\",\"IdleBehavior\":\"0\",\"DefaultValueReg\":\"0\"},\"ch20\":{\"PauseBehavior\":\"0\",\"IdleBehavior\":\"0\",\"DefaultValueReg\":\"0\"},\"ch21\":{\"PauseBehavior\":\"0\",\"IdleBehavior\":\"0\",\"DefaultValueReg\":\"0\"},\"ch22\":{\"PauseBehavior\":\"0\",\"IdleBehavior\":\"0\",\"DefaultValueReg\":\"0\"},\"ch23\":{\"PauseBehavior\":\"0\",\"IdleBehavior\":\"0\",\"DefaultValueReg\":\"0\"},\"ch24\":{\"PauseBehavior\":\"0\",\"IdleBehavior\":\"0\",\"DefaultValueReg\":\"0\"},\"ch25\":{\"PauseBehavior\":\"0\",\"IdleBehavior\":\"0\",\"DefaultValueReg\":\"0\"},\"ch26\":{\"PauseBehavior\":\"0\",\"IdleBehavior\":\"0\",\"DefaultValueReg\":\"0\"},\"ch27\":{\"PauseBehavior\":\"0\",\"IdleBehavior\":\"0\",\"DefaultValueReg\":\"0\"},\"ch28\":{\"PauseBehavior\":\"0\",\"IdleBehavior\":\"0\",\"DefaultValueReg\":\"0\"},\"ch29\":{\"PauseBehavior\":\"0\",\"IdleBehavior\":\"0\",\"DefaultValueReg\":\"0\"},\"ch30\":{\"PauseBehavior\":\"0\",\"IdleBehavior\":\"0\",\"DefaultValueReg\":\"0\"},\"ch31\":{\"PauseBehavior\":\"0\",\"IdleBehavior\":\"0\",\"DefaultValueReg\":\"0\"}}}"  Expansion_DV_6B="{\"dv_Expansion_6B\":{\"ch0\":{\"PauseBehavior\":\"0\",\"IdleBehavior\":\"0\",\"DefaultValueReg\":\"0\"},\"ch1\":{\"PauseBehavior\":\"0\",\"IdleBehavior\":\"0\",\"DefaultValueReg\":\"0\"},\"ch2\":{\"PauseBehavior\":\"0\",\"IdleBehavior\":\"0\",\"DefaultValueReg\":\"0\"},\"ch3\":{\"PauseBehavior\":\"0\",\"IdleBehavior\":\"0\",\"DefaultValueReg\":\"0\"},\"ch4\":{\"PauseBehavior\":\"0\",\"IdleBehavior\":\"0\",\"DefaultValueReg\":\"0\"},\"ch5\":{\"PauseBehavior\":\"0\",\"IdleBehavior\":\"0\",\"DefaultValueReg\":\"0\"},\"ch6\":{\"PauseBehavior\":\"0\",\"IdleBehavior\":\"0\",\"DefaultValueReg\":\"0\"},\"ch7\":{\"PauseBehavior\":\"0\",\"IdleBehavior\":\"0\",\"DefaultValueReg\":\"0\"},\"ch8\":{\"PauseBehavior\":\"0\",\"IdleBehavior\":\"0\",\"DefaultValueReg\":\"0\"},\"ch9\":{\"PauseBehavior\":\"0\",\"IdleBehavior\":\"0\",\"DefaultValueReg\":\"0\"},\"ch10\":{\"PauseBehavior\":\"0\",\"IdleBehavior\":\"0\",\"DefaultValueReg\":\"0\"},\"ch11\":{\"PauseBehavior\":\"0\",\"IdleBehavior\":\"0\",\"DefaultValueReg\":\"0\"},\"ch12\":{\"PauseBehavior\":\"0\",\"IdleBehavior\":\"0\",\"DefaultValueReg\":\"0\"},\"ch13\":{\"PauseBehavior\":\"0\",\"IdleBehavior\":\"0\",\"DefaultValueReg\":\"0\"},\"ch14\":{\"PauseBehavior\":\"0\",\"IdleBehavior\":\"0\",\"DefaultValueReg\":\"0\"},\"ch15\":{\"PauseBehavior\":\"0\",\"IdleBehavior\":\"0\",\"DefaultValueReg\":\"0\"},\"ch16\":{\"PauseBehavior\":\"0\",\"IdleBehavior\":\"0\",\"DefaultValueReg\":\"0\"},\"ch17\":{\"PauseBehavior\":\"0\",\"IdleBehavior\":\"0\",\"DefaultValueReg\":\"0\"},\"ch18\":{\"PauseBehavior\":\"0\",\"IdleBehavior\":\"0\",\"DefaultValueReg\":\"0\"},\"ch19\":{\"PauseBehavior\":\"0\",\"IdleBehavior\":\"0\",\"DefaultValueReg\":\"0\"},\"ch20\":{\"PauseBehavior\":\"0\",\"IdleBehavior\":\"0\",\"DefaultValueReg\":\"0\"},\"ch21\":{\"PauseBehavior\":\"0\",\"IdleBehavior\":\"0\",\"DefaultValueReg\":\"0\"},\"ch22\":{\"PauseBehavior\":\"0\",\"IdleBehavior\":\"0\",\"DefaultValueReg\":\"0\"},\"ch23\":{\"PauseBehavior\":\"0\",\"IdleBehavior\":\"0\",\"DefaultValueReg\":\"0\"},\"ch24\":{\"PauseBehavior\":\"0\",\"IdleBehavior\":\"0\",\"DefaultValueReg\":\"0\"},\"ch25\":{\"PauseBehavior\":\"0\",\"IdleBehavior\":\"0\",\"DefaultValueReg\":\"0\"},\"ch26\":{\"PauseBehavior\":\"0\",\"IdleBehavior\":\"0\",\"DefaultValueReg\":\"0\"},\"ch27\":{\"PauseBehavior\":\"0\",\"IdleBehavior\":\"0\",\"DefaultValueReg\":\"0\"},\"ch28\":{\"PauseBehavior\":\"0\",\"IdleBehavior\":\"0\",\"DefaultValueReg\":\"0\"},\"ch29\":{\"PauseBehavior\":\"0\",\"IdleBehavior\":\"0\",\"DefaultValueReg\":\"0\"},\"ch30\":{\"PauseBehavior\":\"0\",\"IdleBehavior\":\"0\",\"DefaultValueReg\":\"0\"},\"ch31\":{\"PauseBehavior\":\"0\",\"IdleBehavior\":\"0\",\"DefaultValueReg\":\"0\"}}}"  Slot_DV_5A="{\"dv_5A\":{\"ch0\":{\"PauseBehavior\":\"0\",\"IdleBehavior\":\"0\",\"DefaultValueReg\":\"0\"},\"ch1\":{\"PauseBehavior\":\"0\",\"IdleBehavior\":\"0\",\"DefaultValueReg\":\"0\"},\"ch2\":{\"PauseBehavior\":\"0\",\"IdleBehavior\":\"0\",\"DefaultValueReg\":\"0\"},\"ch3\":{\"PauseBehavior\":\"0\",\"IdleBehavior\":\"0\",\"DefaultValueReg\":\"0\"},\"ch4\":{\"PauseBehavior\":\"0\",\"IdleBehavior\":\"0\",\"DefaultValueReg\":\"0\"},\"ch5\":{\"PauseBehavior\":\"0\",\"IdleBehavior\":\"0\",\"DefaultValueReg\":\"0\"},\"ch6\":{\"PauseBehavior\":\"0\",\"IdleBehavior\":\"0\",\"DefaultValueReg\":\"0\"},\"ch7\":{\"PauseBehavior\":\"0\",\"IdleBehavior\":\"0\",\"DefaultValueReg\":\"0\"},\"ch8\":{\"PauseBehavior\":\"0\",\"IdleBehavior\":\"0\",\"DefaultValueReg\":\"0\"},\"ch9\":{\"PauseBehavior\":\"0\",\"IdleBehavior\":\"0\",\"DefaultValueReg\":\"0\"},\"ch10\":{\"PauseBehavior\":\"0\",\"IdleBehavior\":\"0\",\"DefaultValueReg\":\"0\"},\"ch11\":{\"PauseBehavior\":\"0\",\"IdleBehavior\":\"0\",\"DefaultValueReg\":\"0\"},\"ch12\":{\"PauseBehavior\":\"0\",\"IdleBehavior\":\"0\",\"DefaultValueReg\":\"0\"},\"ch13\":{\"PauseBehavior\":\"0\",\"IdleBehavior\":\"0\",\"DefaultValueReg\":\"0\"},\"ch14\":{\"PauseBehavior\":\"0\",\"IdleBehavior\":\"0\",\"DefaultValueReg\":\"0\"},\"ch15\":{\"PauseBehavior\":\"0\",\"IdleBehavior\":\"0\",\"DefaultValueReg\":\"0\"},\"ch16\":{\"PauseBehavior\":\"0\",\"IdleBehavior\":\"0\",\"DefaultValueReg\":\"0\"},\"ch17\":{\"PauseBehavior\":\"0\",\"IdleBehavior\":\"0\",\"DefaultValueReg\":\"0\"},\"ch18\":{\"PauseBehavior\":\"0\",\"IdleBehavior\":\"0\",\"DefaultValueReg\":\"0\"},\"ch19\":{\"PauseBehavior\":\"0\",\"IdleBehavior\":\"0\",\"DefaultValueReg\":\"0\"},\"ch20\":{\"PauseBehavior\":\"0\",\"IdleBehavior\":\"0\",\"DefaultValueReg\":\"0\"},\"ch21\":{\"PauseBehavior\":\"0\",\"IdleBehavior\":\"0\",\"DefaultValueReg\":\"0\"},\"ch22\":{\"PauseBehavior\":\"0\",\"IdleBehavior\":\"0\",\"DefaultValueReg\":\"0\"},\"ch23\":{\"PauseBehavior\":\"0\",\"IdleBehavior\":\"0\",\"DefaultValueReg\":\"0\"},\"ch24\":{\"PauseBehavior\":\"0\",\"IdleBehavior\":\"0\",\"DefaultValueReg\":\"0\"},\"ch25\":{\"PauseBehavior\":\"0\",\"IdleBehavior\":\"0\",\"DefaultValueReg\":\"0\"},\"ch26\":{\"PauseBehavior\":\"0\",\"IdleBehavior\":\"0\",\"DefaultValueReg\":\"0\"},\"ch27\":{\"PauseBehavior\":\"0\",\"IdleBehavior\":\"0\",\"DefaultValueReg\":\"0\"},\"ch28\":{\"PauseBehavior\":\"0\",\"IdleBehavior\":\"0\",\"DefaultValueReg\":\"0\"},\"ch29\":{\"PauseBehavior\":\"0\",\"IdleBehavior\":\"0\",\"DefaultValueReg\":\"0\"},\"ch30\":{\"PauseBehavior\":\"0\",\"IdleBehavior\":\"0\",\"DefaultValueReg\":\"0\"},\"ch31\":{\"PauseBehavior\":\"0\",\"IdleBehavior\":\"0\",\"DefaultValueReg\":\"0\"}}}"  Slot_DV_5B="{\"dv_5B\":{\"ch0\":{\"PauseBehavior\":\"0\",\"IdleBehavior\":\"0\",\"DefaultValueReg\":\"0\"},\"ch1\":{\"PauseBehavior\":\"0\",\"IdleBehavior\":\"0\",\"DefaultValueReg\":\"0\"},\"ch2\":{\"PauseBehavior\":\"0\",\"IdleBehavior\":\"0\",\"DefaultValueReg\":\"0\"},\"ch3\":{\"PauseBehavior\":\"0\",\"IdleBehavior\":\"0\",\"DefaultValueReg\":\"0\"},\"ch4\":{\"PauseBehavior\":\"0\",\"IdleBehavior\":\"0\",\"DefaultValueReg\":\"0\"},\"ch5\":{\"PauseBehavior\":\"0\",\"IdleBehavior\":\"0\",\"DefaultValueReg\":\"0\"},\"ch6\":{\"PauseBehavior\":\"0\",\"IdleBehavior\":\"0\",\"DefaultValueReg\":\"0\"},\"ch7\":{\"PauseBehavior\":\"0\",\"IdleBehavior\":\"0\",\"DefaultValueReg\":\"0\"},\"ch8\":{\"PauseBehavior\":\"0\",\"IdleBehavior\":\"0\",\"DefaultValueReg\":\"0\"},\"ch9\":{\"PauseBehavior\":\"0\",\"IdleBehavior\":\"0\",\"DefaultValueReg\":\"0\"},\"ch10\":{\"PauseBehavior\":\"0\",\"IdleBehavior\":\"0\",\"DefaultValueReg\":\"0\"},\"ch11\":{\"PauseBehavior\":\"0\",\"IdleBehavior\":\"0\",\"DefaultValueReg\":\"0\"},\"ch12\":{\"PauseBehavior\":\"0\",\"IdleBehavior\":\"0\",\"DefaultValueReg\":\"0\"},\"ch13\":{\"PauseBehavior\":\"0\",\"IdleBehavior\":\"0\",\"DefaultValueReg\":\"0\"},\"ch14\":{\"PauseBehavior\":\"0\",\"IdleBehavior\":\"0\",\"DefaultValueReg\":\"0\"},\"ch15\":{\"PauseBehavior\":\"0\",\"IdleBehavior\":\"0\",\"DefaultValueReg\":\"0\"},\"ch16\":{\"PauseBehavior\":\"0\",\"IdleBehavior\":\"0\",\"DefaultValueReg\":\"0\"},\"ch17\":{\"PauseBehavior\":\"0\",\"IdleBehavior\":\"0\",\"DefaultValueReg\":\"0\"},\"ch18\":{\"PauseBehavior\":\"0\",\"IdleBehavior\":\"0\",\"DefaultValueReg\":\"0\"},\"ch19\":{\"PauseBehavior\":\"0\",\"IdleBehavior\":\"0\",\"DefaultValueReg\":\"0\"},\"ch20\":{\"PauseBehavior\":\"0\",\"IdleBehavior\":\"0\",\"DefaultValueReg\":\"0\"},\"ch21\":{\"PauseBehavior\":\"0\",\"IdleBehavior\":\"0\",\"DefaultValueReg\":\"0\"},\"ch22\":{\"PauseBehavior\":\"0\",\"IdleBehavior\":\"0\",\"DefaultValueReg\":\"0\"},\"ch23\":{\"PauseBehavior\":\"0\",\"IdleBehavior\":\"0\",\"DefaultValueReg\":\"0\"},\"ch24\":{\"PauseBehavior\":\"0\",\"IdleBehavior\":\"0\",\"DefaultValueReg\":\"0\"},\"ch25\":{\"PauseBehavior\":\"0\",\"IdleBehavior\":\"0\",\"DefaultValueReg\":\"0\"},\"ch26\":{\"PauseBehavior\":\"0\",\"IdleBehavior\":\"0\",\"DefaultValueReg\":\"0\"},\"ch27\":{\"PauseBehavior\":\"0\",\"IdleBehavior\":\"0\",\"DefaultValueReg\":\"0\"},\"ch28\":{\"PauseBehavior\":\"0\",\"IdleBehavior\":\"0\",\"DefaultValueReg\":\"0\"},\"ch29\":{\"PauseBehavior\":\"0\",\"IdleBehavior\":\"0\",\"DefaultValueReg\":\"0\"},\"ch30\":{\"PauseBehavior\":\"0\",\"IdleBehavior\":\"0\",\"DefaultValueReg\":\"0\"},\"ch31\":{\"PauseBehavior\":\"0\",\"IdleBehavior\":\"0\",\"DefaultValueReg\":\"0\"}}}"  Expansion_DV_5A="{\"dv_Expansion_5A\":{\"ch0\":{\"PauseBehavior\":\"0\",\"IdleBehavior\":\"0\",\"DefaultValueReg\":\"0\"},\"ch1\":{\"PauseBehavior\":\"0\",\"IdleBehavior\":\"0\",\"DefaultValueReg\":\"0\"},\"ch2\":{\"PauseBehavior\":\"0\",\"IdleBehavior\":\"0\",\"DefaultValueReg\":\"0\"},\"ch3\":{\"PauseBehavior\":\"0\",\"IdleBehavior\":\"0\",\"DefaultValueReg\":\"0\"},\"ch4\":{\"PauseBehavior\":\"0\",\"IdleBehavior\":\"0\",\"DefaultValueReg\":\"0\"},\"ch5\":{\"PauseBehavior\":\"0\",\"IdleBehavior\":\"0\",\"DefaultValueReg\":\"0\"},\"ch6\":{\"PauseBehavior\":\"0\",\"IdleBehavior\":\"0\",\"DefaultValueReg\":\"0\"},\"ch7\":{\"PauseBehavior\":\"0\",\"IdleBehavior\":\"0\",\"DefaultValueReg\":\"0\"},\"ch8\":{\"PauseBehavior\":\"0\",\"IdleBehavior\":\"0\",\"DefaultValueReg\":\"0\"},\"ch9\":{\"PauseBehavior\":\"0\",\"IdleBehavior\":\"0\",\"DefaultValueReg\":\"0\"},\"ch10\":{\"PauseBehavior\":\"0\",\"IdleBehavior\":\"0\",\"DefaultValueReg\":\"0\"},\"ch11\":{\"PauseBehavior\":\"0\",\"IdleBehavior\":\"0\",\"DefaultValueReg\":\"0\"},\"ch12\":{\"PauseBehavior\":\"0\",\"IdleBehavior\":\"0\",\"DefaultValueReg\":\"0\"},\"ch13\":{\"PauseBehavior\":\"0\",\"IdleBehavior\":\"0\",\"DefaultValueReg\":\"0\"},\"ch14\":{\"PauseBehavior\":\"0\",\"IdleBehavior\":\"0\",\"DefaultValueReg\":\"0\"},\"ch15\":{\"PauseBehavior\":\"0\",\"IdleBehavior\":\"0\",\"DefaultValueReg\":\"0\"},\"ch16\":{\"PauseBehavior\":\"0\",\"IdleBehavior\":\"0\",\"DefaultValueReg\":\"0\"},\"ch17\":{\"PauseBehavior\":\"0\",\"IdleBehavior\":\"0\",\"DefaultValueReg\":\"0\"},\"ch18\":{\"PauseBehavior\":\"0\",\"IdleBehavior\":\"0\",\"DefaultValueReg\":\"0\"},\"ch19\":{\"PauseBehavior\":\"0\",\"IdleBehavior\":\"0\",\"DefaultValueReg\":\"0\"},\"ch20\":{\"PauseBehavior\":\"0\",\"IdleBehavior\":\"0\",\"DefaultValueReg\":\"0\"},\"ch21\":{\"PauseBehavior\":\"0\",\"IdleBehavior\":\"0\",\"DefaultValueReg\":\"0\"},\"ch22\":{\"PauseBehavior\":\"0\",\"IdleBehavior\":\"0\",\"DefaultValueReg\":\"0\"},\"ch23\":{\"PauseBehavior\":\"0\",\"IdleBehavior\":\"0\",\"DefaultValueReg\":\"0\"},\"ch24\":{\"PauseBehavior\":\"0\",\"IdleBehavior\":\"0\",\"DefaultValueReg\":\"0\"},\"ch25\":{\"PauseBehavior\":\"0\",\"IdleBehavior\":\"0\",\"DefaultValueReg\":\"0\"},\"ch26\":{\"PauseBehavior\":\"0\",\"IdleBehavior\":\"0\",\"DefaultValueReg\":\"0\"},\"ch27\":{\"PauseBehavior\":\"0\",\"IdleBehavior\":\"0\",\"DefaultValueReg\":\"0\"},\"ch28\":{\"PauseBehavior\":\"0\",\"IdleBehavior\":\"0\",\"DefaultValueReg\":\"0\"},\"ch29\":{\"PauseBehavior\":\"0\",\"IdleBehavior\":\"0\",\"DefaultValueReg\":\"0\"},\"ch30\":{\"PauseBehavior\":\"0\",\"IdleBehavior\":\"0\",\"DefaultValueReg\":\"0\"},\"ch31\":{\"PauseBehavior\":\"0\",\"IdleBehavior\":\"0\",\"DefaultValueReg\":\"0\"}}}"  Expansion_DV_5B="{\"dv_Expansion_5B\":{\"ch0\":{\"PauseBehavior\":\"0\",\"IdleBehavior\":\"0\",\"DefaultValueReg\":\"0\"},\"ch1\":{\"PauseBehavior\":\"0\",\"IdleBehavior\":\"0\",\"DefaultValueReg\":\"0\"},\"ch2\":{\"PauseBehavior\":\"0\",\"IdleBehavior\":\"0\",\"DefaultValueReg\":\"0\"},\"ch3\":{\"PauseBehavior\":\"0\",\"IdleBehavior\":\"0\",\"DefaultValueReg\":\"0\"},\"ch4\":{\"PauseBehavior\":\"0\",\"IdleBehavior\":\"0\",\"DefaultValueReg\":\"0\"},\"ch5\":{\"PauseBehavior\":\"0\",\"IdleBehavior\":\"0\",\"DefaultValueReg\":\"0\"},\"ch6\":{\"PauseBehavior\":\"0\",\"IdleBehavior\":\"0\",\"DefaultValueReg\":\"0\"},\"ch7\":{\"PauseBehavior\":\"0\",\"IdleBehavior\":\"0\",\"DefaultValueReg\":\"0\"},\"ch8\":{\"PauseBehavior\":\"0\",\"IdleBehavior\":\"0\",\"DefaultValueReg\":\"0\"},\"ch9\":{\"PauseBehavior\":\"0\",\"IdleBehavior\":\"0\",\"DefaultValueReg\":\"0\"},\"ch10\":{\"PauseBehavior\":\"0\",\"IdleBehavior\":\"0\",\"DefaultValueReg\":\"0\"},\"ch11\":{\"PauseBehavior\":\"0\",\"IdleBehavior\":\"0\",\"DefaultValueReg\":\"0\"},\"ch12\":{\"PauseBehavior\":\"0\",\"IdleBehavior\":\"0\",\"DefaultValueReg\":\"0\"},\"ch13\":{\"PauseBehavior\":\"0\",\"IdleBehavior\":\"0\",\"DefaultValueReg\":\"0\"},\"ch14\":{\"PauseBehavior\":\"0\",\"IdleBehavior\":\"0\",\"DefaultValueReg\":\"0\"},\"ch15\":{\"PauseBehavior\":\"0\",\"IdleBehavior\":\"0\",\"DefaultValueReg\":\"0\"},\"ch16\":{\"PauseBehavior\":\"0\",\"IdleBehavior\":\"0\",\"DefaultValueReg\":\"0\"},\"ch17\":{\"PauseBehavior\":\"0\",\"IdleBehavior\":\"0\",\"DefaultValueReg\":\"0\"},\"ch18\":{\"PauseBehavior\":\"0\",\"IdleBehavior\":\"0\",\"DefaultValueReg\":\"0\"},\"ch19\":{\"PauseBehavior\":\"0\",\"IdleBehavior\":\"0\",\"DefaultValueReg\":\"0\"},\"ch20\":{\"PauseBehavior\":\"0\",\"IdleBehavior\":\"0\",\"DefaultValueReg\":\"0\"},\"ch21\":{\"PauseBehavior\":\"0\",\"IdleBehavior\":\"0\",\"DefaultValueReg\":\"0\"},\"ch22\":{\"PauseBehavior\":\"0\",\"IdleBehavior\":\"0\",\"DefaultValueReg\":\"0\"},\"ch23\":{\"PauseBehavior\":\"0\",\"IdleBehavior\":\"0\",\"DefaultValueReg\":\"0\"},\"ch24\":{\"PauseBehavior\":\"0\",\"IdleBehavior\":\"0\",\"DefaultValueReg\":\"0\"},\"ch25\":{\"PauseBehavior\":\"0\",\"IdleBehavior\":\"0\",\"DefaultValueReg\":\"0\"},\"ch26\":{\"PauseBehavior\":\"0\",\"IdleBehavior\":\"0\",\"DefaultValueReg\":\"0\"},\"ch27\":{\"PauseBehavior\":\"0\",\"IdleBehavior\":\"0\",\"DefaultValueReg\":\"0\"},\"ch28\":{\"PauseBehavior\":\"0\",\"IdleBehavior\":\"0\",\"DefaultValueReg\":\"0\"},\"ch29\":{\"PauseBehavior\":\"0\",\"IdleBehavior\":\"0\",\"DefaultValueReg\":\"0\"},\"ch30\":{\"PauseBehavior\":\"0\",\"IdleBehavior\":\"0\",\"DefaultValueReg\":\"0\"},\"ch31\":{\"PauseBehavior\":\"0\",\"IdleBehavior\":\"0\",\"DefaultValueReg\":\"0\"}}}"  Slot_DV_4A="{\"dv_4A\":{\"ch0\":{\"PauseBehavior\":\"0\",\"IdleBehavior\":\"0\",\"DefaultValueReg\":\"0\"},\"ch1\":{\"PauseBehavior\":\"0\",\"IdleBehavior\":\"0\",\"DefaultValueReg\":\"0\"},\"ch2\":{\"PauseBehavior\":\"0\",\"IdleBehavior\":\"0\",\"DefaultValueReg\":\"0\"},\"ch3\":{\"PauseBehavior\":\"0\",\"IdleBehavior\":\"0\",\"DefaultValueReg\":\"0\"},\"ch4\":{\"PauseBehavior\":\"0\",\"IdleBehavior\":\"0\",\"DefaultValueReg\":\"0\"},\"ch5\":{\"PauseBehavior\":\"0\",\"IdleBehavior\":\"0\",\"DefaultValueReg\":\"0\"},\"ch6\":{\"PauseBehavior\":\"0\",\"IdleBehavior\":\"0\",\"DefaultValueReg\":\"0\"},\"ch7\":{\"PauseBehavior\":\"0\",\"IdleBehavior\":\"0\",\"DefaultValueReg\":\"0\"},\"ch8\":{\"PauseBehavior\":\"0\",\"IdleBehavior\":\"0\",\"DefaultValueReg\":\"0\"},\"ch9\":{\"PauseBehavior\":\"0\",\"IdleBehavior\":\"0\",\"DefaultValueReg\":\"0\"},\"ch10\":{\"PauseBehavior\":\"0\",\"IdleBehavior\":\"0\",\"DefaultValueReg\":\"0\"},\"ch11\":{\"PauseBehavior\":\"0\",\"IdleBehavior\":\"0\",\"DefaultValueReg\":\"0\"},\"ch12\":{\"PauseBehavior\":\"0\",\"IdleBehavior\":\"0\",\"DefaultValueReg\":\"0\"},\"ch13\":{\"PauseBehavior\":\"0\",\"IdleBehavior\":\"0\",\"DefaultValueReg\":\"0\"},\"ch14\":{\"PauseBehavior\":\"0\",\"IdleBehavior\":\"0\",\"DefaultValueReg\":\"0\"},\"ch15\":{\"PauseBehavior\":\"0\",\"IdleBehavior\":\"0\",\"DefaultValueReg\":\"0\"},\"ch16\":{\"PauseBehavior\":\"0\",\"IdleBehavior\":\"0\",\"DefaultValueReg\":\"0\"},\"ch17\":{\"PauseBehavior\":\"0\",\"IdleBehavior\":\"0\",\"DefaultValueReg\":\"0\"},\"ch18\":{\"PauseBehavior\":\"0\",\"IdleBehavior\":\"0\",\"DefaultValueReg\":\"0\"},\"ch19\":{\"PauseBehavior\":\"0\",\"IdleBehavior\":\"0\",\"DefaultValueReg\":\"0\"},\"ch20\":{\"PauseBehavior\":\"0\",\"IdleBehavior\":\"0\",\"DefaultValueReg\":\"0\"},\"ch21\":{\"PauseBehavior\":\"0\",\"IdleBehavior\":\"0\",\"DefaultValueReg\":\"0\"},\"ch22\":{\"PauseBehavior\":\"0\",\"IdleBehavior\":\"0\",\"DefaultValueReg\":\"0\"},\"ch23\":{\"PauseBehavior\":\"0\",\"IdleBehavior\":\"0\",\"DefaultValueReg\":\"0\"},\"ch24\":{\"PauseBehavior\":\"0\",\"IdleBehavior\":\"0\",\"DefaultValueReg\":\"0\"},\"ch25\":{\"PauseBehavior\":\"0\",\"IdleBehavior\":\"0\",\"DefaultValueReg\":\"0\"},\"ch26\":{\"PauseBehavior\":\"0\",\"IdleBehavior\":\"0\",\"DefaultValueReg\":\"0\"},\"ch27\":{\"PauseBehavior\":\"0\",\"IdleBehavior\":\"0\",\"DefaultValueReg\":\"0\"},\"ch28\":{\"PauseBehavior\":\"0\",\"IdleBehavior\":\"0\",\"DefaultValueReg\":\"0\"},\"ch29\":{\"PauseBehavior\":\"0\",\"IdleBehavior\":\"0\",\"DefaultValueReg\":\"0\"},\"ch30\":{\"PauseBehavior\":\"0\",\"IdleBehavior\":\"0\",\"DefaultValueReg\":\"0\"},\"ch31\":{\"PauseBehavior\":\"0\",\"IdleBehavior\":\"0\",\"DefaultValueReg\":\"0\"}}}"  Slot_DV_4B="{\"dv_4B\":{\"ch0\":{\"PauseBehavior\":\"0\",\"IdleBehavior\":\"0\",\"DefaultValueReg\":\"0\"},\"ch1\":{\"PauseBehavior\":\"0\",\"IdleBehavior\":\"0\",\"DefaultValueReg\":\"0\"},\"ch2\":{\"PauseBehavior\":\"0\",\"IdleBehavior\":\"0\",\"DefaultValueReg\":\"0\"},\"ch3\":{\"PauseBehavior\":\"0\",\"IdleBehavior\":\"0\",\"DefaultValueReg\":\"0\"},\"ch4\":{\"PauseBehavior\":\"0\",\"IdleBehavior\":\"0\",\"DefaultValueReg\":\"0\"},\"ch5\":{\"PauseBehavior\":\"0\",\"IdleBehavior\":\"0\",\"DefaultValueReg\":\"0\"},\"ch6\":{\"PauseBehavior\":\"0\",\"IdleBehavior\":\"0\",\"DefaultValueReg\":\"0\"},\"ch7\":{\"PauseBehavior\":\"0\",\"IdleBehavior\":\"0\",\"DefaultValueReg\":\"0\"},\"ch8\":{\"PauseBehavior\":\"0\",\"IdleBehavior\":\"0\",\"DefaultValueReg\":\"0\"},\"ch9\":{\"PauseBehavior\":\"0\",\"IdleBehavior\":\"0\",\"DefaultValueReg\":\"0\"},\"ch10\":{\"PauseBehavior\":\"0\",\"IdleBehavior\":\"0\",\"DefaultValueReg\":\"0\"},\"ch11\":{\"PauseBehavior\":\"0\",\"IdleBehavior\":\"0\",\"DefaultValueReg\":\"0\"},\"ch12\":{\"PauseBehavior\":\"0\",\"IdleBehavior\":\"0\",\"DefaultValueReg\":\"0\"},\"ch13\":{\"PauseBehavior\":\"0\",\"IdleBehavior\":\"0\",\"DefaultValueReg\":\"0\"},\"ch14\":{\"PauseBehavior\":\"0\",\"IdleBehavior\":\"0\",\"DefaultValueReg\":\"0\"},\"ch15\":{\"PauseBehavior\":\"0\",\"IdleBehavior\":\"0\",\"DefaultValueReg\":\"0\"},\"ch16\":{\"PauseBehavior\":\"0\",\"IdleBehavior\":\"0\",\"DefaultValueReg\":\"0\"},\"ch17\":{\"PauseBehavior\":\"0\",\"IdleBehavior\":\"0\",\"DefaultValueReg\":\"0\"},\"ch18\":{\"PauseBehavior\":\"0\",\"IdleBehavior\":\"0\",\"DefaultValueReg\":\"0\"},\"ch19\":{\"PauseBehavior\":\"0\",\"IdleBehavior\":\"0\",\"DefaultValueReg\":\"0\"},\"ch20\":{\"PauseBehavior\":\"0\",\"IdleBehavior\":\"0\",\"DefaultValueReg\":\"0\"},\"ch21\":{\"PauseBehavior\":\"0\",\"IdleBehavior\":\"0\",\"DefaultValueReg\":\"0\"},\"ch22\":{\"PauseBehavior\":\"0\",\"IdleBehavior\":\"0\",\"DefaultValueReg\":\"0\"},\"ch23\":{\"PauseBehavior\":\"0\",\"IdleBehavior\":\"0\",\"DefaultValueReg\":\"0\"},\"ch24\":{\"PauseBehavior\":\"0\",\"IdleBehavior\":\"0\",\"DefaultValueReg\":\"0\"},\"ch25\":{\"PauseBehavior\":\"0\",\"IdleBehavior\":\"0\",\"DefaultValueReg\":\"0\"},\"ch26\":{\"PauseBehavior\":\"0\",\"IdleBehavior\":\"0\",\"DefaultValueReg\":\"0\"},\"ch27\":{\"PauseBehavior\":\"0\",\"IdleBehavior\":\"0\",\"DefaultValueReg\":\"0\"},\"ch28\":{\"PauseBehavior\":\"0\",\"IdleBehavior\":\"0\",\"DefaultValueReg\":\"0\"},\"ch29\":{\"PauseBehavior\":\"0\",\"IdleBehavior\":\"0\",\"DefaultValueReg\":\"0\"},\"ch30\":{\"PauseBehavior\":\"0\",\"IdleBehavior\":\"0\",\"DefaultValueReg\":\"0\"},\"ch31\":{\"PauseBehavior\":\"0\",\"IdleBehavior\":\"0\",\"DefaultValueReg\":\"0\"}}}"  Expansion_DV_4A="{\"dv_Expansion_4A\":{\"ch0\":{\"PauseBehavior\":\"0\",\"IdleBehavior\":\"0\",\"DefaultValueReg\":\"0\"},\"ch1\":{\"PauseBehavior\":\"0\",\"IdleBehavior\":\"0\",\"DefaultValueReg\":\"0\"},\"ch2\":{\"PauseBehavior\":\"0\",\"IdleBehavior\":\"0\",\"DefaultValueReg\":\"0\"},\"ch3\":{\"PauseBehavior\":\"0\",\"IdleBehavior\":\"0\",\"DefaultValueReg\":\"0\"},\"ch4\":{\"PauseBehavior\":\"0\",\"IdleBehavior\":\"0\",\"DefaultValueReg\":\"0\"},\"ch5\":{\"PauseBehavior\":\"0\",\"IdleBehavior\":\"0\",\"DefaultValueReg\":\"0\"},\"ch6\":{\"PauseBehavior\":\"0\",\"IdleBehavior\":\"0\",\"DefaultValueReg\":\"0\"},\"ch7\":{\"PauseBehavior\":\"0\",\"IdleBehavior\":\"0\",\"DefaultValueReg\":\"0\"},\"ch8\":{\"PauseBehavior\":\"0\",\"IdleBehavior\":\"0\",\"DefaultValueReg\":\"0\"},\"ch9\":{\"PauseBehavior\":\"0\",\"IdleBehavior\":\"0\",\"DefaultValueReg\":\"0\"},\"ch10\":{\"PauseBehavior\":\"0\",\"IdleBehavior\":\"0\",\"DefaultValueReg\":\"0\"},\"ch11\":{\"PauseBehavior\":\"0\",\"IdleBehavior\":\"0\",\"DefaultValueReg\":\"0\"},\"ch12\":{\"PauseBehavior\":\"0\",\"IdleBehavior\":\"0\",\"DefaultValueReg\":\"0\"},\"ch13\":{\"PauseBehavior\":\"0\",\"IdleBehavior\":\"0\",\"DefaultValueReg\":\"0\"},\"ch14\":{\"PauseBehavior\":\"0\",\"IdleBehavior\":\"0\",\"DefaultValueReg\":\"0\"},\"ch15\":{\"PauseBehavior\":\"0\",\"IdleBehavior\":\"0\",\"DefaultValueReg\":\"0\"},\"ch16\":{\"PauseBehavior\":\"0\",\"IdleBehavior\":\"0\",\"DefaultValueReg\":\"0\"},\"ch17\":{\"PauseBehavior\":\"0\",\"IdleBehavior\":\"0\",\"DefaultValueReg\":\"0\"},\"ch18\":{\"PauseBehavior\":\"0\",\"IdleBehavior\":\"0\",\"DefaultValueReg\":\"0\"},